simulink model "DYN_02x"  (R2021a)
(part 5 of 53)

[de2*((cos(e6)*(sin(e2 + e3)*sin(e5) - cos(e2 + e3)*cos(e4)*cos(e5)) + cos(e2 + e3)*sin(e4)*sin(e6))*(I6zx*(cos(e2 + e3)*cos(e5) - sin(e2 + e3)*cos(e4)*sin(e5)) + I6xx*(cos(e6)*(cos(e2 + e3)*sin(e5) + sin(e2 + e3)*cos(e4)*cos(e5)) - sin(e2 + e3)*sin(e4)*sin(e6)) - I6yx*(sin(e6)*(cos(e2 + e3)*sin(e5) + sin(e2 + e3)*cos(e4)*cos(e5)) + sin(e2 + e3)*cos(e6)*sin(e4))) - (sin(e6)*(sin(e2 + e3)*sin(e5) - cos(e2 + e3)*cos(e4)*cos(e5)) - cos(e2 + e3)*cos(e6)*sin(e4))*(I6zy*(cos(e2 + e3)*cos(e5) - sin(e2 + e3)*cos(e4)*sin(e5)) + I6xy*(cos(e6)*(cos(e2 + e3)*sin(e5) + sin(e2 + e3)*cos(e4)*cos(e5)) - sin(e2 + e3)*sin(e4)*sin(e6)) - I6yy*(sin(e6)*(cos(e2 + e3)*sin(e5) + sin(e2 + e3)*cos(e4)*cos(e5)) + sin(e2 + e3)*cos(e6)*sin(e4))) + (cos(e2 + e3)*sin(e5) + sin(e2 + e3)*cos(e4)*cos(e5))*(I5xx*(sin(e2 + e3)*sin(e5) - cos(e2 + e3)*cos(e4)*cos(e5)) + I5yx*(sin(e2 + e3)*cos(e5) + cos(e2 + e3)*cos(e4)*sin(e5)) - I5zx*cos(e2 + e3)*sin(e4)) + (cos(e2 + e3)*cos(e5) - sin(e2 + e3)*cos(e4)*sin(e5))*(I5xy*(sin(e2 + e3)*sin(e5) - cos(e2 + e3)*cos(e4)*cos(e5)) + I5yy*(sin(e2 + e3)*cos(e5) + cos(e2 + e3)*cos(e4)*sin(e5)) - I5zy*cos(e2 + e3)*sin(e4)) + (sin(e2 + e3)*sin(e5) - cos(e2 + e3)*cos(e4)*cos(e5))*(I5xx*(cos(e2 + e3)*sin(e5) + sin(e2 + e3)*cos(e4)*cos(e5)) + I5yx*(cos(e2 + e3)*cos(e5) - sin(e2 + e3)*cos(e4)*sin(e5)) + I5zx*sin(e2 + e3)*sin(e4)) + (sin(e2 + e3)*cos(e5) + cos(e2 + e3)*cos(e4)*sin(e5))*(I5xy*(cos(e2 + e3)*sin(e5) + sin(e2 + e3)*cos(e4)*cos(e5)) + I5yy*(cos(e2 + e3)*cos(e5) - sin(e2 + e3)*cos(e4)*sin(e5)) + I5zy*sin(e2 + e3)*sin(e4)) - cos(e2)*(I2yx*cos(e2) + I2xx*sin(e2)) - cos(e2)*(I2xy*cos(e2) - I2yy*sin(e2)) - sin(e2)*(I2xx*cos(e2) - I2yx*sin(e2)) + sin(e2)*(I2yy*cos(e2) + I2xy*sin(e2)) + cos(e2 + e3)*(I4zz*sin(e2 + e3) + I4yz*cos(e2 + e3)*sin(e4) - I4xz*cos(e2 + e3)*cos(e4)) + sin(e2 + e3)*(I4zz*cos(e2 + e3) + I4xz*sin(e2 + e3)*cos(e4) - I4yz*sin(e2 + e3)*sin(e4)) + (cos(e2 + e3)*cos(e5) - sin(e2 + e3)*cos(e4)*sin(e5))*(I6zz*(sin(e2 + e3)*cos(e5) + cos(e2 + e3)*cos(e4)*sin(e5)) + I6xz*(cos(e6)*(sin(e2 + e3)*sin(e5) - cos(e2 + e3)*cos(e4)*cos(e5)) + cos(e2 + e3)*sin(e4)*sin(e6)) - I6yz*(sin(e6)*(sin(e2 + e3)*sin(e5) - cos(e2 + e3)*cos(e4)*cos(e5)) - cos(e2 + e3)*cos(e6)*sin(e4))) - cos(e2 + e3)*(I3yx*cos(e2 + e3) + I3xx*sin(e2 + e3)) - cos(e2 + e3)*(I3xy*cos(e2 + e3) - I3yy*sin(e2 + e3)) - sin(e2 + e3)*(I3xx*cos(e2 + e3) - I3yx*sin(e2 + e3)) + sin(e2 + e3)*(I3yy*cos(e2 + e3) + I3xy*sin(e2 + e3)) + (sin(e2 + e3)*cos(e5) + cos(e2 + e3)*cos(e4)*sin(e5))*(I6zz*(cos(e2 + e3)*cos(e5) - sin(e2 + e3)*cos(e4)*sin(e5)) + I6xz*(cos(e6)*(cos(e2 + e3)*sin(e5) + sin(e2 + e3)*cos(e4)*cos(e5)) - sin(e2 + e3)*sin(e4)*sin(e6)) - I6yz*(sin(e6)*(cos(e2 + e3)*sin(e5) + sin(e2 + e3)*cos(e4)*cos(e5)) + sin(e2 + e3)*cos(e6)*sin(e4))) + (cos(e6)*(cos(e2 + e3)*sin(e5) + sin(e2 + e3)*cos(e4)*cos(e5)) - sin(e2 + e3)*sin(e4)*sin(e6))*(I6zx*(sin(e2 + e3)*cos(e5) + cos(e2 + e3)*cos(e4)*sin(e5)) + I6xx*(cos(e6)*(sin(e2 + e3)*sin(e5) - cos(e2 + e3)*cos(e4)*cos(e5)) + cos(e2 + e3)*sin(e4)*sin(e6)) - I6yx*(sin(e6)*(sin(e2 + e3)*sin(e5) - cos(e2 + e3)*cos(e4)*cos(e5)) - cos(e2 + e3)*cos(e6)*sin(e4))) - (sin(e6)*(cos(e2 + e3)*sin(e5) + sin(e2 + e3)*cos(e4)*cos(e5)) + sin(e2 + e3)*cos(e6)*sin(e4))*(I6zy*(sin(e2 + e3)*cos(e5) + cos(e2 + e3)*cos(e4)*sin(e5)) + I6xy*(cos(e6)*(sin(e2 + e3)*sin(e5) - cos(e2 + e3)*cos(e4)*cos(e5)) + cos(e2 + e3)*sin(e4)*sin(e6)) - I6yy*(sin(e6)*(sin(e2 + e3)*sin(e5) - cos(e2 + e3)*cos(e4)*cos(e5)) - cos(e2 + e3)*cos(e6)*sin(e4))) - 2*m6*((sin(e6)*(sin(e5)*(cos(e2)*cos(e3)*sin(e1) - sin(e1)*sin(e2)*sin(e3)) - cos(e5)*(cos(e1)*sin(e4) - cos(e4)*(cos(e2)*sin(e1)*sin(e3) + cos(e3)*sin(e1)*sin(e2)))) + cos(e6)*(sin(e4)*(cos(e2)*sin(e1)*sin(e3) + cos(e3)*sin(e1)*sin(e2)) + cos(e1)*cos(e4)))*(x6*(sin(e2 + e3)*cos(e5) + cos(e2 + e3)*cos(e4)*sin(e5)) - z6*(cos(e6)*(sin(e2 + e3)*sin(e5) - cos(e2 + e3)*cos(e4)*cos(e5)) + cos(e2 + e3)*sin(e4)*sin(e6)) + cos(e4)*cos(e6)*(a1 + d4*cos(e2 + e3) + a3*sin(e2 + e3) + a2*sin(e2)) - cos(e5)*sin(e4)*sin(e6)*(a1 + d4*cos(e2 + e3) + a3*sin(e2 + e3) + a2*sin(e2))) + (cos(e6)*(sin(e5)*(cos(e2)*cos(e3)*sin(e1) - sin(e1)*sin(e2)*sin(e3)) - cos(e5)*(cos(e1)*sin(e4) - cos(e4)*(cos(e2)*sin(e1)*sin(e3) + cos(e3)*sin(e1)*sin(e2)))) - sin(e6)*(sin(e4)*(cos(e2)*sin(e1)*sin(e3) + cos(e3)*sin(e1)*sin(e2)) + cos(e1)*cos(e4)))*(y6*(sin(e2 + e3)*cos(e5) + cos(e2 + e3)*cos(e4)*sin(e5)) + z6*(sin(e6)*(sin(e2 + e3)*sin(e5) - cos(e2 + e3)*cos(e4)*cos(e5)) - cos(e2 + e3)*cos(e6)*sin(e4)) - cos(e4)*sin(e6)*(a1 + d4*cos(e2 + e3) + a3*sin(e2 + e3) + a2*sin(e2)) - cos(e5)*cos(e6)*sin(e4)*(a1 + d4*cos(e2 + e3) + a3*sin(e2 + e3) + a2*sin(e2))) - (cos(e5)*(cos(e2)*cos(e3)*sin(e1) - sin(e1)*sin(e2)*sin(e3)) + sin(e5)*(cos(e1)*sin(e4) - cos(e4)*(cos(e2)*sin(e1)*sin(e3) + cos(e3)*sin(e1)*sin(e2))))*(x6*(sin(e6)*(sin(e2 + e3)*sin(e5) - cos(e2 + e3)*cos(e4)*cos(e5)) - cos(e2 + e3)*cos(e6)*sin(e4)) + y6*(cos(e6)*(sin(e2 + e3)*sin(e5) - cos(e2 + e3)*cos(e4)*cos(e5)) + cos(e2 + e3)*sin(e4)*sin(e6)) - sin(e4)*sin(e5)*(a1 + d4*cos(e2 + e3) + a3*sin(e2 + e3) + a2*sin(e2))))*((sin(e6)*(sin(e5)*(cos(e2)*sin(e1)*sin(e3) + cos(e3)*sin(e1)*sin(e2)) - cos(e4)*cos(e5)*(cos(e2)*cos(e3)*sin(e1) - sin(e1)*sin(e2)*sin(e3))) - cos(e6)*sin(e4)*(cos(e2)*cos(e3)*sin(e1) - sin(e1)*sin(e2)*sin(e3)))*(x6*(sin(e2 + e3)*cos(e5) + cos(e2 + e3)*cos(e4)*sin(e5)) - z6*(cos(e6)*(sin(e2 + e3)*sin(e5) - cos(e2 + e3)*cos(e4)*cos(e5)) + cos(e2 + e3)*sin(e4)*sin(e6)) + cos(e4)*cos(e6)*(a1 + d4*cos(e2 + e3) + a3*sin(e2 + e3) + a2*sin(e2)) - cos(e5)*sin(e4)*sin(e6)*(a1 + d4*cos(e2 + e3) + a3*sin(e2 + e3) + a2*sin(e2))) + (cos(e6)*(sin(e5)*(cos(e2)*sin(e1)*sin(e3) + cos(e3)*sin(e1)*sin(e2)) - cos(e4)*cos(e5)*(cos(e2)*cos(e3)*sin(e1) - sin(e1)*sin(e2)*sin(e3))) + sin(e4)*sin(e6)*(cos(e2)*cos(e3)*sin(e1) - sin(e1)*sin(e2)*sin(e3)))*(y6*(sin(e2 + e3)*cos(e5) + cos(e2 + e3)*cos(e4)*sin(e5)) + z6*(sin(e6)*(sin(e2 + e3)*sin(e5) - cos(e2 + e3)*cos(e4)*cos(e5)) - cos(e2 + e3)*cos(e6)*sin(e4)) - cos(e4)*sin(e6)*(a1 + d4*cos(e2 + e3) + a3*sin(e2 + e3) + a2*sin(e2)) - cos(e5)*cos(e6)*sin(e4)*(a1 + d4*cos(e2 + e3) + a3*sin(e2 + e3) + a2*sin(e2))) + (cos(e5)*(cos(e2)*cos(e3)*sin(e1) - sin(e1)*sin(e2)*sin(e3)) + sin(e5)*(cos(e1)*sin(e4) - cos(e4)*(cos(e2)*sin(e1)*sin(e3) + cos(e3)*sin(e1)*sin(e2))))*(x6*(sin(e6)*(cos(e2 + e3)*sin(e5) + sin(e2 + e3)*cos(e4)*cos(e5)) + sin(e2 + e3)*cos(e6)*sin(e4)) + y6*(cos(e6)*(cos(e2 + e3)*sin(e5) + sin(e2 + e3)*cos(e4)*cos(e5)) - sin(e2 + e3)*sin(e4)*sin(e6)) - sin(e4)*sin(e5)*(a3*cos(e2 + e3) - d4*sin(e2 + e3) + a2*cos(e2))) - (sin(e6)*(sin(e5)*(cos(e2)*cos(e3)*sin(e1) - sin(e1)*sin(e2)*sin(e3)) - cos(e5)*(cos(e1)*sin(e4) - cos(e4)*(cos(e2)*sin(e1)*sin(e3) + cos(e3)*sin(e1)*sin(e2)))) + cos(e6)*(sin(e4)*(cos(e2)*sin(e1)*sin(e3) + cos(e3)*sin(e1)*sin(e2)) + cos(e1)*cos(e4)))*(x6*(cos(e2 + e3)*cos(e5) - sin(e2 + e3)*cos(e4)*sin(e5)) - z6*(cos(e6)*(cos(e2 + e3)*sin(e5) + sin(e2 + e3)*cos(e4)*cos(e5)) - sin(e2 + e3)*sin(e4)*sin(e6)) + cos(e4)*cos(e6)*(a3*cos(e2 + e3) - d4*sin(e2 + e3) + a2*cos(e2)) - cos(e5)*sin(e4)*sin(e6)*(a3*cos(e2 + e3) - d4*sin(e2 + e3) + a2*cos(e2))) - (cos(e6)*(sin(e5)*(cos(e2)*cos(e3)*sin(e1) - sin(e1)*sin(e2)*sin(e3)) - cos(e5)*(cos(e1)*sin(e4) - cos(e4)*(cos(e2)*sin(e1)*sin(e3) + cos(e3)*sin(e1)*sin(e2)))) - sin(e6)*(sin(e4)*(cos(e2)*sin(e1)*sin(e3) + cos(e3)*sin(e1)*sin(e2)) + cos(e1)*cos(e4)))*(y6*(cos(e2 + e3)*cos(e5) - sin(e2 + e3)*cos(e4)*sin(e5)) + z6*(sin(e6)*(cos(e2 + e3)*sin(e5) + sin(e2 + e3)*cos(e4)*cos(e5)) + sin(e2 + e3)*cos(e6)*sin(e4)) - cos(e4)*sin(e6)*(a3*cos(e2 + e3) - d4*sin(e2 + e3) + a2*cos(e2)) - cos(e5)*cos(e6)*sin(e4)*(a3*cos(e2 + e3) - d4*sin(e2 + e3) + a2*cos(e2))) - (cos(e5)*(cos(e2)*sin(e1)*sin(e3) + cos(e3)*sin(e1)*sin(e2)) + cos(e4)*sin(e5)*(cos(e2)*cos(e3)*sin(e1) - sin(e1)*sin(e2)*sin(e3)))*(x6*(sin(e6)*(sin(e2 + e3)*sin(e5) - cos(e2 + e3)*cos(e4)*cos(e5)) - cos(e2 + e3)*cos(e6)*sin(e4)) + y6*(cos(e6)*(sin(e2 + e3)*sin(e5) - cos(e2 + e3)*cos(e4)*cos(e5)) + cos(e2 + e3)*sin(e4)*sin(e6)) - sin(e4)*sin(e5)*(a1 + d4*cos(e2 + e3) + a3*sin(e2 + e3) + a2*sin(e2)))) + 2*m5*((cos(e5)*(cos(e2)*sin(e3) + cos(e3)*sin(e2)) - cos(e4)*sin(e5)*(sin(e2)*sin(e3) - cos(e2)*cos(e3)))*(z5*(sin(e2 + e3)*sin(e5) - cos(e2 + e3)*cos(e4)*cos(e5)) + sin(e4)*sin(e5)*(a1 + d4*cos(e2 + e3) + a3*sin(e2 + e3) + a2*sin(e2)) + x5*cos(e2 + e3)*sin(e4)) - (sin(e5)*(cos(e2)*sin(e3) + cos(e3)*sin(e2)) + cos(e4)*cos(e5)*(sin(e2)*sin(e3) - cos(e2)*cos(e3)))*(z5*(sin(e2 + e3)*cos(e5) + cos(e2 + e3)*cos(e4)*sin(e5)) + cos(e5)*sin(e4)*(a1 + d4*cos(e2 + e3) + a3*sin(e2 + e3) + a2*sin(e2)) + y5*cos(e2 + e3)*sin(e4)) + sin(e4)*(sin(e2)*sin(e3) - cos(e2)*cos(e3))*(cos(e4)*(a1 + d4*cos(e2 + e3) + a3*sin(e2 + e3) + a2*sin(e2)) + x5*(sin(e2 + e3)*cos(e5) + cos(e2 + e3)*cos(e4)*sin(e5)) - y5*(sin(e2 + e3)*sin(e5) - cos(e2 + e3)*cos(e4)*cos(e5))))*((cos(e5)*(cos(e2)*sin(e3) + cos(e3)*sin(e2)) - cos(e4)*sin(e5)*(sin(e2)*sin(e3) - cos(e2)*cos(e3)))*(z5*(cos(e2 + e3)*sin(e5) + sin(e2 + e3)*cos(e4)*cos(e5)) - x5*sin(e2 + e3)*sin(e4) + sin(e4)*sin(e5)*(a3*cos(e2 + e3) - d4*sin(e2 + e3) + a2*cos(e2))) - (sin(e5)*(cos(e2)*sin(e3) + cos(e3)*sin(e2)) + cos(e4)*cos(e5)*(sin(e2)*sin(e3) - cos(e2)*cos(e3)))*(z5*(cos(e2 + e3)*cos(e5) - sin(e2 + e3)*cos(e4)*sin(e5)) - y5*sin(e2 + e3)*sin(e4) + cos(e5)*sin(e4)*(a3*cos(e2 + e3) - d4*sin(e2 + e3) + a2*cos(e2))) + (sin(e5)*(sin(e2)*sin(e3) - cos(e2)*cos(e3)) - cos(e4)*cos(e5)*(cos(e2)*sin(e3) + cos(e3)*sin(e2)))*(z5*(sin(e2 + e3)*cos(e5) + cos(e2 + e3)*cos(e4)*sin(e5)) + cos(e5)*sin(e4)*(a1 + d4*cos(e2 + e3) + a3*sin(e2 + e3) + a2*sin(e2)) + y5*cos(e2 + e3)*sin(e4)) - (cos(e5)*(sin(e2)*sin(e3) - cos(e2)*cos(e3)) + cos(e4)*sin(e5)*(cos(e2)*sin(e3) + cos(e3)*sin(e2)))*(z5*(sin(e2 + e3)*sin(e5) - cos(e2 + e3)*cos(e4)*cos(e5)) + sin(e4)*sin(e5)*(a1 + d4*cos(e2 + e3) + a3*sin(e2 + e3) + a2*sin(e2)) + x5*cos(e2 + e3)*sin(e4)) + sin(e4)*(cos(e2)*sin(e3) + cos(e3)*sin(e2))*(cos(e4)*(a1 + d4*cos(e2 + e3) + a3*sin(e2 + e3) + a2*sin(e2)) + x5*(sin(e2 + e3)*cos(e5) + cos(e2 + e3)*cos(e4)*sin(e5)) - y5*(sin(e2 + e3)*sin(e5) - cos(e2 + e3)*cos(e4)*cos(e5))) + sin(e4)*(sin(e2)*sin(e3) - cos(e2)*cos(e3))*(x5*(cos(e2 + e3)*cos(e5) - sin(e2 + e3)*cos(e4)*sin(e5)) - y5*(cos(e2 + e3)*sin(e5) + sin(e2 + e3)*cos(e4)*cos(e5)) + cos(e4)*(a3*cos(e2 + e3) - d4*sin(e2 + e3) + a2*cos(e2)))) - 2*m4*((cos(e2)*sin(e3) + cos(e3)*sin(e2))*(y4*cos(e2 + e3)*cos(e4) + x4*cos(e2 + e3)*sin(e4)) + sin(e4)*(sin(e2)*sin(e3) - cos(e2)*cos(e3))*(cos(e4)*(a1 + d4*cos(e2 + e3) + a3*sin(e2 + e3) + a2*sin(e2)) + x4*sin(e2 + e3) + z4*cos(e2 + e3)*cos(e4)) - cos(e4)*(sin(e2)*sin(e3) - cos(e2)*cos(e3))*(sin(e4)*(a1 + d4*cos(e2 + e3) + a3*sin(e2 + e3) + a2*sin(e2)) - y4*sin(e2 + e3) + z4*cos(e2 + e3)*sin(e4)))*((sin(e2)*sin(e3) - cos(e2)*cos(e3))*(y4*cos(e2 + e3)*cos(e4) + x4*cos(e2 + e3)*sin(e4)) + (cos(e2)*sin(e3) + cos(e3)*sin(e2))*(y4*sin(e2 + e3)*cos(e4) + x4*sin(e2 + e3)*sin(e4)) - sin(e4)*(sin(e2)*sin(e3) - cos(e2)*cos(e3))*(x4*cos(e2 + e3) + cos(e4)*(a3*cos(e2 + e3) - d4*sin(e2 + e3) + a2*cos(e2)) - z4*sin(e2 + e3)*cos(e4)) - cos(e4)*(sin(e2)*sin(e3) - cos(e2)*cos(e3))*(y4*cos(e2 + e3) - sin(e4)*(a3*cos(e2 + e3) - d4*sin(e2 + e3) + a2*cos(e2)) + z4*sin(e2 + e3)*sin(e4)) - sin(e4)*(cos(e2)*sin(e3) + cos(e3)*sin(e2))*(cos(e4)*(a1 + d4*cos(e2 + e3) + a3*sin(e2 + e3) + a2*sin(e2)) + x4*sin(e2 + e3) + z4*cos(e2 + e3)*cos(e4)) + cos(e4)*(cos(e2)*sin(e3) + cos(e3)*sin(e2))*(sin(e4)*(a1 + d4*cos(e2 + e3) + a3*sin(e2 + e3) + a2*sin(e2)) - y4*sin(e2 + e3) + z4*cos(e2 + e3)*sin(e4))) - 2*m6*((sin(e6)*(sin(e5)*(cos(e2)*sin(e3) + cos(e3)*sin(e2)) + cos(e4)*cos(e5)*(sin(e2)*sin(e3) - cos(e2)*cos(e3))) + cos(e6)*sin(e4)*(sin(e2)*sin(e3) - cos(e2)*cos(e3)))*(x6*(sin(e2 + e3)*cos(e5) + cos(e2 + e3)*cos(e4)*sin(e5)) - z6*(cos(e6)*(sin(e2 + e3)*sin(e5) - cos(e2 + e3)*cos(e4)*cos(e5)) + cos(e2 + e3)*sin(e4)*sin(e6)) + cos(e4)*cos(e6)*(a1 + d4*cos(e2 + e3) + a3*sin(e2 + e3) + a2*sin(e2)) - cos(e5)*sin(e4)*sin(e6)*(a1 + d4*cos(e2 + e3) + a3*sin(e2 + e3) + a2*sin(e2))) + (cos(e6)*(sin(e5)*(cos(e2)*sin(e3) + cos(e3)*sin(e2)) + cos(e4)*cos(e5)*(sin(e2)*sin(e3) - cos(e2)*cos(e3))) - sin(e4)*sin(e6)*(sin(e2)*sin(e3) - cos(e2)*cos(e3)))*(y6*(sin(e2 + e3)*cos(e5) + cos(e2 + e3)*cos(e4)*sin(e5)) + z6*(sin(e6)*(sin(e2 + e3)*sin(e5) - cos(e2 + e3)*cos(e4)*cos(e5)) - cos(e2 + e3)*cos(e6)*sin(e4)) - cos(e4)*sin(e6)*(a1 + d4*cos(e2 + e3) + a3*sin(e2 + e3) + a2*sin(e2)) - cos(e5)*cos(e6)*sin(e4)*(a1 + d4*cos(e2 + e3) + a3*sin(e2 + e3) + a2*sin(e2))) - (cos(e5)*(cos(e2)*sin(e3) + cos(e3)*sin(e2)) - cos(e4)*sin(e5)*(sin(e2)*sin(e3) - cos(e2)*cos(e3)))*(x6*(sin(e6)*(sin(e2 + e3)*sin(e5) - cos(e2 + e3)*cos(e4)*cos(e5)) - cos(e2 + e3)*cos(e6)*sin(e4)) + y6*(cos(e6)*(sin(e2 + e3)*sin(e5) - cos(e2 + e3)*cos(e4)*cos(e5)) + cos(e2 + e3)*sin(e4)*sin(e6)) - sin(e4)*sin(e5)*(a1 + d4*cos(e2 + e3) + a3*sin(e2 + e3) + a2*sin(e2))))*((sin(e6)*(sin(e5)*(sin(e2)*sin(e3) - cos(e2)*cos(e3)) - cos(e4)*cos(e5)*(cos(e2)*sin(e3) + cos(e3)*sin(e2))) - cos(e6)*sin(e4)*(cos(e2)*sin(e3) + cos(e3)*sin(e2)))*(x6*(sin(e2 + e3)*cos(e5) + cos(e2 + e3)*cos(e4)*sin(e5)) - z6*(cos(e6)*(sin(e2 + e3)*sin(e5) - cos(e2 + e3)*cos(e4)*cos(e5)) + cos(e2 + e3)*sin(e4)*sin(e6)) + cos(e4)*cos(e6)*(a1 + d4*cos(e2 + e3) + a3*sin(e2 + e3) + a2*sin(e2)) - cos(e5)*sin(e4)*sin(e6)*(a1 + d4*cos(e2 + e3) + a3*sin(e2 + e3) + a2*sin(e2))) + (cos(e6)*(sin(e5)*(sin(e2)*sin(e3) - cos(e2)*cos(e3)) - cos(e4)*cos(e5)*(cos(e2)*sin(e3) + cos(e3)*sin(e2))) + sin(e4)*sin(e6)*(cos(e2)*sin(e3) + cos(e3)*sin(e2)))*(y6*(sin(e2 + e3)*cos(e5) + cos(e2 + e3)*cos(e4)*sin(e5)) + z6*(sin(e6)*(sin(e2 + e3)*sin(e5) - cos(e2 + e3)*cos(e4)*cos(e5)) - cos(e2 + e3)*cos(e6)*sin(e4)) - cos(e4)*sin(e6)*(a1 + d4*cos(e2 + e3) + a3*sin(e2 + e3) + a2*sin(e2)) - cos(e5)*cos(e6)*sin(e4)*(a1 + d4*cos(e2 + e3) + a3*sin(e2 + e3) + a2*sin(e2))) + (cos(e5)*(cos(e2)*sin(e3) + cos(e3)*sin(e2)) - cos(e4)*sin(e5)*(sin(e2)*sin(e3) - cos(e2)*cos(e3)))*(x6*(sin(e6)*(cos(e2 + e3)*sin(e5) + sin(e2 + e3)*cos(e4)*cos(e5)) + sin(e2 + e3)*cos(e6)*sin(e4)) + y6*(cos(e6)*(cos(e2 + e3)*sin(e5) + sin(e2 + e3)*cos(e4)*cos(e5)) - sin(e2 + e3)*sin(e4)*sin(e6)) - sin(e4)*sin(e5)*(a3*cos(e2 + e3) - d4*sin(e2 + e3) + a2*cos(e2))) - (sin(e6)*(sin(e5)*(cos(e2)*sin(e3) + cos(e3)*sin(e2)) + cos(e4)*cos(e5)*(sin(e2)*sin(e3) - cos(e2)*cos(e3))) + cos(e6)*sin(e4)*(sin(e2)*sin(e3) - cos(e2)*cos(e3)))*(x6*(cos(e2 + e3)*cos(e5) - sin(e2 + e3)*cos(e4)*sin(e5)) - z6*(cos(e6)*(cos(e2 + e3)*sin(e5) + sin(e2 + e3)*cos(e4)*cos(e5)) - sin(e2 + e3)*sin(e4)*sin(e6)) + cos(e4)*cos(e6)*(a3*cos(e2 + e3) - d4*sin(e2 + e3) + a2*cos(e2)) - cos(e5)*sin(e4)*sin(e6)*(a3*cos(e2 + e3) - d4*sin(e2 + e3) + a2*cos(e2))) - (cos(e6)*(sin(e5)*(cos(e2)*sin(e3) + cos(e3)*sin(e2)) + cos(e4)*cos(e5)*(sin(e2)*sin(e3) - cos(e2)*cos(e3))) - sin(e4)*sin(e6)*(sin(e2)*sin(e3) - cos(e2)*cos(e3)))*(y6*(cos(e2 + e3)*cos(e5) - sin(e2 + e3)*cos(e4)*sin(e5)) + z6*(sin(e6)*(cos(e2 + e3)*sin(e5) + sin(e2 + e3)*cos(e4)*cos(e5)) + sin(e2 + e3)*cos(e6)*sin(e4)) - cos(e4)*sin(e6)*(a3*cos(e2 + e3) - d4*sin(e2 + e3) + a2*cos(e2)) - cos(e5)*cos(e6)*sin(e4)*(a3*cos(e2 + e3) - d4*sin(e2 + e3) + a2*cos(e2))) - (cos(e5)*(sin(e2)*sin(e3) - cos(e2)*cos(e3)) + cos(e4)*sin(e5)*(cos(e2)*sin(e3) + cos(e3)*sin(e2)))*(x6*(sin(e6)*(sin(e2 + e3)*sin(e5) - cos(e2 + e3)*cos(e4)*cos(e5)) - cos(e2 + e3)*cos(e6)*sin(e4)) + y6*(cos(e6)*(sin(e2 + e3)*sin(e5) - cos(e2 + e3)*cos(e4)*cos(e5)) + cos(e2 + e3)*sin(e4)*sin(e6)) - sin(e4)*sin(e5)*(a1 + d4*cos(e2 + e3) + a3*sin(e2 + e3) + a2*sin(e2)))) - 2*m4*((sin(e4)*(cos(e2)*sin(e1)*sin(e3) + cos(e3)*sin(e1)*sin(e2)) + cos(e1)*cos(e4))*(cos(e4)*(a1 + d4*cos(e2 + e3) + a3*sin(e2 + e3) + a2*sin(e2)) + x4*sin(e2 + e3) + z4*cos(e2 + e3)*cos(e4)) + (cos(e2)*cos(e3)*sin(e1) - sin(e1)*sin(e2)*sin(e3))*(y4*cos(e2 + e3)*cos(e4) + x4*cos(e2 + e3)*sin(e4)) + (cos(e1)*sin(e4) - cos(e4)*(cos(e2)*sin(e1)*sin(e3) + cos(e3)*sin(e1)*sin(e2)))*(sin(e4)*(a1 + d4*cos(e2 + e3) + a3*sin(e2 + e3) + a2*sin(e2)) - y4*sin(e2 + e3) + z4*cos(e2 + e3)*sin(e4)))*((cos(e2)*sin(e1)*sin(e3) + cos(e3)*sin(e1)*sin(e2))*(y4*cos(e2 + e3)*cos(e4) + x4*cos(e2 + e3)*sin(e4)) + (cos(e2)*cos(e3)*sin(e1) - sin(e1)*sin(e2)*sin(e3))*(y4*sin(e2 + e3)*cos(e4) + x4*sin(e2 + e3)*sin(e4)) - (sin(e4)*(cos(e2)*sin(e1)*sin(e3) + cos(e3)*sin(e1)*sin(e2)) + cos(e1)*cos(e4))*(x4*cos(e2 + e3) + cos(e4)*(a3*cos(e2 + e3) - d4*sin(e2 + e3) + a2*cos(e2)) - z4*sin(e2 + e3)*cos(e4)) + (cos(e1)*sin(e4) - cos(e4)*(cos(e2)*sin(e1)*sin(e3) + cos(e3)*sin(e1)*sin(e2)))*(y4*cos(e2 + e3) - sin(e4)*(a3*cos(e2 + e3) - d4*sin(e2 + e3) + a2*cos(e2)) + z4*sin(e2 + e3)*sin(e4)) - sin(e4)*(cos(e2)*cos(e3)*sin(e1) - sin(e1)*sin(e2)*sin(e3))*(cos(e4)*(a1 + d4*cos(e2 + e3) + a3*sin(e2 + e3) + a2*sin(e2)) + x4*sin(e2 + e3) + z4*cos(e2 + e3)*cos(e4)) + cos(e4)*(cos(e2)*cos(e3)*sin(e1) - sin(e1)*sin(e2)*sin(e3))*(sin(e4)*(a1 + d4*cos(e2 + e3) + a3*sin(e2 + e3) + a2*sin(e2)) - y4*sin(e2 + e3) + z4*cos(e2 + e3)*sin(e4))) + 2*m5*((cos(e4)*sin(e1) - sin(e4)*(cos(e1)*cos(e2)*sin(e3) + cos(e1)*cos(e3)*sin(e2)))*(cos(e4)*(a1 + d4*cos(e2 + e3) + a3*sin(e2 + e3) + a2*sin(e2)) + x5*(sin(e2 + e3)*cos(e5) + cos(e2 + e3)*cos(e4)*sin(e5)) - y5*(sin(e2 + e3)*sin(e5) - cos(e2 + e3)*cos(e4)*cos(e5))) + (sin(e5)*(cos(e1)*cos(e2)*cos(e3) - cos(e1)*sin(e2)*sin(e3)) + cos(e5)*(sin(e1)*sin(e4) + cos(e4)*(cos(e1)*cos(e2)*sin(e3) + cos(e1)*cos(e3)*sin(e2))))*(z5*(sin(e2 + e3)*cos(e5) + cos(e2 + e3)*cos(e4)*sin(e5)) + cos(e5)*sin(e4)*(a1 + d4*cos(e2 + e3) + a3*sin(e2 + e3) + a2*sin(e2)) + y5*cos(e2 + e3)*sin(e4)) - (cos(e5)*(cos(e1)*cos(e2)*cos(e3) - cos(e1)*sin(e2)*sin(e3)) - sin(e5)*(sin(e1)*sin(e4) + cos(e4)*(cos(e1)*cos(e2)*sin(e3) + cos(e1)*cos(e3)*sin(e2))))*(z5*(sin(e2 + e3)*sin(e5) - cos(e2 + e3)*cos(e4)*cos(e5)) + sin(e4)*sin(e5)*(a1 + d4*cos(e2 + e3) + a3*sin(e2 + e3) + a2*sin(e2)) + x5*cos(e2 + e3)*sin(e4)))*((cos(e5)*(cos(e1)*cos(e2)*sin(e3) + cos(e1)*cos(e3)*sin(e2)) + cos(e4)*sin(e5)*(cos(e1)*cos(e2)*cos(e3) - cos(e1)*sin(e2)*sin(e3)))*(z5*(sin(e2 + e3)*sin(e5) - cos(e2 + e3)*cos(e4)*cos(e5)) + sin(e4)*sin(e5)*(a1 + d4*cos(e2 + e3) + a3*sin(e2 + e3) + a2*sin(e2)) + x5*cos(e2 + e3)*sin(e4)) + (cos(e4)*sin(e1) - sin(e4)*(cos(e1)*cos(e2)*sin(e3) + cos(e1)*cos(e3)*sin(e2)))*(x5*(cos(e2 + e3)*cos(e5) - sin(e2 + e3)*cos(e4)*sin(e5)) - y5*(cos(e2 + e3)*sin(e5) + sin(e2 + e3)*cos(e4)*cos(e5)) + cos(e4)*(a3*cos(e2 + e3) - d4*sin(e2 + e3) + a2*cos(e2))) + (sin(e5)*(cos(e1)*cos(e2)*cos(e3) - cos(e1)*sin(e2)*sin(e3)) + cos(e5)*(sin(e1)*sin(e4) + cos(e4)*(cos(e1)*cos(e2)*sin(e3) + cos(e1)*cos(e3)*sin(e2))))*(z5*(cos(e2 + e3)*cos(e5) - sin(e2 + e3)*cos(e4)*sin(e5)) - y5*sin(e2 + e3)*sin(e4) + cos(e5)*sin(e4)*(a3*cos(e2 + e3) - d4*sin(e2 + e3) + a2*cos(e2))) - (cos(e5)*(cos(e1)*cos(e2)*cos(e3) - cos(e1)*sin(e2)*sin(e3)) - sin(e5)*(sin(e1)*sin(e4) + cos(e4)*(cos(e1)*cos(e2)*sin(e3) + cos(e1)*cos(e3)*sin(e2))))*(z5*(cos(e2 + e3)*sin(e5) + sin(e2 + e3)*cos(e4)*cos(e5)) - x5*sin(e2 + e3)*sin(e4) + sin(e4)*sin(e5)*(a3*cos(e2 + e3) - d4*sin(e2 + e3) + a2*cos(e2))) - (sin(e5)*(cos(e1)*cos(e2)*sin(e3) + cos(e1)*cos(e3)*sin(e2)) - cos(e4)*cos(e5)*(cos(e1)*cos(e2)*cos(e3) - cos(e1)*sin(e2)*sin(e3)))*(z5*(sin(e2 + e3)*cos(e5) + cos(e2 + e3)*cos(e4)*sin(e5)) + cos(e5)*sin(e4)*(a1 + d4*cos(e2 + e3) + a3*sin(e2 + e3) + a2*sin(e2)) + y5*cos(e2 + e3)*sin(e4)) - sin(e4)*(cos(e1)*cos(e2)*cos(e3) - cos(e1)*sin(e2)*sin(e3))*(cos(e4)*(a1 + d4*cos(e2 + e3) + a3*sin(e2 + e3) + a2*sin(e2)) + x5*(sin(e2 + e3)*cos(e5) + cos(e2 + e3)*cos(e4)*sin(e5)) - y5*(sin(e2 + e3)*sin(e5) - cos(e2 + e3)*cos(e4)*cos(e5)))) - cos(e2 + e3)*cos(e4)*(I4zx*cos(e2 + e3) + I4xx*sin(e2 + e3)*cos(e4) - I4yx*sin(e2 + e3)*sin(e4)) + sin(e2 + e3)*cos(e4)*(I4zx*sin(e2 + e3) + I4yx*cos(e2 + e3)*sin(e4) - I4xx*cos(e2 + e3)*cos(e4)) + 2*m4*((cos(e4)*sin(e1) - sin(e4)*(cos(e1)*cos(e2)*sin(e3) + cos(e1)*cos(e3)*sin(e2)))*(cos(e4)*(a1 + d4*cos(e2 + e3) + a3*sin(e2 + e3) + a2*sin(e2)) + x4*sin(e2 + e3) + z4*cos(e2 + e3)*cos(e4)) - (y4*cos(e2 + e3)*cos(e4) + x4*cos(e2 + e3)*sin(e4))*(cos(e1)*cos(e2)*cos(e3) - cos(e1)*sin(e2)*sin(e3)) + (sin(e1)*sin(e4) + cos(e4)*(cos(e1)*cos(e2)*sin(e3) + cos(e1)*cos(e3)*sin(e2)))*(sin(e4)*(a1 + d4*cos(e2 + e3) + a3*sin(e2 + e3) + a2*sin(e2)) - y4*sin(e2 + e3) + z4*cos(e2 + e3)*sin(e4)))*((y4*cos(e2 + e3)*cos(e4) + x4*cos(e2 + e3)*sin(e4))*(cos(e1)*cos(e2)*sin(e3) + cos(e1)*cos(e3)*sin(e2)) + (y4*sin(e2 + e3)*cos(e4) + x4*sin(e2 + e3)*sin(e4))*(cos(e1)*cos(e2)*cos(e3) - cos(e1)*sin(e2)*sin(e3)) + (cos(e4)*sin(e1) - sin(e4)*(cos(e1)*cos(e2)*sin(e3) + cos(e1)*cos(e3)*sin(e2)))*(x4*cos(e2 + e3) + cos(e4)*(a3*cos(e2 + e3) - d4*sin(e2 + e3) + a2*cos(e2)) - z4*sin(e2 + e3)*cos(e4)) - (sin(e1)*sin(e4) + cos(e4)*(cos(e1)*cos(e2)*sin(e3) + cos(e1)*cos(e3)*sin(e2)))*(y4*cos(e2 + e3) - sin(e4)*(a3*cos(e2 + e3) - d4*sin(e2 + e3) + a2*cos(e2)) + z4*sin(e2 + e3)*sin(e4)) - sin(e4)*(cos(e1)*cos(e2)*cos(e3) - cos(e1)*sin(e2)*sin(e3))*(cos(e4)*(a1 + d4*cos(e2 + e3) + a3*sin(e2 + e3) + a2*sin(e2)) + x4*sin(e2 + e3) + z4*cos(e2 + e3)*cos(e4)) + cos(e4)*(cos(e1)*cos(e2)*cos(e3) - cos(e1)*sin(e2)*sin(e3))*(sin(e4)*(a1 + d4*cos(e2 + e3) + a3*sin(e2 + e3) + a2*sin(e2)) - y4*sin(e2 + e3) + z4*cos(e2 + e3)*sin(e4))) + cos(e2 + e3)*sin(e4)*(I4zy*cos(e2 + e3) + I4xy*sin(e2 + e3)*cos(e4) - I4yy*sin(e2 + e3)*sin(e4)) - sin(e2 + e3)*sin(e4)*(I4zy*sin(e2 + e3) + I4yy*cos(e2 + e3)*sin(e4) - I4xy*cos(e2 + e3)*cos(e4)) - 2*m6*((sin(e6)*(sin(e5)*(cos(e1)*cos(e2)*cos(e3) - cos(e1)*sin(e2)*sin(e3)) + cos(e5)*(sin(e1)*sin(e4) + cos(e4)*(cos(e1)*cos(e2)*sin(e3) + cos(e1)*cos(e3)*sin(e2)))) - cos(e6)*(cos(e4)*sin(e1) - sin(e4)*(cos(e1)*cos(e2)*sin(e3) + cos(e1)*cos(e3)*sin(e2))))*(x6*(sin(e2 + e3)*cos(e5) + cos(e2 + e3)*cos(e4)*sin(e5)) - z6*(cos(e6)*(sin(e2 + e3)*sin(e5) - cos(e2 + e3)*cos(e4)*cos(e5)) + cos(e2 + e3)*sin(e4)*sin(e6)) + cos(e4)*cos(e6)*(a1 + d4*cos(e2 + e3) + a3*sin(e2 + e3) + a2*sin(e2)) - cos(e5)*sin(e4)*sin(e6)*(a1 + d4*cos(e2 + e3) + a3*sin(e2 + e3) + a2*sin(e2))) + (cos(e6)*(sin(e5)*(cos(e1)*cos(e2)*cos(e3) - cos(e1)*sin(e2)*sin(e3)) + cos(e5)*(sin(e1)*sin(e4) + cos(e4)*(cos(e1)*cos(e2)*sin(e3) + cos(e1)*cos(e3)*sin(e2)))) + sin(e6)*(cos(e4)*sin(e1) - sin(e4)*(cos(e1)*cos(e2)*sin(e3) + cos(e1)*cos(e3)*sin(e2))))*(y6*(sin(e2 + e3)*cos(e5) + cos(e2 + e3)*cos(e4)*sin(e5)) + z6*(sin(e6)*(sin(e2 + e3)*sin(e5) - cos(e2 + e3)*cos(e4)*cos(e5)) - cos(e2 + e3)*cos(e6)*sin(e4)) - cos(e4)*sin(e6)*(a1 + d4*cos(e2 + e3) + a3*sin(e2 + e3) + a2*sin(e2)) - cos(e5)*cos(e6)*sin(e4)*(a1 + d4*cos(e2 + e3) + a3*sin(e2 + e3) + a2*sin(e2))) - (cos(e5)*(cos(e1)*cos(e2)*cos(e3) - cos(e1)*sin(e2)*sin(e3)) - sin(e5)*(sin(e1)*sin(e4) + cos(e4)*(cos(e1)*cos(e2)*sin(e3) + cos(e1)*cos(e3)*sin(e2))))*(x6*(sin(e6)*(sin(e2 + e3)*sin(e5) - cos(e2 + e3)*cos(e4)*cos(e5)) - cos(e2 + e3)*cos(e6)*sin(e4)) + y6*(cos(e6)*(sin(e2 + e3)*sin(e5) - cos(e2 + e3)*cos(e4)*cos(e5)) + cos(e2 + e3)*sin(e4)*sin(e6)) - sin(e4)*sin(e5)*(a1 + d4*cos(e2 + e3) + a3*sin(e2 + e3) + a2*sin(e2))))*((cos(e5)*(cos(e1)*cos(e2)*cos(e3) - cos(e1)*sin(e2)*sin(e3)) - sin(e5)*(sin(e1)*sin(e4) + cos(e4)*(cos(e1)*cos(e2)*sin(e3) + cos(e1)*cos(e3)*sin(e2))))*(x6*(sin(e6)*(cos(e2 + e3)*sin(e5) + sin(e2 + e3)*cos(e4)*cos(e5)) + sin(e2 + e3)*cos(e6)*sin(e4)) + y6*(cos(e6)*(cos(e2 + e3)*sin(e5) + sin(e2 + e3)*cos(e4)*cos(e5)) - sin(e2 + e3)*sin(e4)*sin(e6)) - sin(e4)*sin(e5)*(a3*cos(e2 + e3) - d4*sin(e2 + e3) + a2*cos(e2))) - (sin(e6)*(sin(e5)*(cos(e1)*cos(e2)*cos(e3) - cos(e1)*sin(e2)*sin(e3)) + cos(e5)*(sin(e1)*sin(e4) + cos(e4)*(cos(e1)*cos(e2)*sin(e3) + cos(e1)*cos(e3)*sin(e2)))) - cos(e6)*(cos(e4)*sin(e1) - sin(e4)*(cos(e1)*cos(e2)*sin(e3) + cos(e1)*cos(e3)*sin(e2))))*(x6*(cos(e2 + e3)*cos(e5) - sin(e2 + e3)*cos(e4)*sin(e5)) - z6*(cos(e6)*(cos(e2 + e3)*sin(e5) + sin(e2 + e3)*cos(e4)*cos(e5)) - sin(e2 + e3)*sin(e4)*sin(e6)) + cos(e4)*cos(e6)*(a3*cos(e2 + e3) - d4*sin(e2 + e3) + a2*cos(e2)) - cos(e5)*sin(e4)*sin(e6)*(a3*cos(e2 + e3) - d4*sin(e2 + e3) + a2*cos(e2))) - (cos(e6)*(sin(e5)*(cos(e1)*cos(e2)*cos(e3) - cos(e1)*sin(e2)*sin(e3)) + cos(e5)*(sin(e1)*sin(e4) + cos(e4)*(cos(e1)*cos(e2)*sin(e3) + cos(e1)*cos(e3)*sin(e2)))) + sin(e6)*(cos(e4)*sin(e1) - sin(e4)*(cos(e1)*cos(e2)*sin(e3) + cos(e1)*cos(e3)*sin(e2))))*(y6*(cos(e2 + e3)*cos(e5) - sin(e2 + e3)*cos(e4)*sin(e5)) + z6*(sin(e6)*(cos(e2 + e3)*sin(e5) + sin(e2 + e3)*cos(e4)*cos(e5)) + sin(e2 + e3)*cos(e6)*sin(e4)) - cos(e4)*sin(e6)*(a3*cos(e2 + e3) - d4*sin(e2 + e3) + a2*cos(e2)) - cos(e5)*cos(e6)*sin(e4)*(a3*cos(e2 + e3) - d4*sin(e2 + e3) + a2*cos(e2))) - (cos(e5)*(cos(e1)*cos(e2)*sin(e3) + cos(e1)*cos(e3)*sin(e2)) + cos(e4)*sin(e5)*(cos(e1)*cos(e2)*cos(e3) - cos(e1)*sin(e2)*sin(e3)))*(x6*(sin(e6)*(sin(e2 + e3)*sin(e5) - cos(e2 + e3)*cos(e4)*cos(e5)) - cos(e2 + e3)*cos(e6)*sin(e4)) + y6*(cos(e6)*(sin(e2 + e3)*sin(e5) - cos(e2 + e3)*cos(e4)*cos(e5)) + cos(e2 + e3)*sin(e4)*sin(e6)) - sin(e4)*sin(e5)*(a1 + d4*cos(e2 + e3) + a3*sin(e2 + e3) + a2*sin(e2))) + (sin(e6)*(sin(e5)*(cos(e1)*cos(e2)*sin(e3) + cos(e1)*cos(e3)*sin(e2)) - cos(e4)*cos(e5)*(cos(e1)*cos(e2)*cos(e3) - cos(e1)*sin(e2)*sin(e3))) - cos(e6)*sin(e4)*(cos(e1)*cos(e2)*cos(e3) - cos(e1)*sin(e2)*sin(e3)))*(x6*(sin(e2 + e3)*cos(e5) + cos(e2 + e3)*cos(e4)*sin(e5)) - z6*(cos(e6)*(sin(e2 + e3)*sin(e5) - cos(e2 + e3)*cos(e4)*cos(e5)) + cos(e2 + e3)*sin(e4)*sin(e6)) + cos(e4)*cos(e6)*(a1 + d4*cos(e2 + e3) + a3*sin(e2 + e3) + a2*sin(e2)) - cos(e5)*sin(e4)*sin(e6)*(a1 + d4*cos(e2 + e3) + a3*sin(e2 + e3) + a2*sin(e2))) + (cos(e6)*(sin(e5)*(cos(e1)*cos(e2)*sin(e3) + cos(e1)*cos(e3)*sin(e2)) - cos(e4)*cos(e5)*(cos(e1)*cos(e2)*cos(e3) - cos(e1)*sin(e2)*sin(e3))) + sin(e4)*sin(e6)*(cos(e1)*cos(e2)*cos(e3) - cos(e1)*sin(e2)*sin(e3)))*(y6*(sin(e2 + e3)*cos(e5) + cos(e2 + e3)*cos(e4)*sin(e5)) + z6*(sin(e6)*(sin(e2 + e3)*sin(e5) - cos(e2 + e3)*cos(e4)*cos(e5)) - cos(e2 + e3)*cos(e6)*sin(e4)) - cos(e4)*sin(e6)*(a1 + d4*cos(e2 + e3) + a3*sin(e2 + e3) + a2*sin(e2)) - cos(e5)*cos(e6)*sin(e4)*(a1 + d4*cos(e2 + e3) + a3*sin(e2 + e3) + a2*sin(e2)))) + 2*m5*((cos(e5)*(cos(e2)*cos(e3)*sin(e1) - sin(e1)*sin(e2)*sin(e3)) + sin(e5)*(cos(e1)*sin(e4) - cos(e4)*(cos(e2)*sin(e1)*sin(e3) + cos(e3)*sin(e1)*sin(e2))))*(z5*(sin(e2 + e3)*sin(e5) - cos(e2 + e3)*cos(e4)*cos(e5)) + sin(e4)*sin(e5)*(a1 + d4*cos(e2 + e3) + a3*sin(e2 + e3) + a2*sin(e2)) + x5*cos(e2 + e3)*sin(e4)) + (sin(e4)*(cos(e2)*sin(e1)*sin(e3) + cos(e3)*sin(e1)*sin(e2)) + cos(e1)*cos(e4))*(cos(e4)*(a1 + d4*cos(e2 + e3) + a3*sin(e2 + e3) + a2*sin(e2)) + x5*(sin(e2 + e3)*cos(e5) + cos(e2 + e3)*cos(e4)*sin(e5)) - y5*(sin(e2 + e3)*sin(e5) - cos(e2 + e3)*cos(e4)*cos(e5))) - (sin(e5)*(cos(e2)*cos(e3)*sin(e1) - sin(e1)*sin(e2)*sin(e3)) - cos(e5)*(cos(e1)*sin(e4) - cos(e4)*(cos(e2)*sin(e1)*sin(e3) + cos(e3)*sin(e1)*sin(e2))))*(z5*(sin(e2 + e3)*cos(e5) + cos(e2 + e3)*cos(e4)*sin(e5)) + cos(e5)*sin(e4)*(a1 + d4*cos(e2 + e3) + a3*sin(e2 + e3) + a2*sin(e2)) + y5*cos(e2 + e3)*sin(e4)))*((sin(e4)*(cos(e2)*sin(e1)*sin(e3) + cos(e3)*sin(e1)*sin(e2)) + cos(e1)*cos(e4))*(x5*(cos(e2 + e3)*cos(e5) - sin(e2 + e3)*cos(e4)*sin(e5)) - y5*(cos(e2 + e3)*sin(e5) + sin(e2 + e3)*cos(e4)*cos(e5)) + cos(e4)*(a3*cos(e2 + e3) - d4*sin(e2 + e3) + a2*cos(e2))) + (sin(e5)*(cos(e2)*sin(e1)*sin(e3) + cos(e3)*sin(e1)*sin(e2)) - cos(e4)*cos(e5)*(cos(e2)*cos(e3)*sin(e1) - sin(e1)*sin(e2)*sin(e3)))*(z5*(sin(e2 + e3)*cos(e5) + cos(e2 + e3)*cos(e4)*sin(e5)) + cos(e5)*sin(e4)*(a1 + d4*cos(e2 + e3) + a3*sin(e2 + e3) + a2*sin(e2)) + y5*cos(e2 + e3)*sin(e4)) - (cos(e5)*(cos(e2)*sin(e1)*sin(e3) + cos(e3)*sin(e1)*sin(e2)) + cos(e4)*sin(e5)*(cos(e2)*cos(e3)*sin(e1) - sin(e1)*sin(e2)*sin(e3)))*(z5*(sin(e2 + e3)*sin(e5) - cos(e2 + e3)*cos(e4)*cos(e5)) + sin(e4)*sin(e5)*(a1 + d4*cos(e2 + e3) + a3*sin(e2 + e3) + a2*sin(e2)) + x5*cos(e2 + e3)*sin(e4)) - (sin(e5)*(cos(e2)*cos(e3)*sin(e1) - sin(e1)*sin(e2)*sin(e3)) - cos(e5)*(cos(e1)*sin(e4) - cos(e4)*(cos(e2)*sin(e1)*sin(e3) + cos(e3)*sin(e1)*sin(e2))))*(z5*(cos(e2 + e3)*cos(e5) - sin(e2 + e3)*cos(e4)*sin(e5)) - y5*sin(e2 + e3)*sin(e4) + cos(e5)*sin(e4)*(a3*cos(e2 + e3) - d4*sin(e2 + e3) + a2*cos(e2))) + (cos(e5)*(cos(e2)*cos(e3)*sin(e1) - sin(e1)*sin(e2)*sin(e3)) + sin(e5)*(cos(e1)*sin(e4) - cos(e4)*(cos(e2)*sin(e1)*sin(e3) + cos(e3)*sin(e1)*sin(e2))))*(z5*(cos(e2 + e3)*sin(e5) + sin(e2 + e3)*cos(e4)*cos(e5)) - x5*sin(e2 + e3)*sin(e4) + sin(e4)*sin(e5)*(a3*cos(e2 + e3) - d4*sin(e2 + e3) + a2*cos(e2))) + sin(e4)*(cos(e2)*cos(e3)*sin(e1) - sin(e1)*sin(e2)*sin(e3))*(cos(e4)*(a1 + d4*cos(e2 + e3) + a3*sin(e2 + e3) + a2*sin(e2)) + x5*(sin(e2 + e3)*cos(e5) + cos(e2 + e3)*cos(e4)*sin(e5)) - y5*(sin(e2 + e3)*sin(e5) - cos(e2 + e3)*cos(e4)*cos(e5)))) - cos(e2 + e3)*sin(e4)*(I5xz*(cos(e2 + e3)*sin(e5) + sin(e2 + e3)*cos(e4)*cos(e5)) + I5yz*(cos(e2 + e3)*cos(e5) - sin(e2 + e3)*cos(e4)*sin(e5)) + I5zz*sin(e2 + e3)*sin(e4)) + sin(e2 + e3)*sin(e4)*(I5xz*(sin(e2 + e3)*sin(e5) - cos(e2 + e3)*cos(e4)*cos(e5)) + I5yz*(sin(e2 + e3)*cos(e5) + cos(e2 + e3)*cos(e4)*sin(e5)) - I5zz*cos(e2 + e3)*sin(e4)) + 2*m3*sin(e1)*(x3*cos(e2 + e3) - y3*sin(e2 + e3) + a2*cos(e2))*(sin(e1)*(a1 + y3*cos(e2 + e3) + x3*sin(e2 + e3) + a2*sin(e2)) + z3*cos(e2 + e3)^2*cos(e1) + z3*sin(e2 + e3)^2*cos(e1)) - 2*m3*cos(e1)*(z3*cos(e2 + e3)^2*sin(e1) - cos(e1)*(a1 + y3*cos(e2 + e3) + x3*sin(e2 + e3) + a2*sin(e2)) + z3*sin(e2 + e3)^2*sin(e1))*(x3*cos(e2 + e3) - y3*sin(e2 + e3) + a2*cos(e2)) + 2*m2*sin(e1)*(x2*cos(e2) - y2*sin(e2))*(sin(e1)*(a1 + y2*cos(e2) + x2*sin(e2)) + z2*cos(e1)*cos(e2)^2 + z2*cos(e1)*sin(e2)^2) - 2*m2*cos(e1)*(x2*cos(e2) - y2*sin(e2))*(z2*cos(e2)^2*sin(e1) - cos(e1)*(a1 + y2*cos(e2) + x2*sin(e2)) + z2*sin(e1)*sin(e2)^2)) - de5*((sin(e2 + e3)*cos(e5) + cos(e2 + e3)*cos(e4)*sin(e5))*(I6zz*(sin(e2 + e3)*sin(e5) - cos(e2 + e3)*cos(e4)*cos(e5)) - I6xz*cos(e6)*(sin(e2 + e3)*cos(e5) + cos(e2 + e3)*cos(e4)*sin(e5)) + I6yz*sin(e6)*(sin(e2 + e3)*cos(e5) + cos(e2 + e3)*cos(e4)*sin(e5))) - (I5xx*(sin(e2 + e3)*cos(e5) + cos(e2 + e3)*cos(e4)*sin(e5)) - I5yx*(sin(e2 + e3)*sin(e5) - cos(e2 + e3)*cos(e4)*cos(e5)))*(sin(e2 + e3)*sin(e5) - cos(e2 + e3)*cos(e4)*cos(e5)) - (I5xy*(sin(e2 + e3)*cos(e5) + cos(e2 + e3)*cos(e4)*sin(e5)) - I5yy*(sin(e2 + e3)*sin(e5) - cos(e2 + e3)*cos(e4)*cos(e5)))*(sin(e2 + e3)*cos(e5) + cos(e2 + e3)*cos(e4)*sin(e5)) - (sin(e2 + e3)*cos(e5) + cos(e2 + e3)*cos(e4)*sin(e5))*(I5xx*(sin(e2 + e3)*sin(e5) - cos(e2 + e3)*cos(e4)*cos(e5)) + I5yx*(sin(e2 + e3)*cos(e5) + cos(e2 + e3)*cos(e4)*sin(e5)) - I5zx*cos(e2 + e3)*sin(e4)) + (sin(e2 + e3)*sin(e5) - cos(e2 + e3)*cos(e4)*cos(e5))*(I5xy*(sin(e2 + e3)*sin(e5) - cos(e2 + e3)*cos(e4)*cos(e5)) + I5yy*(sin(e2 + e3)*cos(e5) + cos(e2 + e3)*cos(e4)*sin(e5)) - I5zy*cos(e2 + e3)*sin(e4)) + (cos(e6)*(sin(e2 + e3)*sin(e5) - cos(e2 + e3)*cos(e4)*cos(e5)) + cos(e2 + e3)*sin(e4)*sin(e6))*(I6zx*(sin(e2 + e3)*sin(e5) - cos(e2 + e3)*cos(e4)*cos(e5)) - I6xx*cos(e6)*(sin(e2 + e3)*cos(e5) + cos(e2 + e3)*cos(e4)*sin(e5)) + I6yx*sin(e6)*(sin(e2 + e3)*cos(e5) + cos(e2 + e3)*cos(e4)*sin(e5))) - (sin(e6)*(sin(e2 + e3)*sin(e5) - cos(e2 + e3)*cos(e4)*cos(e5)) - cos(e2 + e3)*cos(e6)*sin(e4))*(I6zy*(sin(e2 + e3)*sin(e5) - cos(e2 + e3)*cos(e4)*cos(e5)) - I6xy*cos(e6)*(sin(e2 + e3)*cos(e5) + cos(e2 + e3)*cos(e4)*sin(e5)) + I6yy*sin(e6)*(sin(e2 + e3)*cos(e5) + cos(e2 + e3)*cos(e4)*sin(e5))) + (sin(e2 + e3)*sin(e5) - cos(e2 + e3)*cos(e4)*cos(e5))*(I6zz*(sin(e2 + e3)*cos(e5) + cos(e2 + e3)*cos(e4)*sin(e5)) + I6xz*(cos(e6)*(sin(e2 + e3)*sin(e5) - cos(e2 + e3)*cos(e4)*cos(e5)) + cos(e2 + e3)*sin(e4)*sin(e6)) - I6yz*(sin(e6)*(sin(e2 + e3)*sin(e5) - cos(e2 + e3)*cos(e4)*cos(e5)) - cos(e2 + e3)*cos(e6)*sin(e4))) + 2*m5*((cos(e5)*(cos(e2)*cos(e3)*sin(e1) - sin(e1)*sin(e2)*sin(e3)) + sin(e5)*(cos(e1)*sin(e4) - cos(e4)*(cos(e2)*sin(e1)*sin(e3) + cos(e3)*sin(e1)*sin(e2))))*(z5*(sin(e2 + e3)*sin(e5) - cos(e2 + e3)*cos(e4)*cos(e5)) + sin(e4)*sin(e5)*(a1 + d4*cos(e2 + e3) + a3*sin(e2 + e3) + a2*sin(e2)) + x5*cos(e2 + e3)*sin(e4)) + (sin(e4)*(cos(e2)*sin(e1)*sin(e3) + cos(e3)*sin(e1)*sin(e2)) + cos(e1)*cos(e4))*(cos(e4)*(a1 + d4*cos(e2 + e3) + a3*sin(e2 + e3) + a2*sin(e2)) + x5*(sin(e2 + e3)*cos(e5) + cos(e2 + e3)*cos(e4)*sin(e5)) - y5*(sin(e2 + e3)*sin(e5) - cos(e2 + e3)*cos(e4)*cos(e5))) - (sin(e5)*(cos(e2)*cos(e3)*sin(e1) - sin(e1)*sin(e2)*sin(e3)) - cos(e5)*(cos(e1)*sin(e4) - cos(e4)*(cos(e2)*sin(e1)*sin(e3) + cos(e3)*sin(e1)*sin(e2))))*(z5*(sin(e2 + e3)*cos(e5) + cos(e2 + e3)*cos(e4)*sin(e5)) + cos(e5)*sin(e4)*(a1 + d4*cos(e2 + e3) + a3*sin(e2 + e3) + a2*sin(e2)) + y5*cos(e2 + e3)*sin(e4)))*((sin(e5)*(cos(e2)*cos(e3)*sin(e1) - sin(e1)*sin(e2)*sin(e3)) - cos(e5)*(cos(e1)*sin(e4) - cos(e4)*(cos(e2)*sin(e1)*sin(e3) + cos(e3)*sin(e1)*sin(e2))))*(z5*(sin(e2 + e3)*sin(e5) - cos(e2 + e3)*cos(e4)*cos(e5)) + sin(e4)*sin(e5)*(a1 + d4*cos(e2 + e3) + a3*sin(e2 + e3) + a2*sin(e2)) + x5*cos(e2 + e3)*sin(e4)) + (x5*(sin(e2 + e3)*sin(e5) - cos(e2 + e3)*cos(e4)*cos(e5)) + y5*(sin(e2 + e3)*cos(e5) + cos(e2 + e3)*cos(e4)*sin(e5)))*(sin(e4)*(cos(e2)*sin(e1)*sin(e3) + cos(e3)*sin(e1)*sin(e2)) + cos(e1)*cos(e4)) - (cos(e5)*(cos(e2)*cos(e3)*sin(e1) - sin(e1)*sin(e2)*sin(e3)) + sin(e5)*(cos(e1)*sin(e4) - cos(e4)*(cos(e2)*sin(e1)*sin(e3) + cos(e3)*sin(e1)*sin(e2))))*(z5*(sin(e2 + e3)*cos(e5) + cos(e2 + e3)*cos(e4)*sin(e5)) + cos(e5)*sin(e4)*(a1 + d4*cos(e2 + e3) + a3*sin(e2 + e3) + a2*sin(e2))) - (z5*(sin(e2 + e3)*sin(e5) - cos(e2 + e3)*cos(e4)*cos(e5)) + sin(e4)*sin(e5)*(a1 + d4*cos(e2 + e3) + a3*sin(e2 + e3) + a2*sin(e2)))*(sin(e5)*(cos(e2)*cos(e3)*sin(e1) - sin(e1)*sin(e2)*sin(e3)) - cos(e5)*(cos(e1)*sin(e4) - cos(e4)*(cos(e2)*sin(e1)*sin(e3) + cos(e3)*sin(e1)*sin(e2)))) + (cos(e5)*(cos(e2)*cos(e3)*sin(e1) - sin(e1)*sin(e2)*sin(e3)) + sin(e5)*(cos(e1)*sin(e4) - cos(e4)*(cos(e2)*sin(e1)*sin(e3) + cos(e3)*sin(e1)*sin(e2))))*(z5*(sin(e2 + e3)*cos(e5) + cos(e2 + e3)*cos(e4)*sin(e5)) + cos(e5)*sin(e4)*(a1 + d4*cos(e2 + e3) + a3*sin(e2 + e3) + a2*sin(e2)) + y5*cos(e2 + e3)*sin(e4))) - 2*m6*((sin(e6)*(sin(e5)*(cos(e2)*cos(e3)*sin(e1) - sin(e1)*sin(e2)*sin(e3)) - cos(e5)*(cos(e1)*sin(e4) - cos(e4)*(cos(e2)*sin(e1)*sin(e3) + cos(e3)*sin(e1)*sin(e2)))) + cos(e6)*(sin(e4)*(cos(e2)*sin(e1)*sin(e3) + cos(e3)*sin(e1)*sin(e2)) + cos(e1)*cos(e4)))*(x6*(sin(e2 + e3)*cos(e5) + cos(e2 + e3)*cos(e4)*sin(e5)) - z6*(cos(e6)*(sin(e2 + e3)*sin(e5) - cos(e2 + e3)*cos(e4)*cos(e5)) + cos(e2 + e3)*sin(e4)*sin(e6)) + cos(e4)*cos(e6)*(a1 + d4*cos(e2 + e3) + a3*sin(e2 + e3) + a2*sin(e2)) - cos(e5)*sin(e4)*sin(e6)*(a1 + d4*cos(e2 + e3) + a3*sin(e2 + e3) + a2*sin(e2))) + (cos(e6)*(sin(e5)*(cos(e2)*cos(e3)*sin(e1) - sin(e1)*sin(e2)*sin(e3)) - cos(e5)*(cos(e1)*sin(e4) - cos(e4)*(cos(e2)*sin(e1)*sin(e3) + cos(e3)*sin(e1)*sin(e2)))) - sin(e6)*(sin(e4)*(cos(e2)*sin(e1)*sin(e3) + cos(e3)*sin(e1)*sin(e2)) + cos(e1)*cos(e4)))*(y6*(sin(e2 + e3)*cos(e5) + cos(e2 + e3)*cos(e4)*sin(e5)) + z6*(sin(e6)*(sin(e2 + e3)*sin(e5) - cos(e2 + e3)*cos(e4)*cos(e5)) - cos(e2 + e3)*cos(e6)*sin(e4)) - cos(e4)*sin(e6)*(a1 + d4*cos(e2 + e3) + a3*sin(e2 + e3) + a2*sin(e2)) - cos(e5)*cos(e6)*sin(e4)*(a1 + d4*cos(e2 + e3) + a3*sin(e2 + e3) + a2*sin(e2))) - (cos(e5)*(cos(e2)*cos(e3)*sin(e1) - sin(e1)*sin(e2)*sin(e3)) + sin(e5)*(cos(e1)*sin(e4) - cos(e4)*(cos(e2)*sin(e1)*sin(e3) + cos(e3)*sin(e1)*sin(e2))))*(x6*(sin(e6)*(sin(e2 + e3)*sin(e5) - cos(e2 + e3)*cos(e4)*cos(e5)) - cos(e2 + e3)*cos(e6)*sin(e4)) + y6*(cos(e6)*(sin(e2 + e3)*sin(e5) - cos(e2 + e3)*cos(e4)*cos(e5)) + cos(e2 + e3)*sin(e4)*sin(e6)) - sin(e4)*sin(e5)*(a1 + d4*cos(e2 + e3) + a3*sin(e2 + e3) + a2*sin(e2))))*((cos(e6)*(sin(e5)*(cos(e2)*cos(e3)*sin(e1) - sin(e1)*sin(e2)*sin(e3)) - cos(e5)*(cos(e1)*sin(e4) - cos(e4)*(cos(e2)*sin(e1)*sin(e3) + cos(e3)*sin(e1)*sin(e2)))) - sin(e6)*(sin(e4)*(cos(e2)*sin(e1)*sin(e3) + cos(e3)*sin(e1)*sin(e2)) + cos(e1)*cos(e4)))*(z6*sin(e6)*(sin(e2 + e3)*cos(e5) + cos(e2 + e3)*cos(e4)*sin(e5)) - y6*(sin(e2 + e3)*sin(e5) - cos(e2 + e3)*cos(e4)*cos(e5)) + cos(e6)*sin(e4)*sin(e5)*(a1 + d4*cos(e2 + e3) + a3*sin(e2 + e3) + a2*sin(e2))) - (sin(e6)*(sin(e5)*(cos(e2)*cos(e3)*sin(e1) - sin(e1)*sin(e2)*sin(e3)) - cos(e5)*(cos(e1)*sin(e4) - cos(e4)*(cos(e2)*sin(e1)*sin(e3) + cos(e3)*sin(e1)*sin(e2)))) + cos(e6)*(sin(e4)*(cos(e2)*sin(e1)*sin(e3) + cos(e3)*sin(e1)*sin(e2)) + cos(e1)*cos(e4)))*(x6*(sin(e2 + e3)*sin(e5) - cos(e2 + e3)*cos(e4)*cos(e5)) + z6*cos(e6)*(sin(e2 + e3)*cos(e5) + cos(e2 + e3)*cos(e4)*sin(e5)) - sin(e4)*sin(e5)*sin(e6)*(a1 + d4*cos(e2 + e3) + a3*sin(e2 + e3) + a2*sin(e2))) + (sin(e5)*(cos(e2)*cos(e3)*sin(e1) - sin(e1)*sin(e2)*sin(e3)) - cos(e5)*(cos(e1)*sin(e4) - cos(e4)*(cos(e2)*sin(e1)*sin(e3) + cos(e3)*sin(e1)*sin(e2))))*(x6*(sin(e6)*(sin(e2 + e3)*sin(e5) - cos(e2 + e3)*cos(e4)*cos(e5)) - cos(e2 + e3)*cos(e6)*sin(e4)) + y6*(cos(e6)*(sin(e2 + e3)*sin(e5) - cos(e2 + e3)*cos(e4)*cos(e5)) + cos(e2 + e3)*sin(e4)*sin(e6)) - sin(e4)*sin(e5)*(a1 + d4*cos(e2 + e3) + a3*sin(e2 + e3) + a2*sin(e2))) - (cos(e5)*(cos(e2)*cos(e3)*sin(e1) - sin(e1)*sin(e2)*sin(e3)) + sin(e5)*(cos(e1)*sin(e4) - cos(e4)*(cos(e2)*sin(e1)*sin(e3) + cos(e3)*sin(e1)*sin(e2))))*(y6*cos(e6)*(sin(e2 + e3)*cos(e5) + cos(e2 + e3)*cos(e4)*sin(e5)) - cos(e5)*sin(e4)*(a1 + d4*cos(e2 + e3) + a3*sin(e2 + e3) + a2*sin(e2)) + x6*sin(e6)*(sin(e2 + e3)*cos(e5) + cos(e2 + e3)*cos(e4)*sin(e5))) + sin(e6)*(cos(e5)*(cos(e2)*cos(e3)*sin(e1) - sin(e1)*sin(e2)*sin(e3)) + sin(e5)*(cos(e1)*sin(e4) - cos(e4)*(cos(e2)*sin(e1)*sin(e3) + cos(e3)*sin(e1)*sin(e2))))*(x6*(sin(e2 + e3)*cos(e5) + cos(e2 + e3)*cos(e4)*sin(e5)) - z6*(cos(e6)*(sin(e2 + e3)*sin(e5) - cos(e2 + e3)*cos(e4)*cos(e5)) + cos(e2 + e3)*sin(e4)*sin(e6)) + cos(e4)*cos(e6)*(a1 + d4*cos(e2 + e3) + a3*sin(e2 + e3) + a2*sin(e2)) - cos(e5)*sin(e4)*sin(e6)*(a1 + d4*cos(e2 + e3) + a3*sin(e2 + e3) + a2*sin(e2))) + cos(e6)*(cos(e5)*(cos(e2)*cos(e3)*sin(e1) - sin(e1)*sin(e2)*sin(e3)) + sin(e5)*(cos(e1)*sin(e4) - cos(e4)*(cos(e2)*sin(e1)*sin(e3) + cos(e3)*sin(e1)*sin(e2))))*(y6*(sin(e2 + e3)*cos(e5) + cos(e2 + e3)*cos(e4)*sin(e5)) + z6*(sin(e6)*(sin(e2 + e3)*sin(e5) - cos(e2 + e3)*cos(e4)*cos(e5)) - cos(e2 + e3)*cos(e6)*sin(e4)) - cos(e4)*sin(e6)*(a1 + d4*cos(e2 + e3) + a3*sin(e2 + e3) + a2*sin(e2)) - cos(e5)*cos(e6)*sin(e4)*(a1 + d4*cos(e2 + e3) + a3*sin(e2 + e3) + a2*sin(e2)))) - 2*m6*((sin(e6)*(sin(e5)*(cos(e1)*cos(e2)*cos(e3) - cos(e1)*sin(e2)*sin(e3)) + cos(e5)*(sin(e1)*sin(e4) + cos(e4)*(cos(e1)*cos(e2)*sin(e3) + cos(e1)*cos(e3)*sin(e2)))) - cos(e6)*(cos(e4)*sin(e1) - sin(e4)*(cos(e1)*cos(e2)*sin(e3) + cos(e1)*cos(e3)*sin(e2))))*(x6*(sin(e2 + e3)*cos(e5) + cos(e2 + e3)*cos(e4)*sin(e5)) - z6*(cos(e6)*(sin(e2 + e3)*sin(e5) - cos(e2 + e3)*cos(e4)*cos(e5)) + cos(e2 + e3)*sin(e4)*sin(e6)) + cos(e4)*cos(e6)*(a1 + d4*cos(e2 + e3) + a3*sin(e2 + e3) + a2*sin(e2)) - cos(e5)*sin(e4)*sin(e6)*(a1 + d4*cos(e2 + e3) + a3*sin(e2 + e3) + a2*sin(e2))) + (cos(e6)*(sin(e5)*(cos(e1)*cos(e2)*cos(e3) - cos(e1)*sin(e2)*sin(e3)) + cos(e5)*(sin(e1)*sin(e4) + cos(e4)*(cos(e1)*cos(e2)*sin(e3) + cos(e1)*cos(e3)*sin(e2)))) + sin(e6)*(cos(e4)*sin(e1) - sin(e4)*(cos(e1)*cos(e2)*sin(e3) + cos(e1)*cos(e3)*sin(e2))))*(y6*(sin(e2 + e3)*cos(e5) + cos(e2 + e3)*cos(e4)*sin(e5)) + z6*(sin(e6)*(sin(e2 + e3)*sin(e5) - cos(e2 + e3)*cos(e4)*cos(e5)) - cos(e2 + e3)*cos(e6)*sin(e4)) - cos(e4)*sin(e6)*(a1 + d4*cos(e2 + e3) + a3*sin(e2 + e3) + a2*sin(e2)) - cos(e5)*cos(e6)*sin(e4)*(a1 + d4*cos(e2 + e3) + a3*sin(e2 + e3) + a2*sin(e2))) - (cos(e5)*(cos(e1)*cos(e2)*cos(e3) - cos(e1)*sin(e2)*sin(e3)) - sin(e5)*(sin(e1)*sin(e4) + cos(e4)*(cos(e1)*cos(e2)*sin(e3) + cos(e1)*cos(e3)*sin(e2))))*(x6*(sin(e6)*(sin(e2 + e3)*sin(e5) - cos(e2 + e3)*cos(e4)*cos(e5)) - cos(e2 + e3)*cos(e6)*sin(e4)) + y6*(cos(e6)*(sin(e2 + e3)*sin(e5) - cos(e2 + e3)*cos(e4)*cos(e5)) + cos(e2 + e3)*sin(e4)*sin(e6)) - sin(e4)*sin(e5)*(a1 + d4*cos(e2 + e3) + a3*sin(e2 + e3) + a2*sin(e2))))*((cos(e6)*(sin(e5)*(cos(e1)*cos(e2)*cos(e3) - cos(e1)*sin(e2)*sin(e3)) + cos(e5)*(sin(e1)*sin(e4) + cos(e4)*(cos(e1)*cos(e2)*sin(e3) + cos(e1)*cos(e3)*sin(e2)))) + sin(e6)*(cos(e4)*sin(e1) - sin(e4)*(cos(e1)*cos(e2)*sin(e3) + cos(e1)*cos(e3)*sin(e2))))*(z6*sin(e6)*(sin(e2 + e3)*cos(e5) + cos(e2 + e3)*cos(e4)*sin(e5)) - y6*(sin(e2 + e3)*sin(e5) - cos(e2 + e3)*cos(e4)*cos(e5)) + cos(e6)*sin(e4)*sin(e5)*(a1 + d4*cos(e2 + e3) + a3*sin(e2 + e3) + a2*sin(e2))) - (sin(e6)*(sin(e5)*(cos(e1)*cos(e2)*cos(e3) - cos(e1)*sin(e2)*sin(e3)) + cos(e5)*(sin(e1)*sin(e4) + cos(e4)*(cos(e1)*cos(e2)*sin(e3) + cos(e1)*cos(e3)*sin(e2)))) - cos(e6)*(cos(e4)*sin(e1) - sin(e4)*(cos(e1)*cos(e2)*sin(e3) + cos(e1)*cos(e3)*sin(e2))))*(x6*(sin(e2 + e3)*sin(e5) - cos(e2 + e3)*cos(e4)*cos(e5)) + z6*cos(e6)*(sin(e2 + e3)*cos(e5) + cos(e2 + e3)*cos(e4)*sin(e5)) - sin(e4)*sin(e5)*sin(e6)*(a1 + d4*cos(e2 + e3) + a3*sin(e2 + e3) + a2*sin(e2))) + (sin(e5)*(cos(e1)*cos(e2)*cos(e3) - cos(e1)*sin(e2)*sin(e3)) + cos(e5)*(sin(e1)*sin(e4) + cos(e4)*(cos(e1)*cos(e2)*sin(e3) + cos(e1)*cos(e3)*sin(e2))))*(x6*(sin(e6)*(sin(e2 + e3)*sin(e5) - cos(e2 + e3)*cos(e4)*cos(e5)) - cos(e2 + e3)*cos(e6)*sin(e4)) + y6*(cos(e6)*(sin(e2 + e3)*sin(e5) - cos(e2 + e3)*cos(e4)*cos(e5)) + cos(e2 + e3)*sin(e4)*sin(e6)) - sin(e4)*sin(e5)*(a1 + d4*cos(e2 + e3) + a3*sin(e2 + e3) + a2*sin(e2))) - (cos(e5)*(cos(e1)*cos(e2)*cos(e3) - cos(e1)*sin(e2)*sin(e3)) - sin(e5)*(sin(e1)*sin(e4) + cos(e4)*(cos(e1)*cos(e2)*sin(e3) + cos(e1)*cos(e3)*sin(e2))))*(y6*cos(e6)*(sin(e2 + e3)*cos(e5) + cos(e2 + e3)*cos(e4)*sin(e5)) - cos(e5)*sin(e4)*(a1 + d4*cos(e2 + e3) + a3*sin(e2 + e3) + a2*sin(e2)) + x6*sin(e6)*(sin(e2 + e3)*cos(e5) + cos(e2 + e3)*cos(e4)*sin(e5))) + cos(e6)*(cos(e5)*(cos(e1)*cos(e2)*cos(e3) - cos(e1)*sin(e2)*sin(e3)) - sin(e5)*(sin(e1)*sin(e4) + cos(e4)*(cos(e1)*cos(e2)*sin(e3) + cos(e1)*cos(e3)*sin(e2))))*(y6*(sin(e2 + e3)*cos(e5) + cos(e2 + e3)*cos(e4)*sin(e5)) + z6*(sin(e6)*(sin(e2 + e3)*sin(e5) - cos(e2 + e3)*cos(e4)*cos(e5)) - cos(e2 + e3)*cos(e6)*sin(e4)) - cos(e4)*sin(e6)*(a1 + d4*cos(e2 + e3) + a3*sin(e2 + e3) + a2*sin(e2)) - cos(e5)*cos(e6)*sin(e4)*(a1 + d4*cos(e2 + e3) + a3*sin(e2 + e3) + a2*sin(e2))) + sin(e6)*(cos(e5)*(cos(e1)*cos(e2)*cos(e3) - cos(e1)*sin(e2)*sin(e3)) - sin(e5)*(sin(e1)*sin(e4) + cos(e4)*(cos(e1)*cos(e2)*sin(e3) + cos(e1)*cos(e3)*sin(e2))))*(x6*(sin(e2 + e3)*cos(e5) + cos(e2 + e3)*cos(e4)*sin(e5)) - z6*(cos(e6)*(sin(e2 + e3)*sin(e5) - cos(e2 + e3)*cos(e4)*cos(e5)) + cos(e2 + e3)*sin(e4)*sin(e6)) + cos(e4)*cos(e6)*(a1 + d4*cos(e2 + e3) + a3*sin(e2 + e3) + a2*sin(e2)) - cos(e5)*sin(e4)*sin(e6)*(a1 + d4*cos(e2 + e3) + a3*sin(e2 + e3) + a2*sin(e2)))) + 2*m5*((cos(e5)*(cos(e2)*sin(e3) + cos(e3)*sin(e2)) - cos(e4)*sin(e5)*(sin(e2)*sin(e3) - cos(e2)*cos(e3)))*(z5*(sin(e2 + e3)*sin(e5) - cos(e2 + e3)*cos(e4)*cos(e5)) + sin(e4)*sin(e5)*(a1 + d4*cos(e2 + e3) + a3*sin(e2 + e3) + a2*sin(e2)) + x5*cos(e2 + e3)*sin(e4)) - (sin(e5)*(cos(e2)*sin(e3) + cos(e3)*sin(e2)) + cos(e4)*cos(e5)*(sin(e2)*sin(e3) - cos(e2)*cos(e3)))*(z5*(sin(e2 + e3)*cos(e5) + cos(e2 + e3)*cos(e4)*sin(e5)) + cos(e5)*sin(e4)*(a1 + d4*cos(e2 + e3) + a3*sin(e2 + e3) + a2*sin(e2)) + y5*cos(e2 + e3)*sin(e4)) + sin(e4)*(sin(e2)*sin(e3) - cos(e2)*cos(e3))*(cos(e4)*(a1 + d4*cos(e2 + e3) + a3*sin(e2 + e3) + a2*sin(e2)) + x5*(sin(e2 + e3)*cos(e5) + cos(e2 + e3)*cos(e4)*sin(e5)) - y5*(sin(e2 + e3)*sin(e5) - cos(e2 + e3)*cos(e4)*cos(e5))))*((cos(e5)*(cos(e2)*sin(e3) + cos(e3)*sin(e2)) - cos(e4)*sin(e5)*(sin(e2)*sin(e3) - cos(e2)*cos(e3)))*(z5*(sin(e2 + e3)*cos(e5) + cos(e2 + e3)*cos(e4)*sin(e5)) + cos(e5)*sin(e4)*(a1 + d4*cos(e2 + e3) + a3*sin(e2 + e3) + a2*sin(e2)) + y5*cos(e2 + e3)*sin(e4)) - (z5*(sin(e2 + e3)*sin(e5) - cos(e2 + e3)*cos(e4)*cos(e5)) + sin(e4)*sin(e5)*(a1 + d4*cos(e2 + e3) + a3*sin(e2 + e3) + a2*sin(e2)))*(sin(e5)*(cos(e2)*sin(e3) + cos(e3)*sin(e2)) + cos(e4)*cos(e5)*(sin(e2)*sin(e3) - cos(e2)*cos(e3))) - (cos(e5)*(cos(e2)*sin(e3) + cos(e3)*sin(e2)) - cos(e4)*sin(e5)*(sin(e2)*sin(e3) - cos(e2)*cos(e3)))*(z5*(sin(e2 + e3)*cos(e5) + cos(e2 + e3)*cos(e4)*sin(e5)) + cos(e5)*sin(e4)*(a1 + d4*cos(e2 + e3) + a3*sin(e2 + e3) + a2*sin(e2))) + (sin(e5)*(cos(e2)*sin(e3) + cos(e3)*sin(e2)) + cos(e4)*cos(e5)*(sin(e2)*sin(e3) - cos(e2)*cos(e3)))*(z5*(sin(e2 + e3)*sin(e5) - cos(e2 + e3)*cos(e4)*cos(e5)) + sin(e4)*sin(e5)*(a1 + d4*cos(e2 + e3) + a3*sin(e2 + e3) + a2*sin(e2)) + x5*cos(e2 + e3)*sin(e4)) + sin(e4)*(sin(e2)*sin(e3) - cos(e2)*cos(e3))*(x5*(sin(e2 + e3)*sin(e5) - cos(e2 + e3)*cos(e4)*cos(e5)) + y5*(sin(e2 + e3)*cos(e5) + cos(e2 + e3)*cos(e4)*sin(e5)))) - cos(e6)*(sin(e2 + e3)*cos(e5) + cos(e2 + e3)*cos(e4)*sin(e5))*(I6zx*(sin(e2 + e3)*cos(e5) + cos(e2 + e3)*cos(e4)*sin(e5)) + I6xx*(cos(e6)*(sin(e2 + e3)*sin(e5) - cos(e2 + e3)*cos(e4)*cos(e5)) + cos(e2 + e3)*sin(e4)*sin(e6)) - I6yx*(sin(e6)*(sin(e2 + e3)*sin(e5) - cos(e2 + e3)*cos(e4)*cos(e5)) - cos(e2 + e3)*cos(e6)*sin(e4))) + sin(e6)*(sin(e2 + e3)*cos(e5) + cos(e2 + e3)*cos(e4)*sin(e5))*(I6zy*(sin(e2 + e3)*cos(e5) + cos(e2 + e3)*cos(e4)*sin(e5)) + I6xy*(cos(e6)*(sin(e2 + e3)*sin(e5) - cos(e2 + e3)*cos(e4)*cos(e5)) + cos(e2 + e3)*sin(e4)*sin(e6)) - I6yy*(sin(e6)*(sin(e2 + e3)*sin(e5) - cos(e2 + e3)*cos(e4)*cos(e5)) - cos(e2 + e3)*cos(e6)*sin(e4))) - 2*m6*((sin(e6)*(sin(e5)*(cos(e2)*sin(e3) + cos(e3)*sin(e2)) + cos(e4)*cos(e5)*(sin(e2)*sin(e3) - cos(e2)*cos(e3))) + cos(e6)*sin(e4)*(sin(e2)*sin(e3) - cos(e2)*cos(e3)))*(x6*(sin(e2 + e3)*cos(e5) + cos(e2 + e3)*cos(e4)*sin(e5)) - z6*(cos(e6)*(sin(e2 + e3)*sin(e5) - cos(e2 + e3)*cos(e4)*cos(e5)) + cos(e2 + e3)*sin(e4)*sin(e6)) + cos(e4)*cos(e6)*(a1 + d4*cos(e2 + e3) + a3*sin(e2 + e3) + a2*sin(e2)) - cos(e5)*sin(e4)*sin(e6)*(a1 + d4*cos(e2 + e3) + a3*sin(e2 + e3) + a2*sin(e2))) + (cos(e6)*(sin(e5)*(cos(e2)*sin(e3) + cos(e3)*sin(e2)) + cos(e4)*cos(e5)*(sin(e2)*sin(e3) - cos(e2)*cos(e3))) - sin(e4)*sin(e6)*(sin(e2)*sin(e3) - cos(e2)*cos(e3)))*(y6*(sin(e2 + e3)*cos(e5) + cos(e2 + e3)*cos(e4)*sin(e5)) + z6*(sin(e6)*(sin(e2 + e3)*sin(e5) - cos(e2 + e3)*cos(e4)*cos(e5)) - cos(e2 + e3)*cos(e6)*sin(e4)) - cos(e4)*sin(e6)*(a1 + d4*cos(e2 + e3) + a3*sin(e2 + e3) + a2*sin(e2)) - cos(e5)*cos(e6)*sin(e4)*(a1 + d4*cos(e2 + e3) + a3*sin(e2 + e3) + a2*sin(e2))) - (cos(e5)*(cos(e2)*sin(e3) + cos(e3)*sin(e2)) - cos(e4)*sin(e5)*(sin(e2)*sin(e3) - cos(e2)*cos(e3)))*(x6*(sin(e6)*(sin(e2 + e3)*sin(e5) - cos(e2 + e3)*cos(e4)*cos(e5)) - cos(e2 + e3)*cos(e6)*sin(e4)) + y6*(cos(e6)*(sin(e2 + e3)*sin(e5) - cos(e2 + e3)*cos(e4)*cos(e5)) + cos(e2 + e3)*sin(e4)*sin(e6)) - sin(e4)*sin(e5)*(a1 + d4*cos(e2 + e3) + a3*sin(e2 + e3) + a2*sin(e2))))*((sin(e5)*(cos(e2)*sin(e3) + cos(e3)*sin(e2)) + cos(e4)*cos(e5)*(sin(e2)*sin(e3) - cos(e2)*cos(e3)))*(x6*(sin(e6)*(sin(e2 + e3)*sin(e5) - cos(e2 + e3)*cos(e4)*cos(e5)) - cos(e2 + e3)*cos(e6)*sin(e4)) + y6*(cos(e6)*(sin(e2 + e3)*sin(e5) - cos(e2 + e3)*cos(e4)*cos(e5)) + cos(e2 + e3)*sin(e4)*sin(e6)) - sin(e4)*sin(e5)*(a1 + d4*cos(e2 + e3) + a3*sin(e2 + e3) + a2*sin(e2))) - (cos(e5)*(cos(e2)*sin(e3) + cos(e3)*sin(e2)) - cos(e4)*sin(e5)*(sin(e2)*sin(e3) - cos(e2)*cos(e3)))*(y6*cos(e6)*(sin(e2 + e3)*cos(e5) + cos(e2 + e3)*cos(e4)*sin(e5)) - cos(e5)*sin(e4)*(a1 + d4*cos(e2 + e3) + a3*sin(e2 + e3) + a2*sin(e2)) + x6*sin(e6)*(sin(e2 + e3)*cos(e5) + cos(e2 + e3)*cos(e4)*sin(e5))) - (sin(e6)*(sin(e5)*(cos(e2)*sin(e3) + cos(e3)*sin(e2)) + cos(e4)*cos(e5)*(sin(e2)*sin(e3) - cos(e2)*cos(e3))) + cos(e6)*sin(e4)*(sin(e2)*sin(e3) - cos(e2)*cos(e3)))*(x6*(sin(e2 + e3)*sin(e5) - cos(e2 + e3)*cos(e4)*cos(e5)) + z6*cos(e6)*(sin(e2 + e3)*cos(e5) + cos(e2 + e3)*cos(e4)*sin(e5)) - sin(e4)*sin(e5)*sin(e6)*(a1 + d4*cos(e2 + e3) + a3*sin(e2 + e3) + a2*sin(e2))) + (cos(e6)*(sin(e5)*(cos(e2)*sin(e3) + cos(e3)*sin(e2)) + cos(e4)*cos(e5)*(sin(e2)*sin(e3) - cos(e2)*cos(e3))) - sin(e4)*sin(e6)*(sin(e2)*sin(e3) - cos(e2)*cos(e3)))*(z6*sin(e6)*(sin(e2 + e3)*cos(e5) + cos(e2 + e3)*cos(e4)*sin(e5)) - y6*(sin(e2 + e3)*sin(e5) - cos(e2 + e3)*cos(e4)*cos(e5)) + cos(e6)*sin(e4)*sin(e5)*(a1 + d4*cos(e2 + e3) + a3*sin(e2 + e3) + a2*sin(e2))) + cos(e6)*(cos(e5)*(cos(e2)*sin(e3) + cos(e3)*sin(e2)) - cos(e4)*sin(e5)*(sin(e2)*sin(e3) - cos(e2)*cos(e3)))*(y6*(sin(e2 + e3)*cos(e5) + cos(e2 + e3)*cos(e4)*sin(e5)) + z6*(sin(e6)*(sin(e2 + e3)*sin(e5) - cos(e2 + e3)*cos(e4)*cos(e5)) - cos(e2 + e3)*cos(e6)*sin(e4)) - cos(e4)*sin(e6)*(a1 + d4*cos(e2 + e3) + a3*sin(e2 + e3) + a2*sin(e2)) - cos(e5)*cos(e6)*sin(e4)*(a1 + d4*cos(e2 + e3) + a3*sin(e2 + e3) + a2*sin(e2))) + sin(e6)*(cos(e5)*(cos(e2)*sin(e3) + cos(e3)*sin(e2)) - cos(e4)*sin(e5)*(sin(e2)*sin(e3) - cos(e2)*cos(e3)))*(x6*(sin(e2 + e3)*cos(e5) + cos(e2 + e3)*cos(e4)*sin(e5)) - z6*(cos(e6)*(sin(e2 + e3)*sin(e5) - cos(e2 + e3)*cos(e4)*cos(e5)) + cos(e2 + e3)*sin(e4)*sin(e6)) + cos(e4)*cos(e6)*(a1 + d4*cos(e2 + e3) + a3*sin(e2 + e3) + a2*sin(e2)) - cos(e5)*sin(e4)*sin(e6)*(a1 + d4*cos(e2 + e3) + a3*sin(e2 + e3) + a2*sin(e2)))) + 2*m5*((cos(e4)*sin(e1) - sin(e4)*(cos(e1)*cos(e2)*sin(e3) + cos(e1)*cos(e3)*sin(e2)))*(cos(e4)*(a1 + d4*cos(e2 + e3) + a3*sin(e2 + e3) + a2*sin(e2)) + x5*(sin(e2 + e3)*cos(e5) + cos(e2 + e3)*cos(e4)*sin(e5)) - y5*(sin(e2 + e3)*sin(e5) - cos(e2 + e3)*cos(e4)*cos(e5))) + (sin(e5)*(cos(e1)*cos(e2)*cos(e3) - cos(e1)*sin(e2)*sin(e3)) + cos(e5)*(sin(e1)*sin(e4) + cos(e4)*(cos(e1)*cos(e2)*sin(e3) + cos(e1)*cos(e3)*sin(e2))))*(z5*(sin(e2 + e3)*cos(e5) + cos(e2 + e3)*cos(e4)*sin(e5)) + cos(e5)*sin(e4)*(a1 + d4*cos(e2 + e3) + a3*sin(e2 + e3) + a2*sin(e2)) + y5*cos(e2 + e3)*sin(e4)) - (cos(e5)*(cos(e1)*cos(e2)*cos(e3) - cos(e1)*sin(e2)*sin(e3)) - sin(e5)*(sin(e1)*sin(e4) + cos(e4)*(cos(e1)*cos(e2)*sin(e3) + cos(e1)*cos(e3)*sin(e2))))*(z5*(sin(e2 + e3)*sin(e5) - cos(e2 + e3)*cos(e4)*cos(e5)) + sin(e4)*sin(e5)*(a1 + d4*cos(e2 + e3) + a3*sin(e2 + e3) + a2*sin(e2)) + x5*cos(e2 + e3)*sin(e4)))*((x5*(sin(e2 + e3)*sin(e5) - cos(e2 + e3)*cos(e4)*cos(e5)) + y5*(sin(e2 + e3)*cos(e5) + cos(e2 + e3)*cos(e4)*sin(e5)))*(cos(e4)*sin(e1) - sin(e4)*(cos(e1)*cos(e2)*sin(e3) + cos(e1)*cos(e3)*sin(e2))) + (cos(e5)*(cos(e1)*cos(e2)*cos(e3) - cos(e1)*sin(e2)*sin(e3)) - sin(e5)*(sin(e1)*sin(e4) + cos(e4)*(cos(e1)*cos(e2)*sin(e3) + cos(e1)*cos(e3)*sin(e2))))*(z5*(sin(e2 + e3)*cos(e5) + cos(e2 + e3)*cos(e4)*sin(e5)) + cos(e5)*sin(e4)*(a1 + d4*cos(e2 + e3) + a3*sin(e2 + e3) + a2*sin(e2))) + (z5*(sin(e2 + e3)*sin(e5) - cos(e2 + e3)*cos(e4)*cos(e5)) + sin(e4)*sin(e5)*(a1 + d4*cos(e2 + e3) + a3*sin(e2 + e3) + a2*sin(e2)))*(sin(e5)*(cos(e1)*cos(e2)*cos(e3) - cos(e1)*sin(e2)*sin(e3)) + cos(e5)*(sin(e1)*sin(e4) + cos(e4)*(cos(e1)*cos(e2)*sin(e3) + cos(e1)*cos(e3)*sin(e2)))) - (cos(e5)*(cos(e1)*cos(e2)*cos(e3) - cos(e1)*sin(e2)*sin(e3)) - sin(e5)*(sin(e1)*sin(e4) + cos(e4)*(cos(e1)*cos(e2)*sin(e3) + cos(e1)*cos(e3)*sin(e2))))*(z5*(sin(e2 + e3)*cos(e5) + cos(e2 + e3)*cos(e4)*sin(e5)) + cos(e5)*sin(e4)*(a1 + d4*cos(e2 + e3) + a3*sin(e2 + e3) + a2*sin(e2)) + y5*cos(e2 + e3)*sin(e4)) - (sin(e5)*(cos(e1)*cos(e2)*cos(e3) - cos(e1)*sin(e2)*sin(e3)) + cos(e5)*(sin(e1)*sin(e4) + cos(e4)*(cos(e1)*cos(e2)*sin(e3) + cos(e1)*cos(e3)*sin(e2))))*(z5*(sin(e2 + e3)*sin(e5) - cos(e2 + e3)*cos(e4)*cos(e5)) + sin(e4)*sin(e5)*(a1 + d4*cos(e2 + e3) + a3*sin(e2 + e3) + a2*sin(e2)) + x5*cos(e2 + e3)*sin(e4))) + cos(e2 + e3)*sin(e4)*(I5xz*(sin(e2 + e3)*cos(e5) + cos(e2 + e3)*cos(e4)*sin(e5)) - I5yz*(sin(e2 + e3)*sin(e5) - cos(e2 + e3)*cos(e4)*cos(e5)))) - de6*((I6xz*(sin(e6)*(sin(e2 + e3)*sin(e5) - cos(e2 + e3)*cos(e4)*cos(e5)) - cos(e2 + e3)*cos(e6)*sin(e4)) + I6yz*(cos(e6)*(sin(e2 + e3)*sin(e5) - cos(e2 + e3)*cos(e4)*cos(e5)) + cos(e2 + e3)*sin(e4)*sin(e6)))*(sin(e2 + e3)*cos(e5) + cos(e2 + e3)*cos(e4)*sin(e5)) + (I6xx*(sin(e6)*(sin(e2 + e3)*sin(e5) - cos(e2 + e3)*cos(e4)*cos(e5)) - cos(e2 + e3)*cos(e6)*sin(e4)) + I6yx*(cos(e6)*(sin(e2 + e3)*sin(e5) - cos(e2 + e3)*cos(e4)*cos(e5)) + cos(e2 + e3)*sin(e4)*sin(e6)))*(cos(e6)*(sin(e2 + e3)*sin(e5) - cos(e2 + e3)*cos(e4)*cos(e5)) + cos(e2 + e3)*sin(e4)*sin(e6)) - (I6xy*(sin(e6)*(sin(e2 + e3)*sin(e5) - cos(e2 + e3)*cos(e4)*cos(e5)) - cos(e2 + e3)*cos(e6)*sin(e4)) + I6yy*(cos(e6)*(sin(e2 + e3)*sin(e5) - cos(e2 + e3)*cos(e4)*cos(e5)) + cos(e2 + e3)*sin(e4)*sin(e6)))*(sin(e6)*(sin(e2 + e3)*sin(e5) - cos(e2 + e3)*cos(e4)*cos(e5)) - cos(e2 + e3)*cos(e6)*sin(e4)) + (sin(e6)*(sin(e2 + e3)*sin(e5) - cos(e2 + e3)*cos(e4)*cos(e5)) - cos(e2 + e3)*cos(e6)*sin(e4))*(I6zx*(sin(e2 + e3)*cos(e5) + cos(e2 + e3)*cos(e4)*sin(e5)) + I6xx*(cos(e6)*(sin(e2 + e3)*sin(e5) - cos(e2 + e3)*cos(e4)*cos(e5)) + cos(e2 + e3)*sin(e4)*sin(e6)) - I6yx*(sin(e6)*(sin(e2 + e3)*sin(e5) - cos(e2 + e3)*cos(e4)*cos(e5)) - cos(e2 + e3)*cos(e6)*sin(e4))) + (cos(e6)*(sin(e2 + e3)*sin(e5) - cos(e2 + e3)*cos(e4)*cos(e5)) + cos(e2 + e3)*sin(e4)*sin(e6))*(I6zy*(sin(e2 + e3)*cos(e5) + cos(e2 + e3)*cos(e4)*sin(e5)) + I6xy*(cos(e6)*(sin(e2 + e3)*sin(e5) - cos(e2 + e3)*cos(e4)*cos(e5)) + cos(e2 + e3)*sin(e4)*sin(e6)) - I6yy*(sin(e6)*(sin(e2 + e3)*sin(e5) - cos(e2 + e3)*cos(e4)*cos(e5)) - cos(e2 + e3)*cos(e6)*sin(e4))) + 2*m6*((sin(e6)*(sin(e5)*(cos(e1)*cos(e2)*cos(e3) - cos(e1)*sin(e2)*sin(e3)) + cos(e5)*(sin(e1)*sin(e4) + cos(e4)*(cos(e1)*cos(e2)*sin(e3) + cos(e1)*cos(e3)*sin(e2)))) - cos(e6)*(cos(e4)*sin(e1) - sin(e4)*(cos(e1)*cos(e2)*sin(e3) + cos(e1)*cos(e3)*sin(e2))))*(x6*(sin(e2 + e3)*cos(e5) + cos(e2 + e3)*cos(e4)*sin(e5)) - z6*(cos(e6)*(sin(e2 + e3)*sin(e5) - cos(e2 + e3)*cos(e4)*cos(e5)) + cos(e2 + e3)*sin(e4)*sin(e6)) + cos(e4)*cos(e6)*(a1 + d4*cos(e2 + e3) + a3*sin(e2 + e3) + a2*sin(e2)) - cos(e5)*sin(e4)*sin(e6)*(a1 + d4*cos(e2 + e3) + a3*sin(e2 + e3) + a2*sin(e2))) + (cos(e6)*(sin(e5)*(cos(e1)*cos(e2)*cos(e3) - cos(e1)*sin(e2)*sin(e3)) + cos(e5)*(sin(e1)*sin(e4) + cos(e4)*(cos(e1)*cos(e2)*sin(e3) + cos(e1)*cos(e3)*sin(e2)))) + sin(e6)*(cos(e4)*sin(e1) - sin(e4)*(cos(e1)*cos(e2)*sin(e3) + cos(e1)*cos(e3)*sin(e2))))*(y6*(sin(e2 + e3)*cos(e5) + cos(e2 + e3)*cos(e4)*sin(e5)) + z6*(sin(e6)*(sin(e2 + e3)*sin(e5) - cos(e2 + e3)*cos(e4)*cos(e5)) - cos(e2 + e3)*cos(e6)*sin(e4)) - cos(e4)*sin(e6)*(a1 + d4*cos(e2 + e3) + a3*sin(e2 + e3) + a2*sin(e2)) - cos(e5)*cos(e6)*sin(e4)*(a1 + d4*cos(e2 + e3) + a3*sin(e2 + e3) + a2*sin(e2))) - (cos(e5)*(cos(e1)*cos(e2)*cos(e3) - cos(e1)*sin(e2)*sin(e3)) - sin(e5)*(sin(e1)*sin(e4) + cos(e4)*(cos(e1)*cos(e2)*sin(e3) + cos(e1)*cos(e3)*sin(e2))))*(x6*(sin(e6)*(sin(e2 + e3)*sin(e5) - cos(e2 + e3)*cos(e4)*cos(e5)) - cos(e2 + e3)*cos(e6)*sin(e4)) + y6*(cos(e6)*(sin(e2 + e3)*sin(e5) - cos(e2 + e3)*cos(e4)*cos(e5)) + cos(e2 + e3)*sin(e4)*sin(e6)) - sin(e4)*sin(e5)*(a1 + d4*cos(e2 + e3) + a3*sin(e2 + e3) + a2*sin(e2))))*((sin(e6)*(sin(e5)*(cos(e1)*cos(e2)*cos(e3) - cos(e1)*sin(e2)*sin(e3)) + cos(e5)*(sin(e1)*sin(e4) + cos(e4)*(cos(e1)*cos(e2)*sin(e3) + cos(e1)*cos(e3)*sin(e2)))) - cos(e6)*(cos(e4)*sin(e1) - sin(e4)*(cos(e1)*cos(e2)*sin(e3) + cos(e1)*cos(e3)*sin(e2))))*(y6*(sin(e2 + e3)*cos(e5) + cos(e2 + e3)*cos(e4)*sin(e5)) + z6*(sin(e6)*(sin(e2 + e3)*sin(e5) - cos(e2 + e3)*cos(e4)*cos(e5)) - cos(e2 + e3)*cos(e6)*sin(e4)) - cos(e4)*sin(e6)*(a1 + d4*cos(e2 + e3) + a3*sin(e2 + e3) + a2*sin(e2)) - cos(e5)*cos(e6)*sin(e4)*(a1 + d4*cos(e2 + e3) + a3*sin(e2 + e3) + a2*sin(e2))) - (cos(e6)*(sin(e5)*(cos(e1)*cos(e2)*cos(e3) - cos(e1)*sin(e2)*sin(e3)) + cos(e5)*(sin(e1)*sin(e4) + cos(e4)*(cos(e1)*cos(e2)*sin(e3) + cos(e1)*cos(e3)*sin(e2)))) + sin(e6)*(cos(e4)*sin(e1) - sin(e4)*(cos(e1)*cos(e2)*sin(e3) + cos(e1)*cos(e3)*sin(e2))))*(x6*(sin(e2 + e3)*cos(e5) + cos(e2 + e3)*cos(e4)*sin(e5)) - z6*(cos(e6)*(sin(e2 + e3)*sin(e5) - cos(e2 + e3)*cos(e4)*cos(e5)) + cos(e2 + e3)*sin(e4)*sin(e6)) + cos(e4)*cos(e6)*(a1 + d4*cos(e2 + e3) + a3*sin(e2 + e3) + a2*sin(e2)) - cos(e5)*sin(e4)*sin(e6)*(a1 + d4*cos(e2 + e3) + a3*sin(e2 + e3) + a2*sin(e2))) + (cos(e5)*(cos(e1)*cos(e2)*cos(e3) - cos(e1)*sin(e2)*sin(e3)) - sin(e5)*(sin(e1)*sin(e4) + cos(e4)*(cos(e1)*cos(e2)*sin(e3) + cos(e1)*cos(e3)*sin(e2))))*(x6*(cos(e6)*(sin(e2 + e3)*sin(e5) - cos(e2 + e3)*cos(e4)*cos(e5)) + cos(e2 + e3)*sin(e4)*sin(e6)) - y6*(sin(e6)*(sin(e2 + e3)*sin(e5) - cos(e2 + e3)*cos(e4)*cos(e5)) - cos(e2 + e3)*cos(e6)*sin(e4))) - (cos(e6)*(sin(e5)*(cos(e1)*cos(e2)*cos(e3) - cos(e1)*sin(e2)*sin(e3)) + cos(e5)*(sin(e1)*sin(e4) + cos(e4)*(cos(e1)*cos(e2)*sin(e3) + cos(e1)*cos(e3)*sin(e2)))) + sin(e6)*(cos(e4)*sin(e1) - sin(e4)*(cos(e1)*cos(e2)*sin(e3) + cos(e1)*cos(e3)*sin(e2))))*(z6*(cos(e6)*(sin(e2 + e3)*sin(e5) - cos(e2 + e3)*cos(e4)*cos(e5)) + cos(e2 + e3)*sin(e4)*sin(e6)) - cos(e4)*cos(e6)*(a1 + d4*cos(e2 + e3) + a3*sin(e2 + e3) + a2*sin(e2)) + cos(e5)*sin(e4)*sin(e6)*(a1 + d4*cos(e2 + e3) + a3*sin(e2 + e3) + a2*sin(e2))) + (sin(e6)*(sin(e5)*(cos(e1)*cos(e2)*cos(e3) - cos(e1)*sin(e2)*sin(e3)) + cos(e5)*(sin(e1)*sin(e4) + cos(e4)*(cos(e1)*cos(e2)*sin(e3) + cos(e1)*cos(e3)*sin(e2)))) - cos(e6)*(cos(e4)*sin(e1) - sin(e4)*(cos(e1)*cos(e2)*sin(e3) + cos(e1)*cos(e3)*sin(e2))))*(cos(e4)*sin(e6)*(a1 + d4*cos(e2 + e3) + a3*sin(e2 + e3) + a2*sin(e2)) - z6*(sin(e6)*(sin(e2 + e3)*sin(e5) - cos(e2 + e3)*cos(e4)*cos(e5)) - cos(e2 + e3)*cos(e6)*sin(e4)) + cos(e5)*cos(e6)*sin(e4)*(a1 + d4*cos(e2 + e3) + a3*sin(e2 + e3) + a2*sin(e2)))) + 2*m6*((sin(e6)*(sin(e5)*(cos(e2)*sin(e3) + cos(e3)*sin(e2)) + cos(e4)*cos(e5)*(sin(e2)*sin(e3) - cos(e2)*cos(e3))) + cos(e6)*sin(e4)*(sin(e2)*sin(e3) - cos(e2)*cos(e3)))*(x6*(sin(e2 + e3)*cos(e5) + cos(e2 + e3)*cos(e4)*sin(e5)) - z6*(cos(e6)*(sin(e2 + e3)*sin(e5) - cos(e2 + e3)*cos(e4)*cos(e5)) + cos(e2 + e3)*sin(e4)*sin(e6)) + cos(e4)*cos(e6)*(a1 + d4*cos(e2 + e3) + a3*sin(e2 + e3) + a2*sin(e2)) - cos(e5)*sin(e4)*sin(e6)*(a1 + d4*cos(e2 + e3) + a3*sin(e2 + e3) + a2*sin(e2))) + (cos(e6)*(sin(e5)*(cos(e2)*sin(e3) + cos(e3)*sin(e2)) + cos(e4)*cos(e5)*(sin(e2)*sin(e3) - cos(e2)*cos(e3))) - sin(e4)*sin(e6)*(sin(e2)*sin(e3) - cos(e2)*cos(e3)))*(y6*(sin(e2 + e3)*cos(e5) + cos(e2 + e3)*cos(e4)*sin(e5)) + z6*(sin(e6)*(sin(e2 + e3)*sin(e5) - cos(e2 + e3)*cos(e4)*cos(e5)) - cos(e2 + e3)*cos(e6)*sin(e4)) - cos(e4)*sin(e6)*(a1 + d4*cos(e2 + e3) + a3*sin(e2 + e3) + a2*sin(e2)) - cos(e5)*cos(e6)*sin(e4)*(a1 + d4*cos(e2 + e3) + a3*sin(e2 + e3) + a2*sin(e2))) - (cos(e5)*(cos(e2)*sin(e3) + cos(e3)*sin(e2)) - cos(e4)*sin(e5)*(sin(e2)*sin(e3) - cos(e2)*cos(e3)))*(x6*(sin(e6)*(sin(e2 + e3)*sin(e5) - cos(e2 + e3)*cos(e4)*cos(e5)) - cos(e2 + e3)*cos(e6)*sin(e4)) + y6*(cos(e6)*(sin(e2 + e3)*sin(e5) - cos(e2 + e3)*cos(e4)*cos(e5)) + cos(e2 + e3)*sin(e4)*sin(e6)) - sin(e4)*sin(e5)*(a1 + d4*cos(e2 + e3) + a3*sin(e2 + e3) + a2*sin(e2))))*((sin(e6)*(sin(e5)*(cos(e2)*sin(e3) + cos(e3)*sin(e2)) + cos(e4)*cos(e5)*(sin(e2)*sin(e3) - cos(e2)*cos(e3))) + cos(e6)*sin(e4)*(sin(e2)*sin(e3) - cos(e2)*cos(e3)))*(y6*(sin(e2 + e3)*cos(e5) + cos(e2 + e3)*cos(e4)*sin(e5)) + z6*(sin(e6)*(sin(e2 + e3)*sin(e5) - cos(e2 + e3)*cos(e4)*cos(e5)) - cos(e2 + e3)*cos(e6)*sin(e4)) - cos(e4)*sin(e6)*(a1 + d4*cos(e2 + e3) + a3*sin(e2 + e3) + a2*sin(e2)) - cos(e5)*cos(e6)*sin(e4)*(a1 + d4*cos(e2 + e3) + a3*sin(e2 + e3) + a2*sin(e2))) - (cos(e6)*(sin(e5)*(cos(e2)*sin(e3) + cos(e3)*sin(e2)) + cos(e4)*cos(e5)*(sin(e2)*sin(e3) - cos(e2)*cos(e3))) - sin(e4)*sin(e6)*(sin(e2)*sin(e3) - cos(e2)*cos(e3)))*(x6*(sin(e2 + e3)*cos(e5) + cos(e2 + e3)*cos(e4)*sin(e5)) - z6*(cos(e6)*(sin(e2 + e3)*sin(e5) - cos(e2 + e3)*cos(e4)*cos(e5)) + cos(e2 + e3)*sin(e4)*sin(e6)) + cos(e4)*cos(e6)*(a1 + d4*cos(e2 + e3) + a3*sin(e2 + e3) + a2*sin(e2)) - cos(e5)*sin(e4)*sin(e6)*(a1 + d4*cos(e2 + e3) + a3*sin(e2 + e3) + a2*sin(e2))) + (cos(e5)*(cos(e2)*sin(e3) + cos(e3)*sin(e2)) - cos(e4)*sin(e5)*(sin(e2)*sin(e3) - cos(e2)*cos(e3)))*(x6*(cos(e6)*(sin(e2 + e3)*sin(e5) - cos(e2 + e3)*cos(e4)*cos(e5)) + cos(e2 + e3)*sin(e4)*sin(e6)) - y6*(sin(e6)*(sin(e2 + e3)*sin(e5) - cos(e2 + e3)*cos(e4)*cos(e5)) - cos(e2 + e3)*cos(e6)*sin(e4))) + (sin(e6)*(sin(e5)*(cos(e2)*sin(e3) + cos(e3)*sin(e2)) + cos(e4)*cos(e5)*(sin(e2)*sin(e3) - cos(e2)*cos(e3))) + cos(e6)*sin(e4)*(sin(e2)*sin(e3) - cos(e2)*cos(e3)))*(cos(e4)*sin(e6)*(a1 + d4*cos(e2 + e3) + a3*sin(e2 + e3) + a2*sin(e2)) - z6*(sin(e6)*(sin(e2 + e3)*sin(e5) - cos(e2 + e3)*cos(e4)*cos(e5)) - cos(e2 + e3)*cos(e6)*sin(e4)) + cos(e5)*cos(e6)*sin(e4)*(a1 + d4*cos(e2 + e3) + a3*sin(e2 + e3) + a2*sin(e2))) - (cos(e6)*(sin(e5)*(cos(e2)*sin(e3) + cos(e3)*sin(e2)) + cos(e4)*cos(e5)*(sin(e2)*sin(e3) - cos(e2)*cos(e3))) - sin(e4)*sin(e6)*(sin(e2)*sin(e3) - cos(e2)*cos(e3)))*(z6*(cos(e6)*(sin(e2 + e3)*sin(e5) - cos(e2 + e3)*cos(e4)*cos(e5)) + cos(e2 + e3)*sin(e4)*sin(e6)) - cos(e4)*cos(e6)*(a1 + d4*cos(e2 + e3) + a3*sin(e2 + e3) + a2*sin(e2)) + cos(e5)*sin(e4)*sin(e6)*(a1 + d4*cos(e2 + e3) + a3*sin(e2 + e3) + a2*sin(e2)))) + 2*m6*((sin(e6)*(sin(e5)*(cos(e2)*cos(e3)*sin(e1) - sin(e1)*sin(e2)*sin(e3)) - cos(e5)*(cos(e1)*sin(e4) - cos(e4)*(cos(e2)*sin(e1)*sin(e3) + cos(e3)*sin(e1)*sin(e2)))) + cos(e6)*(sin(e4)*(cos(e2)*sin(e1)*sin(e3) + cos(e3)*sin(e1)*sin(e2)) + cos(e1)*cos(e4)))*(x6*(sin(e2 + e3)*cos(e5) + cos(e2 + e3)*cos(e4)*sin(e5)) - z6*(cos(e6)*(sin(e2 + e3)*sin(e5) - cos(e2 + e3)*cos(e4)*cos(e5)) + cos(e2 + e3)*sin(e4)*sin(e6)) + cos(e4)*cos(e6)*(a1 + d4*cos(e2 + e3) + a3*sin(e2 + e3) + a2*sin(e2)) - cos(e5)*sin(e4)*sin(e6)*(a1 + d4*cos(e2 + e3) + a3*sin(e2 + e3) + a2*sin(e2))) + (cos(e6)*(sin(e5)*(cos(e2)*cos(e3)*sin(e1) - sin(e1)*sin(e2)*sin(e3)) - cos(e5)*(cos(e1)*sin(e4) - cos(e4)*(cos(e2)*sin(e1)*sin(e3) + cos(e3)*sin(e1)*sin(e2)))) - sin(e6)*(sin(e4)*(cos(e2)*sin(e1)*sin(e3) + cos(e3)*sin(e1)*sin(e2)) + cos(e1)*cos(e4)))*(y6*(sin(e2 + e3)*cos(e5) + cos(e2 + e3)*cos(e4)*sin(e5)) + z6*(sin(e6)*(sin(e2 + e3)*sin(e5) - cos(e2 + e3)*cos(e4)*cos(e5)) - cos(e2 + e3)*cos(e6)*sin(e4)) - cos(e4)*sin(e6)*(a1 + d4*cos(e2 + e3) + a3*sin(e2 + e3) + a2*sin(e2)) - cos(e5)*cos(e6)*sin(e4)*(a1 + d4*cos(e2 + e3) + a3*sin(e2 + e3) + a2*sin(e2))) - (cos(e5)*(cos(e2)*cos(e3)*sin(e1) - sin(e1)*sin(e2)*sin(e3)) + sin(e5)*(cos(e1)*sin(e4) - cos(e4)*(cos(e2)*sin(e1)*sin(e3) + cos(e3)*sin(e1)*sin(e2))))*(x6*(sin(e6)*(sin(e2 + e3)*sin(e5) - cos(e2 + e3)*cos(e4)*cos(e5)) - cos(e2 + e3)*cos(e6)*sin(e4)) + y6*(cos(e6)*(sin(e2 + e3)*sin(e5) - cos(e2 + e3)*cos(e4)*cos(e5)) + cos(e2 + e3)*sin(e4)*sin(e6)) - sin(e4)*sin(e5)*(a1 + d4*cos(e2 + e3) + a3*sin(e2 + e3) + a2*sin(e2))))*((sin(e6)*(sin(e5)*(cos(e2)*cos(e3)*sin(e1) - sin(e1)*sin(e2)*sin(e3)) - cos(e5)*(cos(e1)*sin(e4) - cos(e4)*(cos(e2)*sin(e1)*sin(e3) + cos(e3)*sin(e1)*sin(e2)))) + cos(e6)*(sin(e4)*(cos(e2)*sin(e1)*sin(e3) + cos(e3)*sin(e1)*sin(e2)) + cos(e1)*cos(e4)))*(cos(e4)*sin(e6)*(a1 + d4*cos(e2 + e3) + a3*sin(e2 + e3) + a2*sin(e2)) - z6*(sin(e6)*(sin(e2 + e3)*sin(e5) - cos(e2 + e3)*cos(e4)*cos(e5)) - cos(e2 + e3)*cos(e6)*sin(e4)) + cos(e5)*cos(e6)*sin(e4)*(a1 + d4*cos(e2 + e3) + a3*sin(e2 + e3) + a2*sin(e2))) - (cos(e6)*(sin(e5)*(cos(e2)*cos(e3)*sin(e1) - sin(e1)*sin(e2)*sin(e3)) - cos(e5)*(cos(e1)*sin(e4) - cos(e4)*(cos(e2)*sin(e1)*sin(e3) + cos(e3)*sin(e1)*sin(e2)))) - sin(e6)*(sin(e4)*(cos(e2)*sin(e1)*sin(e3) + cos(e3)*sin(e1)*sin(e2)) + cos(e1)*cos(e4)))*(z6*(cos(e6)*(sin(e2 + e3)*sin(e5) - cos(e2 + e3)*cos(e4)*cos(e5)) + cos(e2 + e3)*sin(e4)*sin(e6)) - cos(e4)*cos(e6)*(a1 + d4*cos(e2 + e3) + a3*sin(e2 + e3) + a2*sin(e2)) + cos(e5)*sin(e4)*sin(e6)*(a1 + d4*cos(e2 + e3) + a3*sin(e2 + e3) + a2*sin(e2))) + (cos(e5)*(cos(e2)*cos(e3)*sin(e1) - sin(e1)*sin(e2)*sin(e3)) + sin(e5)*(cos(e1)*sin(e4) - cos(e4)*(cos(e2)*sin(e1)*sin(e3) + cos(e3)*sin(e1)*sin(e2))))*(x6*(cos(e6)*(sin(e2 + e3)*sin(e5) - cos(e2 + e3)*cos(e4)*cos(e5)) + cos(e2 + e3)*sin(e4)*sin(e6)) - y6*(sin(e6)*(sin(e2 + e3)*sin(e5) - cos(e2 + e3)*cos(e4)*cos(e5)) - cos(e2 + e3)*cos(e6)*sin(e4))) - (cos(e6)*(sin(e5)*(cos(e2)*cos(e3)*sin(e1) - sin(e1)*sin(e2)*sin(e3)) - cos(e5)*(cos(e1)*sin(e4) - cos(e4)*(cos(e2)*sin(e1)*sin(e3) + cos(e3)*sin(e1)*sin(e2)))) - sin(e6)*(sin(e4)*(cos(e2)*sin(e1)*sin(e3) + cos(e3)*sin(e1)*sin(e2)) + cos(e1)*cos(e4)))*(x6*(sin(e2 + e3)*cos(e5) + cos(e2 + e3)*cos(e4)*sin(e5)) - z6*(cos(e6)*(sin(e2 + e3)*sin(e5) - cos(e2 + e3)*cos(e4)*cos(e5)) + cos(e2 + e3)*sin(e4)*sin(e6)) + cos(e4)*cos(e6)*(a1 + d4*cos(e2 + e3) + a3*sin(e2 + e3) + a2*sin(e2)) - cos(e5)*sin(e4)*sin(e6)*(a1 + d4*cos(e2 + e3) + a3*sin(e2 + e3) + a2*sin(e2))) + (sin(e6)*(sin(e5)*(cos(e2)*cos(e3)*sin(e1) - sin(e1)*sin(e2)*sin(e3)) - cos(e5)*(cos(e1)*sin(e4) - cos(e4)*(cos(e2)*sin(e1)*sin(e3) + cos(e3)*sin(e1)*sin(e2)))) + cos(e6)*(sin(e4)*(cos(e2)*sin(e1)*sin(e3) + cos(e3)*sin(e1)*sin(e2)) + cos(e1)*cos(e4)))*(y6*(sin(e2 + e3)*cos(e5) + cos(e2 + e3)*cos(e4)*sin(e5)) + z6*(sin(e6)*(sin(e2 + e3)*sin(e5) - cos(e2 + e3)*cos(e4)*cos(e5)) - cos(e2 + e3)*cos(e6)*sin(e4)) - cos(e4)*sin(e6)*(a1 + d4*cos(e2 + e3) + a3*sin(e2 + e3) + a2*sin(e2)) - cos(e5)*cos(e6)*sin(e4)*(a1 + d4*cos(e2 + e3) + a3*sin(e2 + e3) + a2*sin(e2))))) + de3*((cos(e6)*(sin(e2 + e3)*sin(e5) - cos(e2 + e3)*cos(e4)*cos(e5)) + cos(e2 + e3)*sin(e4)*sin(e6))*(I6zx*(cos(e2 + e3)*cos(e5) - sin(e2 + e3)*cos(e4)*sin(e5)) + I6xx*(cos(e6)*(cos(e2 + e3)*sin(e5) + sin(e2 + e3)*cos(e4)*cos(e5)) - sin(e2 + e3)*sin(e4)*sin(e6)) - I6yx*(sin(e6)*(cos(e2 + e3)*sin(e5) + sin(e2 + e3)*cos(e4)*cos(e5)) + sin(e2 + e3)*cos(e6)*sin(e4))) - (sin(e6)*(sin(e2 + e3)*sin(e5) - cos(e2 + e3)*cos(e4)*cos(e5)) - cos(e2 + e3)*cos(e6)*sin(e4))*(I6zy*(cos(e2 + e3)*cos(e5) - sin(e2 + e3)*cos(e4)*sin(e5)) + I6xy*(cos(e6)*(cos(e2 + e3)*sin(e5) + sin(e2 + e3)*cos(e4)*cos(e5)) - sin(e2 + e3)*sin(e4)*sin(e6)) - I6yy*(sin(e6)*(cos(e2 + e3)*sin(e5) + sin(e2 + e3)*cos(e4)*cos(e5)) + sin(e2 + e3)*cos(e6)*sin(e4))) + (cos(e2 + e3)*sin(e5) + sin(e2 + e3)*cos(e4)*cos(e5))*(I5xx*(sin(e2 + e3)*sin(e5) - cos(e2 + e3)*cos(e4)*cos(e5)) + I5yx*(sin(e2 + e3)*cos(e5) + cos(e2 + e3)*cos(e4)*sin(e5)) - I5zx*cos(e2 + e3)*sin(e4)) + (cos(e2 + e3)*cos(e5) - sin(e2 + e3)*cos(e4)*sin(e5))*(I5xy*(sin(e2 + e3)*sin(e5) - cos(e2 + e3)*cos(e4)*cos(e5)) + I5yy*(sin(e2 + e3)*cos(e5) + cos(e2 + e3)*cos(e4)*sin(e5)) - I5zy*cos(e2 + e3)*sin(e4)) + (sin(e2 + e3)*sin(e5) - cos(e2 + e3)*cos(e4)*cos(e5))*(I5xx*(cos(e2 + e3)*sin(e5) + sin(e2 + e3)*cos(e4)*cos(e5)) + I5yx*(cos(e2 + e3)*cos(e5) - sin(e2 + e3)*cos(e4)*sin(e5)) + I5zx*sin(e2 + e3)*sin(e4)) + (sin(e2 + e3)*cos(e5) + cos(e2 + e3)*cos(e4)*sin(e5))*(I5xy*(cos(e2 + e3)*sin(e5) + sin(e2 + e3)*cos(e4)*cos(e5)) + I5yy*(cos(e2 + e3)*cos(e5) - sin(e2 + e3)*cos(e4)*sin(e5)) + I5zy*sin(e2 + e3)*sin(e4)) + cos(e2 + e3)*(I4zz*sin(e2 + e3) + I4yz*cos(e2 + e3)*sin(e4) - I4xz*cos(e2 + e3)*cos(e4)) + sin(e2 + e3)*(I4zz*cos(e2 + e3) + I4xz*sin(e2 + e3)*cos(e4) - I4yz*sin(e2 + e3)*sin(e4)) + (cos(e2 + e3)*cos(e5) - sin(e2 + e3)*cos(e4)*sin(e5))*(I6zz*(sin(e2 + e3)*cos(e5) + cos(e2 + e3)*cos(e4)*sin(e5)) + I6xz*(cos(e6)*(sin(e2 + e3)*sin(e5) - cos(e2 + e3)*cos(e4)*cos(e5)) + cos(e2 + e3)*sin(e4)*sin(e6)) - I6yz*(sin(e6)*(sin(e2 + e3)*sin(e5) - cos(e2 + e3)*cos(e4)*cos(e5)) - cos(e2 + e3)*cos(e6)*sin(e4))) - cos(e2 + e3)*(I3yx*cos(e2 + e3) + I3xx*sin(e2 + e3)) - cos(e2 + e3)*(I3xy*cos(e2 + e3) - I3yy*sin(e2 + e3)) - sin(e2 + e3)*(I3xx*cos(e2 + e3) - I3yx*sin(e2 + e3)) + sin(e2 + e3)*(I3yy*cos(e2 + e3) + I3xy*sin(e2 + e3)) + (sin(e2 + e3)*cos(e5) + cos(e2 + e3)*cos(e4)*sin(e5))*(I6zz*(cos(e2 + e3)*cos(e5) - sin(e2 + e3)*cos(e4)*sin(e5)) + I6xz*(cos(e6)*(cos(e2 + e3)*sin(e5) + sin(e2 + e3)*cos(e4)*cos(e5)) - sin(e2 + e3)*sin(e4)*sin(e6)) - I6yz*(sin(e6)*(cos(e2 + e3)*sin(e5) + sin(e2 + e3)*cos(e4)*cos(e5)) + sin(e2 + e3)*cos(e6)*sin(e4))) + (cos(e6)*(cos(e2 + e3)*sin(e5) + sin(e2 + e3)*cos(e4)*cos(e5)) - sin(e2 + e3)*sin(e4)*sin(e6))*(I6zx*(sin(e2 + e3)*cos(e5) + cos(e2 + e3)*cos(e4)*sin(e5)) + I6xx*(cos(e6)*(sin(e2 + e3)*sin(e5) - cos(e2 + e3)*cos(e4)*cos(e5)) + cos(e2 + e3)*sin(e4)*sin(e6)) - I6yx*(sin(e6)*(sin(e2 + e3)*sin(e5) - cos(e2 + e3)*cos(e4)*cos(e5)) - cos(e2 + e3)*cos(e6)*sin(e4))) - (sin(e6)*(cos(e2 + e3)*sin(e5) + sin(e2 + e3)*cos(e4)*cos(e5)) + sin(e2 + e3)*cos(e6)*sin(e4))*(I6zy*(sin(e2 + e3)*cos(e5) + cos(e2 + e3)*cos(e4)*sin(e5)) + I6xy*(cos(e6)*(sin(e2 + e3)*sin(e5) - cos(e2 + e3)*cos(e4)*cos(e5)) + cos(e2 + e3)*sin(e4)*sin(e6)) - I6yy*(sin(e6)*(sin(e2 + e3)*sin(e5) - cos(e2 + e3)*cos(e4)*cos(e5)) - cos(e2 + e3)*cos(e6)*sin(e4))) + 2*m6*((sin(e6)*(sin(e5)*(cos(e1)*cos(e2)*cos(e3) - cos(e1)*sin(e2)*sin(e3)) + cos(e5)*(sin(e1)*sin(e4) + cos(e4)*(cos(e1)*cos(e2)*sin(e3) + cos(e1)*cos(e3)*sin(e2)))) - cos(e6)*(cos(e4)*sin(e1) - sin(e4)*(cos(e1)*cos(e2)*sin(e3) + cos(e1)*cos(e3)*sin(e2))))*(x6*(sin(e2 + e3)*cos(e5) + cos(e2 + e3)*cos(e4)*sin(e5)) - z6*(cos(e6)*(sin(e2 + e3)*sin(e5) - cos(e2 + e3)*cos(e4)*cos(e5)) + cos(e2 + e3)*sin(e4)*sin(e6)) + cos(e4)*cos(e6)*(a1 + d4*cos(e2 + e3) + a3*sin(e2 + e3) + a2*sin(e2)) - cos(e5)*sin(e4)*sin(e6)*(a1 + d4*cos(e2 + e3) + a3*sin(e2 + e3) + a2*sin(e2))) + (cos(e6)*(sin(e5)*(cos(e1)*cos(e2)*cos(e3) - cos(e1)*sin(e2)*sin(e3)) + cos(e5)*(sin(e1)*sin(e4) + cos(e4)*(cos(e1)*cos(e2)*sin(e3) + cos(e1)*cos(e3)*sin(e2)))) + sin(e6)*(cos(e4)*sin(e1) - sin(e4)*(cos(e1)*cos(e2)*sin(e3) + cos(e1)*cos(e3)*sin(e2))))*(y6*(sin(e2 + e3)*cos(e5) + cos(e2 + e3)*cos(e4)*sin(e5)) + z6*(sin(e6)*(sin(e2 + e3)*sin(e5) - cos(e2 + e3)*cos(e4)*cos(e5)) - cos(e2 + e3)*cos(e6)*sin(e4)) - cos(e4)*sin(e6)*(a1 + d4*cos(e2 + e3) + a3*sin(e2 + e3) + a2*sin(e2)) - cos(e5)*cos(e6)*sin(e4)*(a1 + d4*cos(e2 + e3) + a3*sin(e2 + e3) + a2*sin(e2))) - (cos(e5)*(cos(e1)*cos(e2)*cos(e3) - cos(e1)*sin(e2)*sin(e3)) - sin(e5)*(sin(e1)*sin(e4) + cos(e4)*(cos(e1)*cos(e2)*sin(e3) + cos(e1)*cos(e3)*sin(e2))))*(x6*(sin(e6)*(sin(e2 + e3)*sin(e5) - cos(e2 + e3)*cos(e4)*cos(e5)) - cos(e2 + e3)*cos(e6)*sin(e4)) + y6*(cos(e6)*(sin(e2 + e3)*sin(e5) - cos(e2 + e3)*cos(e4)*cos(e5)) + cos(e2 + e3)*sin(e4)*sin(e6)) - sin(e4)*sin(e5)*(a1 + d4*cos(e2 + e3) + a3*sin(e2 + e3) + a2*sin(e2))))*((sin(e6)*(sin(e5)*(cos(e1)*cos(e2)*cos(e3) - cos(e1)*sin(e2)*sin(e3)) + cos(e5)*(sin(e1)*sin(e4) + cos(e4)*(cos(e1)*cos(e2)*sin(e3) + cos(e1)*cos(e3)*sin(e2)))) - cos(e6)*(cos(e4)*sin(e1) - sin(e4)*(cos(e1)*cos(e2)*sin(e3) + cos(e1)*cos(e3)*sin(e2))))*(x6*(cos(e2 + e3)*cos(e5) - sin(e2 + e3)*cos(e4)*sin(e5)) - z6*(cos(e6)*(cos(e2 + e3)*sin(e5) + sin(e2 + e3)*cos(e4)*cos(e5)) - sin(e2 + e3)*sin(e4)*sin(e6)) + cos(e4)*cos(e6)*(a3*cos(e2 + e3) - d4*sin(e2 + e3)) - cos(e5)*sin(e4)*sin(e6)*(a3*cos(e2 + e3) - d4*sin(e2 + e3))) + (cos(e6)*(sin(e5)*(cos(e1)*cos(e2)*cos(e3) - cos(e1)*sin(e2)*sin(e3)) + cos(e5)*(sin(e1)*sin(e4) + cos(e4)*(cos(e1)*cos(e2)*sin(e3) + cos(e1)*cos(e3)*sin(e2)))) + sin(e6)*(cos(e4)*sin(e1) - sin(e4)*(cos(e1)*cos(e2)*sin(e3) + cos(e1)*cos(e3)*sin(e2))))*(y6*(cos(e2 + e3)*cos(e5) - sin(e2 + e3)*cos(e4)*sin(e5)) + z6*(sin(e6)*(cos(e2 + e3)*sin(e5) + sin(e2 + e3)*cos(e4)*cos(e5)) + sin(e2 + e3)*cos(e6)*sin(e4)) - cos(e4)*sin(e6)*(a3*cos(e2 + e3) - d4*sin(e2 + e3)) - cos(e5)*cos(e6)*sin(e4)*(a3*cos(e2 + e3) - d4*sin(e2 + e3))) - (cos(e5)*(cos(e1)*cos(e2)*cos(e3) - cos(e1)*sin(e2)*sin(e3)) - sin(e5)*(sin(e1)*sin(e4) + cos(e4)*(cos(e1)*cos(e2)*sin(e3) + cos(e1)*cos(e3)*sin(e2))))*(x6*(sin(e6)*(cos(e2 + e3)*sin(e5) + sin(e2 + e3)*cos(e4)*cos(e5)) + sin(e2 + e3)*cos(e6)*sin(e4)) + y6*(cos(e6)*(cos(e2 + e3)*sin(e5) + sin(e2 + e3)*cos(e4)*cos(e5)) - sin(e2 + e3)*sin(e4)*sin(e6)) - sin(e4)*sin(e5)*(a3*cos(e2 + e3) - d4*sin(e2 + e3))) + (cos(e5)*(cos(e1)*cos(e2)*sin(e3) + cos(e1)*cos(e3)*sin(e2)) + cos(e4)*sin(e5)*(cos(e1)*cos(e2)*cos(e3) - cos(e1)*sin(e2)*sin(e3)))*(x6*(sin(e6)*(sin(e2 + e3)*sin(e5) - cos(e2 + e3)*cos(e4)*cos(e5)) - cos(e2 + e3)*cos(e6)*sin(e4)) + y6*(cos(e6)*(sin(e2 + e3)*sin(e5) - cos(e2 + e3)*cos(e4)*cos(e5)) + cos(e2 + e3)*sin(e4)*sin(e6)) - sin(e4)*sin(e5)*(a1 + d4*cos(e2 + e3) + a3*sin(e2 + e3) + a2*sin(e2))) - (sin(e6)*(sin(e5)*(cos(e1)*cos(e2)*sin(e3) + cos(e1)*cos(e3)*sin(e2)) - cos(e4)*cos(e5)*(cos(e1)*cos(e2)*cos(e3) - cos(e1)*sin(e2)*sin(e3))) - cos(e6)*sin(e4)*(cos(e1)*cos(e2)*cos(e3) - cos(e1)*sin(e2)*sin(e3)))*(x6*(sin(e2 + e3)*cos(e5) + cos(e2 + e3)*cos(e4)*sin(e5)) - z6*(cos(e6)*(sin(e2 + e3)*sin(e5) - cos(e2 + e3)*cos(e4)*cos(e5)) + cos(e2 + e3)*sin(e4)*sin(e6)) + cos(e4)*cos(e6)*(a1 + d4*cos(e2 + e3) + a3*sin(e2 + e3) + a2*sin(e2)) - cos(e5)*sin(e4)*sin(e6)*(a1 + d4*cos(e2 + e3) + a3*sin(e2 + e3) + a2*sin(e2))) - (cos(e6)*(sin(e5)*(cos(e1)*cos(e2)*sin(e3) + cos(e1)*cos(e3)*sin(e2)) - cos(e4)*cos(e5)*(cos(e1)*cos(e2)*cos(e3) - cos(e1)*sin(e2)*sin(e3))) + sin(e4)*sin(e6)*(cos(e1)*cos(e2)*cos(e3) - cos(e1)*sin(e2)*sin(e3)))*(y6*(sin(e2 + e3)*cos(e5) + cos(e2 + e3)*cos(e4)*sin(e5)) + z6*(sin(e6)*(sin(e2 + e3)*sin(e5) - cos(e2 + e3)*cos(e4)*cos(e5)) - cos(e2 + e3)*cos(e6)*sin(e4)) - cos(e4)*sin(e6)*(a1 + d4*cos(e2 + e3) + a3*sin(e2 + e3) + a2*sin(e2)) - cos(e5)*cos(e6)*sin(e4)*(a1 + d4*cos(e2 + e3) + a3*sin(e2 + e3) + a2*sin(e2)))) - 2*m4*((cos(e2)*sin(e3) + cos(e3)*sin(e2))*(y4*cos(e2 + e3)*cos(e4) + x4*cos(e2 + e3)*sin(e4)) + sin(e4)*(sin(e2)*sin(e3) - cos(e2)*cos(e3))*(cos(e4)*(a1 + d4*cos(e2 + e3) + a3*sin(e2 + e3) + a2*sin(e2)) + x4*sin(e2 + e3) + z4*cos(e2 + e3)*cos(e4)) - cos(e4)*(sin(e2)*sin(e3) - cos(e2)*cos(e3))*(sin(e4)*(a1 + d4*cos(e2 + e3) + a3*sin(e2 + e3) + a2*sin(e2)) - y4*sin(e2 + e3) + z4*cos(e2 + e3)*sin(e4)))*((sin(e2)*sin(e3) - cos(e2)*cos(e3))*(y4*cos(e2 + e3)*cos(e4) + x4*cos(e2 + e3)*sin(e4)) + (cos(e2)*sin(e3) + cos(e3)*sin(e2))*(y4*sin(e2 + e3)*cos(e4) + x4*sin(e2 + e3)*sin(e4)) - sin(e4)*(cos(e2)*sin(e3) + cos(e3)*sin(e2))*(cos(e4)*(a1 + d4*cos(e2 + e3) + a3*sin(e2 + e3) + a2*sin(e2)) + x4*sin(e2 + e3) + z4*cos(e2 + e3)*cos(e4)) - sin(e4)*(sin(e2)*sin(e3) - cos(e2)*cos(e3))*(cos(e4)*(a3*cos(e2 + e3) - d4*sin(e2 + e3)) + x4*cos(e2 + e3) - z4*sin(e2 + e3)*cos(e4)) + cos(e4)*(cos(e2)*sin(e3) + cos(e3)*sin(e2))*(sin(e4)*(a1 + d4*cos(e2 + e3) + a3*sin(e2 + e3) + a2*sin(e2)) - y4*sin(e2 + e3) + z4*cos(e2 + e3)*sin(e4)) - cos(e4)*(sin(e2)*sin(e3) - cos(e2)*cos(e3))*(y4*cos(e2 + e3) - sin(e4)*(a3*cos(e2 + e3) - d4*sin(e2 + e3)) + z4*sin(e2 + e3)*sin(e4))) + 2*m5*((cos(e5)*(cos(e2)*cos(e3)*sin(e1) - sin(e1)*sin(e2)*sin(e3)) + sin(e5)*(cos(e1)*sin(e4) - cos(e4)*(cos(e2)*sin(e1)*sin(e3) + cos(e3)*sin(e1)*sin(e2))))*(z5*(sin(e2 + e3)*sin(e5) - cos(e2 + e3)*cos(e4)*cos(e5)) + sin(e4)*sin(e5)*(a1 + d4*cos(e2 + e3) + a3*sin(e2 + e3) + a2*sin(e2)) + x5*cos(e2 + e3)*sin(e4)) + (sin(e4)*(cos(e2)*sin(e1)*sin(e3) + cos(e3)*sin(e1)*sin(e2)) + cos(e1)*cos(e4))*(cos(e4)*(a1 + d4*cos(e2 + e3) + a3*sin(e2 + e3) + a2*sin(e2)) + x5*(sin(e2 + e3)*cos(e5) + cos(e2 + e3)*cos(e4)*sin(e5)) - y5*(sin(e2 + e3)*sin(e5) - cos(e2 + e3)*cos(e4)*cos(e5))) - (sin(e5)*(cos(e2)*cos(e3)*sin(e1) - sin(e1)*sin(e2)*sin(e3)) - cos(e5)*(cos(e1)*sin(e4) - cos(e4)*(cos(e2)*sin(e1)*sin(e3) + cos(e3)*sin(e1)*sin(e2))))*(z5*(sin(e2 + e3)*cos(e5) + cos(e2 + e3)*cos(e4)*sin(e5)) + cos(e5)*sin(e4)*(a1 + d4*cos(e2 + e3) + a3*sin(e2 + e3) + a2*sin(e2)) + y5*cos(e2 + e3)*sin(e4)))*((cos(e5)*(cos(e2)*cos(e3)*sin(e1) - sin(e1)*sin(e2)*sin(e3)) + sin(e5)*(cos(e1)*sin(e4) - cos(e4)*(cos(e2)*sin(e1)*sin(e3) + cos(e3)*sin(e1)*sin(e2))))*(z5*(cos(e2 + e3)*sin(e5) + sin(e2 + e3)*cos(e4)*cos(e5)) + sin(e4)*sin(e5)*(a3*cos(e2 + e3) - d4*sin(e2 + e3)) - x5*sin(e2 + e3)*sin(e4)) - (sin(e5)*(cos(e2)*cos(e3)*sin(e1) - sin(e1)*sin(e2)*sin(e3)) - cos(e5)*(cos(e1)*sin(e4) - cos(e4)*(cos(e2)*sin(e1)*sin(e3) + cos(e3)*sin(e1)*sin(e2))))*(z5*(cos(e2 + e3)*cos(e5) - sin(e2 + e3)*cos(e4)*sin(e5)) + cos(e5)*sin(e4)*(a3*cos(e2 + e3) - d4*sin(e2 + e3)) - y5*sin(e2 + e3)*sin(e4)) + (sin(e5)*(cos(e2)*sin(e1)*sin(e3) + cos(e3)*sin(e1)*sin(e2)) - cos(e4)*cos(e5)*(cos(e2)*cos(e3)*sin(e1) - sin(e1)*sin(e2)*sin(e3)))*(z5*(sin(e2 + e3)*cos(e5) + cos(e2 + e3)*cos(e4)*sin(e5)) + cos(e5)*sin(e4)*(a1 + d4*cos(e2 + e3) + a3*sin(e2 + e3) + a2*sin(e2)) + y5*cos(e2 + e3)*sin(e4)) - (cos(e5)*(cos(e2)*sin(e1)*sin(e3) + cos(e3)*sin(e1)*sin(e2)) + cos(e4)*sin(e5)*(cos(e2)*cos(e3)*sin(e1) - sin(e1)*sin(e2)*sin(e3)))*(z5*(sin(e2 + e3)*sin(e5) - cos(e2 + e3)*cos(e4)*cos(e5)) + sin(e4)*sin(e5)*(a1 + d4*cos(e2 + e3) + a3*sin(e2 + e3) + a2*sin(e2)) + x5*cos(e2 + e3)*sin(e4)) + (sin(e4)*(cos(e2)*sin(e1)*sin(e3) + cos(e3)*sin(e1)*sin(e2)) + cos(e1)*cos(e4))*(cos(e4)*(a3*cos(e2 + e3) - d4*sin(e2 + e3)) + x5*(cos(e2 + e3)*cos(e5) - sin(e2 + e3)*cos(e4)*sin(e5)) - y5*(cos(e2 + e3)*sin(e5) + sin(e2 + e3)*cos(e4)*cos(e5))) + sin(e4)*(cos(e2)*cos(e3)*sin(e1) - sin(e1)*sin(e2)*sin(e3))*(cos(e4)*(a1 + d4*cos(e2 + e3) + a3*sin(e2 + e3) + a2*sin(e2)) + x5*(sin(e2 + e3)*cos(e5) + cos(e2 + e3)*cos(e4)*sin(e5)) - y5*(sin(e2 + e3)*sin(e5) - cos(e2 + e3)*cos(e4)*cos(e5)))) - 2*m4*((sin(e4)*(cos(e2)*sin(e1)*sin(e3) + cos(e3)*sin(e1)*sin(e2)) + cos(e1)*cos(e4))*(cos(e4)*(a1 + d4*cos(e2 + e3) + a3*sin(e2 + e3) + a2*sin(e2)) + x4*sin(e2 + e3) + z4*cos(e2 + e3)*cos(e4)) + (cos(e2)*cos(e3)*sin(e1) - sin(e1)*sin(e2)*sin(e3))*(y4*cos(e2 + e3)*cos(e4) + x4*cos(e2 + e3)*sin(e4)) + (cos(e1)*sin(e4) - cos(e4)*(cos(e2)*sin(e1)*sin(e3) + cos(e3)*sin(e1)*sin(e2)))*(sin(e4)*(a1 + d4*cos(e2 + e3) + a3*sin(e2 + e3) + a2*sin(e2)) - y4*sin(e2 + e3) + z4*cos(e2 + e3)*sin(e4)))*((cos(e2)*sin(e1)*sin(e3) + cos(e3)*sin(e1)*sin(e2))*(y4*cos(e2 + e3)*cos(e4) + x4*cos(e2 + e3)*sin(e4)) - (sin(e4)*(cos(e2)*sin(e1)*sin(e3) + cos(e3)*sin(e1)*sin(e2)) + cos(e1)*cos(e4))*(cos(e4)*(a3*cos(e2 + e3) - d4*sin(e2 + e3)) + x4*cos(e2 + e3) - z4*sin(e2 + e3)*cos(e4)) + (cos(e1)*sin(e4) - cos(e4)*(cos(e2)*sin(e1)*sin(e3) + cos(e3)*sin(e1)*sin(e2)))*(y4*cos(e2 + e3) - sin(e4)*(a3*cos(e2 + e3) - d4*sin(e2 + e3)) + z4*sin(e2 + e3)*sin(e4)) + (cos(e2)*cos(e3)*sin(e1) - sin(e1)*sin(e2)*sin(e3))*(y4*sin(e2 + e3)*cos(e4) + x4*sin(e2 + e3)*sin(e4)) - sin(e4)*(cos(e2)*cos(e3)*sin(e1) - sin(e1)*sin(e2)*sin(e3))*(cos(e4)*(a1 + d4*cos(e2 + e3) + a3*sin(e2 + e3) + a2*sin(e2)) + x4*sin(e2 + e3) + z4*cos(e2 + e3)*cos(e4)) + cos(e4)*(cos(e2)*cos(e3)*sin(e1) - sin(e1)*sin(e2)*sin(e3))*(sin(e4)*(a1 + d4*cos(e2 + e3) + a3*sin(e2 + e3) + a2*sin(e2)) - y4*sin(e2 + e3) + z4*cos(e2 + e3)*sin(e4))) - 2*m6*((sin(e6)*(sin(e5)*(cos(e2)*cos(e3)*sin(e1) - sin(e1)*sin(e2)*sin(e3)) - cos(e5)*(cos(e1)*sin(e4) - cos(e4)*(cos(e2)*sin(e1)*sin(e3) + cos(e3)*sin(e1)*sin(e2)))) + cos(e6)*(sin(e4)*(cos(e2)*sin(e1)*sin(e3) + cos(e3)*sin(e1)*sin(e2)) + cos(e1)*cos(e4)))*(x6*(sin(e2 + e3)*cos(e5) + cos(e2 + e3)*cos(e4)*sin(e5)) - z6*(cos(e6)*(sin(e2 + e3)*sin(e5) - cos(e2 + e3)*cos(e4)*cos(e5)) + cos(e2 + e3)*sin(e4)*sin(e6)) + cos(e4)*cos(e6)*(a1 + d4*cos(e2 + e3) + a3*sin(e2 + e3) + a2*sin(e2)) - cos(e5)*sin(e4)*sin(e6)*(a1 + d4*cos(e2 + e3) + a3*sin(e2 + e3) + a2*sin(e2))) + (cos(e6)*(sin(e5)*(cos(e2)*cos(e3)*sin(e1) - sin(e1)*sin(e2)*sin(e3)) - cos(e5)*(cos(e1)*sin(e4) - cos(e4)*(cos(e2)*sin(e1)*sin(e3) + cos(e3)*sin(e1)*sin(e2)))) - sin(e6)*(sin(e4)*(cos(e2)*sin(e1)*sin(e3) + cos(e3)*sin(e1)*sin(e2)) + cos(e1)*cos(e4)))*(y6*(sin(e2 + e3)*cos(e5) + cos(e2 + e3)*cos(e4)*sin(e5)) + z6*(sin(e6)*(sin(e2 + e3)*sin(e5) - cos(e2 + e3)*cos(e4)*cos(e5)) - cos(e2 + e3)*cos(e6)*sin(e4)) - cos(e4)*sin(e6)*(a1 + d4*cos(e2 + e3) + a3*sin(e2 + e3) + a2*sin(e2)) - cos(e5)*cos(e6)*sin(e4)*(a1 + d4*cos(e2 + e3) + a3*sin(e2 + e3) + a2*sin(e2))) - (cos(e5)*(cos(e2)*cos(e3)*sin(e1) - sin(e1)*sin(e2)*sin(e3)) + sin(e5)*(cos(e1)*sin(e4) - cos(e4)*(cos(e2)*sin(e1)*sin(e3) + cos(e3)*sin(e1)*sin(e2))))*(x6*(sin(e6)*(sin(e2 + e3)*sin(e5) - cos(e2 + e3)*cos(e4)*cos(e5)) - cos(e2 + e3)*cos(e6)*sin(e4)) + y6*(cos(e6)*(sin(e2 + e3)*sin(e5) - cos(e2 + e3)*cos(e4)*cos(e5)) + cos(e2 + e3)*sin(e4)*sin(e6)) - sin(e4)*sin(e5)*(a1 + d4*cos(e2 + e3) + a3*sin(e2 + e3) + a2*sin(e2))))*((sin(e6)*(sin(e5)*(cos(e2)*sin(e1)*sin(e3) + cos(e3)*sin(e1)*sin(e2)) - cos(e4)*cos(e5)*(cos(e2)*cos(e3)*sin(e1) - sin(e1)*sin(e2)*sin(e3))) - cos(e6)*sin(e4)*(cos(e2)*cos(e3)*sin(e1) - sin(e1)*sin(e2)*sin(e3)))*(x6*(sin(e2 + e3)*cos(e5) + cos(e2 + e3)*cos(e4)*sin(e5)) - z6*(cos(e6)*(sin(e2 + e3)*sin(e5) - cos(e2 + e3)*cos(e4)*cos(e5)) + cos(e2 + e3)*sin(e4)*sin(e6)) + cos(e4)*cos(e6)*(a1 + d4*cos(e2 + e3) + a3*sin(e2 + e3) + a2*sin(e2)) - cos(e5)*sin(e4)*sin(e6)*(a1 + d4*cos(e2 + e3) + a3*sin(e2 + e3) + a2*sin(e2))) + (cos(e6)*(sin(e5)*(cos(e2)*sin(e1)*sin(e3) + cos(e3)*sin(e1)*sin(e2)) - cos(e4)*cos(e5)*(cos(e2)*cos(e3)*sin(e1) - sin(e1)*sin(e2)*sin(e3))) + sin(e4)*sin(e6)*(cos(e2)*cos(e3)*sin(e1) - sin(e1)*sin(e2)*sin(e3)))*(y6*(sin(e2 + e3)*cos(e5) + cos(e2 + e3)*cos(e4)*sin(e5)) + z6*(sin(e6)*(sin(e2 + e3)*sin(e5) - cos(e2 + e3)*cos(e4)*cos(e5)) - cos(e2 + e3)*cos(e6)*sin(e4)) - cos(e4)*sin(e6)*(a1 + d4*cos(e2 + e3) + a3*sin(e2 + e3) + a2*sin(e2)) - cos(e5)*cos(e6)*sin(e4)*(a1 + d4*cos(e2 + e3) + a3*sin(e2 + e3) + a2*sin(e2))) - (sin(e6)*(sin(e5)*(cos(e2)*cos(e3)*sin(e1) - sin(e1)*sin(e2)*sin(e3)) - cos(e5)*(cos(e1)*sin(e4) - cos(e4)*(cos(e2)*sin(e1)*sin(e3) + cos(e3)*sin(e1)*sin(e2)))) + cos(e6)*(sin(e4)*(cos(e2)*sin(e1)*sin(e3) + cos(e3)*sin(e1)*sin(e2)) + cos(e1)*cos(e4)))*(x6*(cos(e2 + e3)*cos(e5) - sin(e2 + e3)*cos(e4)*sin(e5)) - z6*(cos(e6)*(cos(e2 + e3)*sin(e5) + sin(e2 + e3)*cos(e4)*cos(e5)) - sin(e2 + e3)*sin(e4)*sin(e6)) + cos(e4)*cos(e6)*(a3*cos(e2 + e3) - d4*sin(e2 + e3)) - cos(e5)*sin(e4)*sin(e6)*(a3*cos(e2 + e3) - d4*sin(e2 + e3))) - (cos(e6)*(sin(e5)*(cos(e2)*cos(e3)*sin(e1) - sin(e1)*sin(e2)*sin(e3)) - cos(e5)*(cos(e1)*sin(e4) - cos(e4)*(cos(e2)*sin(e1)*sin(e3) + cos(e3)*sin(e1)*sin(e2)))) - sin(e6)*(sin(e4)*(cos(e2)*sin(e1)*sin(e3) + cos(e3)*sin(e1)*sin(e2)) + cos(e1)*cos(e4)))*(y6*(cos(e2 + e3)*cos(e5) - sin(e2 + e3)*cos(e4)*sin(e5)) + z6*(sin(e6)*(cos(e2 + e3)*sin(e5) + sin(e2 + e3)*cos(e4)*cos(e5)) + sin(e2 + e3)*cos(e6)*sin(e4)) - cos(e4)*sin(e6)*(a3*cos(e2 + e3) - d4*sin(e2 + e3)) - cos(e5)*cos(e6)*sin(e4)*(a3*cos(e2 + e3) - d4*sin(e2 + e3))) + (cos(e5)*(cos(e2)*cos(e3)*sin(e1) - sin(e1)*sin(e2)*sin(e3)) + sin(e5)*(cos(e1)*sin(e4) - cos(e4)*(cos(e2)*sin(e1)*sin(e3) + cos(e3)*sin(e1)*sin(e2))))*(x6*(sin(e6)*(cos(e2 + e3)*sin(e5) + sin(e2 + e3)*cos(e4)*cos(e5)) + sin(e2 + e3)*cos(e6)*sin(e4)) + y6*(cos(e6)*(cos(e2 + e3)*sin(e5) + sin(e2 + e3)*cos(e4)*cos(e5)) - sin(e2 + e3)*sin(e4)*sin(e6)) - sin(e4)*sin(e5)*(a3*cos(e2 + e3) - d4*sin(e2 + e3))) - (cos(e5)*(cos(e2)*sin(e1)*sin(e3) + cos(e3)*sin(e1)*sin(e2)) + cos(e4)*sin(e5)*(cos(e2)*cos(e3)*sin(e1) - sin(e1)*sin(e2)*sin(e3)))*(x6*(sin(e6)*(sin(e2 + e3)*sin(e5) - cos(e2 + e3)*cos(e4)*cos(e5)) - cos(e2 + e3)*cos(e6)*sin(e4)) + y6*(cos(e6)*(sin(e2 + e3)*sin(e5) - cos(e2 + e3)*cos(e4)*cos(e5)) + cos(e2 + e3)*sin(e4)*sin(e6)) - sin(e4)*sin(e5)*(a1 + d4*cos(e2 + e3) + a3*sin(e2 + e3) + a2*sin(e2)))) + 2*m4*((cos(e4)*sin(e1) - sin(e4)*(cos(e1)*cos(e2)*sin(e3) + cos(e1)*cos(e3)*sin(e2)))*(cos(e4)*(a1 + d4*cos(e2 + e3) + a3*sin(e2 + e3) + a2*sin(e2)) + x4*sin(e2 + e3) + z4*cos(e2 + e3)*cos(e4)) - (y4*cos(e2 + e3)*cos(e4) + x4*cos(e2 + e3)*sin(e4))*(cos(e1)*cos(e2)*cos(e3) - cos(e1)*sin(e2)*sin(e3)) + (sin(e1)*sin(e4) + cos(e4)*(cos(e1)*cos(e2)*sin(e3) + cos(e1)*cos(e3)*sin(e2)))*(sin(e4)*(a1 + d4*cos(e2 + e3) + a3*sin(e2 + e3) + a2*sin(e2)) - y4*sin(e2 + e3) + z4*cos(e2 + e3)*sin(e4)))*((y4*cos(e2 + e3)*cos(e4) + x4*cos(e2 + e3)*sin(e4))*(cos(e1)*cos(e2)*sin(e3) + cos(e1)*cos(e3)*sin(e2)) + (cos(e4)*sin(e1) - sin(e4)*(cos(e1)*cos(e2)*sin(e3) + cos(e1)*cos(e3)*sin(e2)))*(cos(e4)*(a3*cos(e2 + e3) - d4*sin(e2 + e3)) + x4*cos(e2 + e3) - z4*sin(e2 + e3)*cos(e4)) + (y4*sin(e2 + e3)*cos(e4) + x4*sin(e2 + e3)*sin(e4))*(cos(e1)*cos(e2)*cos(e3) - cos(e1)*sin(e2)*sin(e3)) - (sin(e1)*sin(e4) + cos(e4)*(cos(e1)*cos(e2)*sin(e3) + cos(e1)*cos(e3)*sin(e2)))*(y4*cos(e2 + e3) - sin(e4)*(a3*cos(e2 + e3) - d4*sin(e2 + e3)) + z4*sin(e2 + e3)*sin(e4)) - sin(e4)*(cos(e1)*cos(e2)*cos(e3) - cos(e1)*sin(e2)*sin(e3))*(cos(e4)*(a1 + d4*cos(e2 + e3) + a3*sin(e2 + e3) + a2*sin(e2)) + x4*sin(e2 + e3) + z4*cos(e2 + e3)*cos(e4)) + cos(e4)*(cos(e1)*cos(e2)*cos(e3) - cos(e1)*sin(e2)*sin(e3))*(sin(e4)*(a1 + d4*cos(e2 + e3) + a3*sin(e2 + e3) + a2*sin(e2)) - y4*sin(e2 + e3) + z4*cos(e2 + e3)*sin(e4))) - cos(e2 + e3)*cos(e4)*(I4zx*cos(e2 + e3) + I4xx*sin(e2 + e3)*cos(e4) - I4yx*sin(e2 + e3)*sin(e4)) + sin(e2 + e3)*cos(e4)*(I4zx*sin(e2 + e3) + I4yx*cos(e2 + e3)*sin(e4) - I4xx*cos(e2 + e3)*cos(e4)) + cos(e2 + e3)*sin(e4)*(I4zy*cos(e2 + e3) + I4xy*sin(e2 + e3)*cos(e4) - I4yy*sin(e2 + e3)*sin(e4)) - sin(e2 + e3)*sin(e4)*(I4zy*sin(e2 + e3) + I4yy*cos(e2 + e3)*sin(e4) - I4xy*cos(e2 + e3)*cos(e4)) + 2*m5*((cos(e5)*(cos(e2)*sin(e3) + cos(e3)*sin(e2)) - cos(e4)*sin(e5)*(sin(e2)*sin(e3) - cos(e2)*cos(e3)))*(z5*(sin(e2 + e3)*sin(e5) - cos(e2 + e3)*cos(e4)*cos(e5)) + sin(e4)*sin(e5)*(a1 + d4*cos(e2 + e3) + a3*sin(e2 + e3) + a2*sin(e2)) + x5*cos(e2 + e3)*sin(e4)) - (sin(e5)*(cos(e2)*sin(e3) + cos(e3)*sin(e2)) + cos(e4)*cos(e5)*(sin(e2)*sin(e3) - cos(e2)*cos(e3)))*(z5*(sin(e2 + e3)*cos(e5) + cos(e2 + e3)*cos(e4)*sin(e5)) + cos(e5)*sin(e4)*(a1 + d4*cos(e2 + e3) + a3*sin(e2 + e3) + a2*sin(e2)) + y5*cos(e2 + e3)*sin(e4)) + sin(e4)*(sin(e2)*sin(e3) - cos(e2)*cos(e3))*(cos(e4)*(a1 + d4*cos(e2 + e3) + a3*sin(e2 + e3) + a2*sin(e2)) + x5*(sin(e2 + e3)*cos(e5) + cos(e2 + e3)*cos(e4)*sin(e5)) - y5*(sin(e2 + e3)*sin(e5) - cos(e2 + e3)*cos(e4)*cos(e5))))*((sin(e5)*(sin(e2)*sin(e3) - cos(e2)*cos(e3)) - cos(e4)*cos(e5)*(cos(e2)*sin(e3) + cos(e3)*sin(e2)))*(z5*(sin(e2 + e3)*cos(e5) + cos(e2 + e3)*cos(e4)*sin(e5)) + cos(e5)*sin(e4)*(a1 + d4*cos(e2 + e3) + a3*sin(e2 + e3) + a2*sin(e2)) + y5*cos(e2 + e3)*sin(e4)) - (cos(e5)*(sin(e2)*sin(e3) - cos(e2)*cos(e3)) + cos(e4)*sin(e5)*(cos(e2)*sin(e3) + cos(e3)*sin(e2)))*(z5*(sin(e2 + e3)*sin(e5) - cos(e2 + e3)*cos(e4)*cos(e5)) + sin(e4)*sin(e5)*(a1 + d4*cos(e2 + e3) + a3*sin(e2 + e3) + a2*sin(e2)) + x5*cos(e2 + e3)*sin(e4)) - (sin(e5)*(cos(e2)*sin(e3) + cos(e3)*sin(e2)) + cos(e4)*cos(e5)*(sin(e2)*sin(e3) - cos(e2)*cos(e3)))*(z5*(cos(e2 + e3)*cos(e5) - sin(e2 + e3)*cos(e4)*sin(e5)) + cos(e5)*sin(e4)*(a3*cos(e2 + e3) - d4*sin(e2 + e3)) - y5*sin(e2 + e3)*sin(e4)) + (cos(e5)*(cos(e2)*sin(e3) + cos(e3)*sin(e2)) - cos(e4)*sin(e5)*(sin(e2)*sin(e3) - cos(e2)*cos(e3)))*(z5*(cos(e2 + e3)*sin(e5) + sin(e2 + e3)*cos(e4)*cos(e5)) + sin(e4)*sin(e5)*(a3*cos(e2 + e3) - d4*sin(e2 + e3)) - x5*sin(e2 + e3)*sin(e4)) + sin(e4)*(cos(e2)*sin(e3) + cos(e3)*sin(e2))*(cos(e4)*(a1 + d4*cos(e2 + e3) + a3*sin(e2 + e3) + a2*sin(e2)) + x5*(sin(e2 + e3)*cos(e5) + cos(e2 + e3)*cos(e4)*sin(e5)) - y5*(sin(e2 + e3)*sin(e5) - cos(e2 + e3)*cos(e4)*cos(e5))) + sin(e4)*(sin(e2)*sin(e3) - cos(e2)*cos(e3))*(cos(e4)*(a3*cos(e2 + e3) - d4*sin(e2 + e3)) + x5*(cos(e2 + e3)*cos(e5) - sin(e2 + e3)*cos(e4)*sin(e5)) - y5*(cos(e2 + e3)*sin(e5) + sin(e2 + e3)*cos(e4)*cos(e5)))) - 2*m6*((sin(e6)*(sin(e5)*(cos(e2)*sin(e3) + cos(e3)*sin(e2)) + cos(e4)*cos(e5)*(sin(e2)*sin(e3) - cos(e2)*cos(e3))) + cos(e6)*sin(e4)*(sin(e2)*sin(e3) - cos(e2)*cos(e3)))*(x6*(sin(e2 + e3)*cos(e5) + cos(e2 + e3)*cos(e4)*sin(e5)) - z6*(cos(e6)*(sin(e2 + e3)*sin(e5) - cos(e2 + e3)*cos(e4)*cos(e5)) + cos(e2 + e3)*sin(e4)*sin(e6)) + cos(e4)*cos(e6)*(a1 + d4*cos(e2 + e3) + a3*sin(e2 + e3) + a2*sin(e2)) - cos(e5)*sin(e4)*sin(e6)*(a1 + d4*cos(e2 + e3) + a3*sin(e2 + e3) + a2*sin(e2))) + (cos(e6)*(sin(e5)*(cos(e2)*sin(e3) + cos(e3)*sin(e2)) + cos(e4)*cos(e5)*(sin(e2)*sin(e3) - cos(e2)*cos(e3))) - sin(e4)*sin(e6)*(sin(e2)*sin(e3) - cos(e2)*cos(e3)))*(y6*(sin(e2 + e3)*cos(e5) + cos(e2 + e3)*cos(e4)*sin(e5)) + z6*(sin(e6)*(sin(e2 + e3)*sin(e5) - cos(e2 + e3)*cos(e4)*cos(e5)) - cos(e2 + e3)*cos(e6)*sin(e4)) - cos(e4)*sin(e6)*(a1 + d4*cos(e2 + e3) + a3*sin(e2 + e3) + a2*sin(e2)) - cos(e5)*cos(e6)*sin(e4)*(a1 + d4*cos(e2 + e3) + a3*sin(e2 + e3) + a2*sin(e2))) - (cos(e5)*(cos(e2)*sin(e3) + cos(e3)*sin(e2)) - cos(e4)*sin(e5)*(sin(e2)*sin(e3) - cos(e2)*cos(e3)))*(x6*(sin(e6)*(sin(e2 + e3)*sin(e5) - cos(e2 + e3)*cos(e4)*cos(e5)) - cos(e2 + e3)*cos(e6)*sin(e4)) + y6*(cos(e6)*(sin(e2 + e3)*sin(e5) - cos(e2 + e3)*cos(e4)*cos(e5)) + cos(e2 + e3)*sin(e4)*sin(e6)) - sin(e4)*sin(e5)*(a1 + d4*cos(e2 + e3) + a3*sin(e2 + e3) + a2*sin(e2))))*((sin(e6)*(sin(e5)*(sin(e2)*sin(e3) - cos(e2)*cos(e3)) - cos(e4)*cos(e5)*(cos(e2)*sin(e3) + cos(e3)*sin(e2))) - cos(e6)*sin(e4)*(cos(e2)*sin(e3) + cos(e3)*sin(e2)))*(x6*(sin(e2 + e3)*cos(e5) + cos(e2 + e3)*cos(e4)*sin(e5)) - z6*(cos(e6)*(sin(e2 + e3)*sin(e5) - cos(e2 + e3)*cos(e4)*cos(e5)) + cos(e2 + e3)*sin(e4)*sin(e6)) + cos(e4)*cos(e6)*(a1 + d4*cos(e2 + e3) + a3*sin(e2 + e3) + a2*sin(e2)) - cos(e5)*sin(e4)*sin(e6)*(a1 + d4*cos(e2 + e3) + a3*sin(e2 + e3) + a2*sin(e2))) + (cos(e6)*(sin(e5)*(sin(e2)*sin(e3) - cos(e2)*cos(e3)) - cos(e4)*cos(e5)*(cos(e2)*sin(e3) + cos(e3)*sin(e2))) + sin(e4)*sin(e6)*(cos(e2)*sin(e3) + cos(e3)*sin(e2)))*(y6*(sin(e2 + e3)*cos(e5) + cos(e2 + e3)*cos(e4)*sin(e5)) + z6*(sin(e6)*(sin(e2 + e3)*sin(e5) - cos(e2 + e3)*cos(e4)*cos(e5)) - cos(e2 + e3)*cos(e6)*sin(e4)) - cos(e4)*sin(e6)*(a1 + d4*cos(e2 + e3) + a3*sin(e2 + e3) + a2*sin(e2)) - cos(e5)*cos(e6)*sin(e4)*(a1 + d4*cos(e2 + e3) + a3*sin(e2 + e3) + a2*sin(e2))) - (sin(e6)*(sin(e5)*(cos(e2)*sin(e3) + cos(e3)*sin(e2)) + cos(e4)*cos(e5)*(sin(e2)*sin(e3) - cos(e2)*cos(e3))) + cos(e6)*sin(e4)*(sin(e2)*sin(e3) - cos(e2)*cos(e3)))*(x6*(cos(e2 + e3)*cos(e5) - sin(e2 + e3)*cos(e4)*sin(e5)) - z6*(cos(e6)*(cos(e2 + e3)*sin(e5) + sin(e2 + e3)*cos(e4)*cos(e5)) - sin(e2 + e3)*sin(e4)*sin(e6)) + cos(e4)*cos(e6)*(a3*cos(e2 + e3) - d4*sin(e2 + e3)) - cos(e5)*sin(e4)*sin(e6)*(a3*cos(e2 + e3) - d4*sin(e2 + e3))) - (cos(e6)*(sin(e5)*(cos(e2)*sin(e3) + cos(e3)*sin(e2)) + cos(e4)*cos(e5)*(sin(e2)*sin(e3) - cos(e2)*cos(e3))) - sin(e4)*sin(e6)*(sin(e2)*sin(e3) - cos(e2)*cos(e3)))*(y6*(cos(e2 + e3)*cos(e5) - sin(e2 + e3)*cos(e4)*sin(e5)) + z6*(sin(e6)*(cos(e2 + e3)*sin(e5) + sin(e2 + e3)*cos(e4)*cos(e5)) + sin(e2 + e3)*cos(e6)*sin(e4)) - cos(e4)*sin(e6)*(a3*cos(e2 + e3) - d4*sin(e2 + e3)) - cos(e5)*cos(e6)*sin(e4)*(a3*cos(e2 + e3) - d4*sin(e2 + e3))) - (cos(e5)*(sin(e2)*sin(e3) - cos(e2)*cos(e3)) + cos(e4)*sin(e5)*(cos(e2)*sin(e3) + cos(e3)*sin(e2)))*(x6*(sin(e6)*(sin(e2 + e3)*sin(e5) - cos(e2 + e3)*cos(e4)*cos(e5)) - cos(e2 + e3)*cos(e6)*sin(e4)) + y6*(cos(e6)*(sin(e2 + e3)*sin(e5) - cos(e2 + e3)*cos(e4)*cos(e5)) + cos(e2 + e3)*sin(e4)*sin(e6)) - sin(e4)*sin(e5)*(a1 + d4*cos(e2 + e3) + a3*sin(e2 + e3) + a2*sin(e2))) + (cos(e5)*(cos(e2)*sin(e3) + cos(e3)*sin(e2)) - cos(e4)*sin(e5)*(sin(e2)*sin(e3) - cos(e2)*cos(e3)))*(x6*(sin(e6)*(cos(e2 + e3)*sin(e5) + sin(e2 + e3)*cos(e4)*cos(e5)) + sin(e2 + e3)*cos(e6)*sin(e4)) + y6*(cos(e6)*(cos(e2 + e3)*sin(e5) + sin(e2 + e3)*cos(e4)*cos(e5)) - sin(e2 + e3)*sin(e4)*sin(e6)) - sin(e4)*sin(e5)*(a3*cos(e2 + e3) - d4*sin(e2 + e3)))) + 2*m5*((cos(e4)*sin(e1) - sin(e4)*(cos(e1)*cos(e2)*sin(e3) + cos(e1)*cos(e3)*sin(e2)))*(cos(e4)*(a1 + d4*cos(e2 + e3) + a3*sin(e2 + e3) + a2*sin(e2)) + x5*(sin(e2 + e3)*cos(e5) + cos(e2 + e3)*cos(e4)*sin(e5)) - y5*(sin(e2 + e3)*sin(e5) - cos(e2 + e3)*cos(e4)*cos(e5))) + (sin(e5)*(cos(e1)*cos(e2)*cos(e3) - cos(e1)*sin(e2)*sin(e3)) + cos(e5)*(sin(e1)*sin(e4) + cos(e4)*(cos(e1)*cos(e2)*sin(e3) + cos(e1)*cos(e3)*sin(e2))))*(z5*(sin(e2 + e3)*cos(e5) + cos(e2 + e3)*cos(e4)*sin(e5)) + cos(e5)*sin(e4)*(a1 + d4*cos(e2 + e3) + a3*sin(e2 + e3) + a2*sin(e2)) + y5*cos(e2 + e3)*sin(e4)) - (cos(e5)*(cos(e1)*cos(e2)*cos(e3) - cos(e1)*sin(e2)*sin(e3)) - sin(e5)*(sin(e1)*sin(e4) + cos(e4)*(cos(e1)*cos(e2)*sin(e3) + cos(e1)*cos(e3)*sin(e2))))*(z5*(sin(e2 + e3)*sin(e5) - cos(e2 + e3)*cos(e4)*cos(e5)) + sin(e4)*sin(e5)*(a1 + d4*cos(e2 + e3) + a3*sin(e2 + e3) + a2*sin(e2)) + x5*cos(e2 + e3)*sin(e4)))*((cos(e5)*(cos(e1)*cos(e2)*sin(e3) + cos(e1)*cos(e3)*sin(e2)) + cos(e4)*sin(e5)*(cos(e1)*cos(e2)*cos(e3) - cos(e1)*sin(e2)*sin(e3)))*(z5*(sin(e2 + e3)*sin(e5) - cos(e2 + e3)*cos(e4)*cos(e5)) + sin(e4)*sin(e5)*(a1 + d4*cos(e2 + e3) + a3*sin(e2 + e3) + a2*sin(e2)) + x5*cos(e2 + e3)*sin(e4)) + (cos(e4)*sin(e1) - sin(e4)*(cos(e1)*cos(e2)*sin(e3) + cos(e1)*cos(e3)*sin(e2)))*(cos(e4)*(a3*cos(e2 + e3) - d4*sin(e2 + e3)) + x5*(cos(e2 + e3)*cos(e5) - sin(e2 + e3)*cos(e4)*sin(e5)) - y5*(cos(e2 + e3)*sin(e5) + sin(e2 + e3)*cos(e4)*cos(e5))) + (sin(e5)*(cos(e1)*cos(e2)*cos(e3) - cos(e1)*sin(e2)*sin(e3)) + cos(e5)*(sin(e1)*sin(e4) + cos(e4)*(cos(e1)*cos(e2)*sin(e3) + cos(e1)*cos(e3)*sin(e2))))*(z5*(cos(e2 + e3)*cos(e5) - sin(e2 + e3)*cos(e4)*sin(e5)) + cos(e5)*sin(e4)*(a3*cos(e2 + e3) - d4*sin(e2 + e3)) - y5*sin(e2 + e3)*sin(e4)) - (cos(e5)*(cos(e1)*cos(e2)*cos(e3) - cos(e1)*sin(e2)*sin(e3)) - sin(e5)*(sin(e1)*sin(e4) + cos(e4)*(cos(e1)*cos(e2)*sin(e3) + cos(e1)*cos(e3)*sin(e2))))*(z5*(cos(e2 + e3)*sin(e5) + sin(e2 + e3)*cos(e4)*cos(e5)) + sin(e4)*sin(e5)*(a3*cos(e2 + e3) - d4*sin(e2 + e3)) - x5*sin(e2 + e3)*sin(e4)) - (sin(e5)*(cos(e1)*cos(e2)*sin(e3) + cos(e1)*cos(e3)*sin(e2)) - cos(e4)*cos(e5)*(cos(e1)*cos(e2)*cos(e3) - cos(e1)*sin(e2)*sin(e3)))*(z5*(sin(e2 + e3)*cos(e5) + cos(e2 + e3)*cos(e4)*sin(e5)) + cos(e5)*sin(e4)*(a1 + d4*cos(e2 + e3) + a3*sin(e2 + e3) + a2*sin(e2)) + y5*cos(e2 + e3)*sin(e4)) - sin(e4)*(cos(e1)*cos(e2)*cos(e3) - cos(e1)*sin(e2)*sin(e3))*(cos(e4)*(a1 + d4*cos(e2 + e3) + a3*sin(e2 + e3) + a2*sin(e2)) + x5*(sin(e2 + e3)*cos(e5) + cos(e2 + e3)*cos(e4)*sin(e5)) - y5*(sin(e2 + e3)*sin(e5) - cos(e2 + e3)*cos(e4)*cos(e5)))) - cos(e2 + e3)*sin(e4)*(I5xz*(cos(e2 + e3)*sin(e5) + sin(e2 + e3)*cos(e4)*cos(e5)) + I5yz*(cos(e2 + e3)*cos(e5) - sin(e2 + e3)*cos(e4)*sin(e5)) + I5zz*sin(e2 + e3)*sin(e4)) + sin(e2 + e3)*sin(e4)*(I5xz*(sin(e2 + e3)*sin(e5) - cos(e2 + e3)*cos(e4)*cos(e5)) + I5yz*(sin(e2 + e3)*cos(e5) + cos(e2 + e3)*cos(e4)*sin(e5)) - I5zz*cos(e2 + e3)*sin(e4)) + 2*m3*sin(e1)*(x3*cos(e2 + e3) - y3*sin(e2 + e3))*(sin(e1)*(a1 + y3*cos(e2 + e3) + x3*sin(e2 + e3) + a2*sin(e2)) + z3*cos(e2 + e3)^2*cos(e1) + z3*sin(e2 + e3)^2*cos(e1)) - 2*m3*cos(e1)*(x3*cos(e2 + e3) - y3*sin(e2 + e3))*(z3*cos(e2 + e3)^2*sin(e1) - cos(e1)*(a1 + y3*cos(e2 + e3) + x3*sin(e2 + e3) + a2*sin(e2)) + z3*sin(e2 + e3)^2*sin(e1))) + de4*((sin(e2 + e3)*cos(e5) + cos(e2 + e3)*cos(e4)*sin(e5))*(I6xz*(cos(e2 + e3)*cos(e4)*sin(e6) + cos(e2 + e3)*cos(e5)*cos(e6)*sin(e4)) + I6yz*(cos(e2 + e3)*cos(e4)*cos(e6) - cos(e2 + e3)*cos(e5)*sin(e4)*sin(e6)) - I6zz*cos(e2 + e3)*sin(e4)*sin(e5)) - (sin(e2 + e3)*cos(e5) + cos(e2 + e3)*cos(e4)*sin(e5))*(I5zy*cos(e2 + e3)*cos(e4) - I5xy*cos(e2 + e3)*cos(e5)*sin(e4) + I5yy*cos(e2 + e3)*sin(e4)*sin(e5)) - (sin(e2 + e3)*sin(e5) - cos(e2 + e3)*cos(e4)*cos(e5))*(I5zx*cos(e2 + e3)*cos(e4) - I5xx*cos(e2 + e3)*cos(e5)*sin(e4) + I5yx*cos(e2 + e3)*sin(e4)*sin(e5)) + (cos(e6)*(sin(e2 + e3)*sin(e5) - cos(e2 + e3)*cos(e4)*cos(e5)) + cos(e2 + e3)*sin(e4)*sin(e6))*(I6xx*(cos(e2 + e3)*cos(e4)*sin(e6) + cos(e2 + e3)*cos(e5)*cos(e6)*sin(e4)) + I6yx*(cos(e2 + e3)*cos(e4)*cos(e6) - cos(e2 + e3)*cos(e5)*sin(e4)*sin(e6)) - I6zx*cos(e2 + e3)*sin(e4)*sin(e5)) - (sin(e6)*(sin(e2 + e3)*sin(e5) - cos(e2 + e3)*cos(e4)*cos(e5)) - cos(e2 + e3)*cos(e6)*sin(e4))*(I6xy*(cos(e2 + e3)*cos(e4)*sin(e6) + cos(e2 + e3)*cos(e5)*cos(e6)*sin(e4)) + I6yy*(cos(e2 + e3)*cos(e4)*cos(e6) - cos(e2 + e3)*cos(e5)*sin(e4)*sin(e6)) - I6zy*cos(e2 + e3)*sin(e4)*sin(e5)) + (cos(e2 + e3)*cos(e4)*sin(e6) + cos(e2 + e3)*cos(e5)*cos(e6)*sin(e4))*(I6zx*(sin(e2 + e3)*cos(e5) + cos(e2 + e3)*cos(e4)*sin(e5)) + I6xx*(cos(e6)*(sin(e2 + e3)*sin(e5) - cos(e2 + e3)*cos(e4)*cos(e5)) + cos(e2 + e3)*sin(e4)*sin(e6)) - I6yx*(sin(e6)*(sin(e2 + e3)*sin(e5) - cos(e2 + e3)*cos(e4)*cos(e5)) - cos(e2 + e3)*cos(e6)*sin(e4))) + (cos(e2 + e3)*cos(e4)*cos(e6) - cos(e2 + e3)*cos(e5)*sin(e4)*sin(e6))*(I6zy*(sin(e2 + e3)*cos(e5) + cos(e2 + e3)*cos(e4)*sin(e5)) + I6xy*(cos(e6)*(sin(e2 + e3)*sin(e5) - cos(e2 + e3)*cos(e4)*cos(e5)) + cos(e2 + e3)*sin(e4)*sin(e6)) - I6yy*(sin(e6)*(sin(e2 + e3)*sin(e5) - cos(e2 + e3)*cos(e4)*cos(e5)) - cos(e2 + e3)*cos(e6)*sin(e4))) + sin(e2 + e3)*(I4xz*cos(e2 + e3)*sin(e4) + I4yz*cos(e2 + e3)*cos(e4)) - 2*m6*((sin(e6)*(sin(e5)*(cos(e2)*sin(e3) + cos(e3)*sin(e2)) + cos(e4)*cos(e5)*(sin(e2)*sin(e3) - cos(e2)*cos(e3))) + cos(e6)*sin(e4)*(sin(e2)*sin(e3) - cos(e2)*cos(e3)))*(x6*(sin(e2 + e3)*cos(e5) + cos(e2 + e3)*cos(e4)*sin(e5)) - z6*(cos(e6)*(sin(e2 + e3)*sin(e5) - cos(e2 + e3)*cos(e4)*cos(e5)) + cos(e2 + e3)*sin(e4)*sin(e6)) + cos(e4)*cos(e6)*(a1 + d4*cos(e2 + e3) + a3*sin(e2 + e3) + a2*sin(e2)) - cos(e5)*sin(e4)*sin(e6)*(a1 + d4*cos(e2 + e3) + a3*sin(e2 + e3) + a2*sin(e2))) + (cos(e6)*(sin(e5)*(cos(e2)*sin(e3) + cos(e3)*sin(e2)) + cos(e4)*cos(e5)*(sin(e2)*sin(e3) - cos(e2)*cos(e3))) - sin(e4)*sin(e6)*(sin(e2)*sin(e3) - cos(e2)*cos(e3)))*(y6*(sin(e2 + e3)*cos(e5) + cos(e2 + e3)*cos(e4)*sin(e5)) + z6*(sin(e6)*(sin(e2 + e3)*sin(e5) - cos(e2 + e3)*cos(e4)*cos(e5)) - cos(e2 + e3)*cos(e6)*sin(e4)) - cos(e4)*sin(e6)*(a1 + d4*cos(e2 + e3) + a3*sin(e2 + e3) + a2*sin(e2)) - cos(e5)*cos(e6)*sin(e4)*(a1 + d4*cos(e2 + e3) + a3*sin(e2 + e3) + a2*sin(e2))) - (cos(e5)*(cos(e2)*sin(e3) + cos(e3)*sin(e2)) - cos(e4)*sin(e5)*(sin(e2)*sin(e3) - cos(e2)*cos(e3)))*(x6*(sin(e6)*(sin(e2 + e3)*sin(e5) - cos(e2 + e3)*cos(e4)*cos(e5)) - cos(e2 + e3)*cos(e6)*sin(e4)) + y6*(cos(e6)*(sin(e2 + e3)*sin(e5) - cos(e2 + e3)*cos(e4)*cos(e5)) + cos(e2 + e3)*sin(e4)*sin(e6)) - sin(e4)*sin(e5)*(a1 + d4*cos(e2 + e3) + a3*sin(e2 + e3) + a2*sin(e2))))*((sin(e6)*(sin(e5)*(cos(e2)*sin(e3) + cos(e3)*sin(e2)) + cos(e4)*cos(e5)*(sin(e2)*sin(e3) - cos(e2)*cos(e3))) + cos(e6)*sin(e4)*(sin(e2)*sin(e3) - cos(e2)*cos(e3)))*(z6*(cos(e2 + e3)*cos(e4)*sin(e6) + cos(e2 + e3)*cos(e5)*cos(e6)*sin(e4)) + cos(e6)*sin(e4)*(a1 + d4*cos(e2 + e3) + a3*sin(e2 + e3) + a2*sin(e2)) + x6*cos(e2 + e3)*sin(e4)*sin(e5) + cos(e4)*cos(e5)*sin(e6)*(a1 + d4*cos(e2 + e3) + a3*sin(e2 + e3) + a2*sin(e2))) + (cos(e6)*(sin(e5)*(cos(e2)*sin(e3) + cos(e3)*sin(e2)) + cos(e4)*cos(e5)*(sin(e2)*sin(e3) - cos(e2)*cos(e3))) - sin(e4)*sin(e6)*(sin(e2)*sin(e3) - cos(e2)*cos(e3)))*(z6*(cos(e2 + e3)*cos(e4)*cos(e6) - cos(e2 + e3)*cos(e5)*sin(e4)*sin(e6)) - sin(e4)*sin(e6)*(a1 + d4*cos(e2 + e3) + a3*sin(e2 + e3) + a2*sin(e2)) + y6*cos(e2 + e3)*sin(e4)*sin(e5) + cos(e4)*cos(e5)*cos(e6)*(a1 + d4*cos(e2 + e3) + a3*sin(e2 + e3) + a2*sin(e2))) - (cos(e5)*(cos(e2)*sin(e3) + cos(e3)*sin(e2)) - cos(e4)*sin(e5)*(sin(e2)*sin(e3) - cos(e2)*cos(e3)))*(x6*(cos(e2 + e3)*cos(e4)*cos(e6) - cos(e2 + e3)*cos(e5)*sin(e4)*sin(e6)) - y6*(cos(e2 + e3)*cos(e4)*sin(e6) + cos(e2 + e3)*cos(e5)*cos(e6)*sin(e4)) + cos(e4)*sin(e5)*(a1 + d4*cos(e2 + e3) + a3*sin(e2 + e3) + a2*sin(e2))) - (cos(e4)*cos(e6)*(sin(e2)*sin(e3) - cos(e2)*cos(e3)) - cos(e5)*sin(e4)*sin(e6)*(sin(e2)*sin(e3) - cos(e2)*cos(e3)))*(x6*(sin(e2 + e3)*cos(e5) + cos(e2 + e3)*cos(e4)*sin(e5)) - z6*(cos(e6)*(sin(e2 + e3)*sin(e5) - cos(e2 + e3)*cos(e4)*cos(e5)) + cos(e2 + e3)*sin(e4)*sin(e6)) + cos(e4)*cos(e6)*(a1 + d4*cos(e2 + e3) + a3*sin(e2 + e3) + a2*sin(e2)) - cos(e5)*sin(e4)*sin(e6)*(a1 + d4*cos(e2 + e3) + a3*sin(e2 + e3) + a2*sin(e2))) + (cos(e4)*sin(e6)*(sin(e2)*sin(e3) - cos(e2)*cos(e3)) + cos(e5)*cos(e6)*sin(e4)*(sin(e2)*sin(e3) - cos(e2)*cos(e3)))*(y6*(sin(e2 + e3)*cos(e5) + cos(e2 + e3)*cos(e4)*sin(e5)) + z6*(sin(e6)*(sin(e2 + e3)*sin(e5) - cos(e2 + e3)*cos(e4)*cos(e5)) - cos(e2 + e3)*cos(e6)*sin(e4)) - cos(e4)*sin(e6)*(a1 + d4*cos(e2 + e3) + a3*sin(e2 + e3) + a2*sin(e2)) - cos(e5)*cos(e6)*sin(e4)*(a1 + d4*cos(e2 + e3) + a3*sin(e2 + e3) + a2*sin(e2))) + sin(e4)*sin(e5)*(sin(e2)*sin(e3) - cos(e2)*cos(e3))*(x6*(sin(e6)*(sin(e2 + e3)*sin(e5) - cos(e2 + e3)*cos(e4)*cos(e5)) - cos(e2 + e3)*cos(e6)*sin(e4)) + y6*(cos(e6)*(sin(e2 + e3)*sin(e5) - cos(e2 + e3)*cos(e4)*cos(e5)) + cos(e2 + e3)*sin(e4)*sin(e6)) - sin(e4)*sin(e5)*(a1 + d4*cos(e2 + e3) + a3*sin(e2 + e3) + a2*sin(e2)))) - 2*m5*((cos(e4)*sin(e1) - sin(e4)*(cos(e1)*cos(e2)*sin(e3) + cos(e1)*cos(e3)*sin(e2)))*(cos(e4)*(a1 + d4*cos(e2 + e3) + a3*sin(e2 + e3) + a2*sin(e2)) + x5*(sin(e2 + e3)*cos(e5) + cos(e2 + e3)*cos(e4)*sin(e5)) - y5*(sin(e2 + e3)*sin(e5) - cos(e2 + e3)*cos(e4)*cos(e5))) + (sin(e5)*(cos(e1)*cos(e2)*cos(e3) - cos(e1)*sin(e2)*sin(e3)) + cos(e5)*(sin(e1)*sin(e4) + cos(e4)*(cos(e1)*cos(e2)*sin(e3) + cos(e1)*cos(e3)*sin(e2))))*(z5*(sin(e2 + e3)*cos(e5) + cos(e2 + e3)*cos(e4)*sin(e5)) + cos(e5)*sin(e4)*(a1 + d4*cos(e2 + e3) + a3*sin(e2 + e3) + a2*sin(e2)) + y5*cos(e2 + e3)*sin(e4)) - (cos(e5)*(cos(e1)*cos(e2)*cos(e3) - cos(e1)*sin(e2)*sin(e3)) - sin(e5)*(sin(e1)*sin(e4) + cos(e4)*(cos(e1)*cos(e2)*sin(e3) + cos(e1)*cos(e3)*sin(e2))))*(z5*(sin(e2 + e3)*sin(e5) - cos(e2 + e3)*cos(e4)*cos(e5)) + sin(e4)*sin(e5)*(a1 + d4*cos(e2 + e3) + a3*sin(e2 + e3) + a2*sin(e2)) + x5*cos(e2 + e3)*sin(e4)))*((cos(e5)*(cos(e1)*cos(e2)*cos(e3) - cos(e1)*sin(e2)*sin(e3)) - sin(e5)*(sin(e1)*sin(e4) + cos(e4)*(cos(e1)*cos(e2)*sin(e3) + cos(e1)*cos(e3)*sin(e2))))*(cos(e4)*sin(e5)*(a1 + d4*cos(e2 + e3) + a3*sin(e2 + e3) + a2*sin(e2)) + x5*cos(e2 + e3)*cos(e4) + z5*cos(e2 + e3)*cos(e5)*sin(e4)) - (sin(e5)*(cos(e1)*cos(e2)*cos(e3) - cos(e1)*sin(e2)*sin(e3)) + cos(e5)*(sin(e1)*sin(e4) + cos(e4)*(cos(e1)*cos(e2)*sin(e3) + cos(e1)*cos(e3)*sin(e2))))*(y5*cos(e2 + e3)*cos(e4) + cos(e4)*cos(e5)*(a1 + d4*cos(e2 + e3) + a3*sin(e2 + e3) + a2*sin(e2)) - z5*cos(e2 + e3)*sin(e4)*sin(e5)) + (sin(e1)*sin(e4) + cos(e4)*(cos(e1)*cos(e2)*sin(e3) + cos(e1)*cos(e3)*sin(e2)))*(cos(e4)*(a1 + d4*cos(e2 + e3) + a3*sin(e2 + e3) + a2*sin(e2)) + x5*(sin(e2 + e3)*cos(e5) + cos(e2 + e3)*cos(e4)*sin(e5)) - y5*(sin(e2 + e3)*sin(e5) - cos(e2 + e3)*cos(e4)*cos(e5))) + (cos(e4)*sin(e1) - sin(e4)*(cos(e1)*cos(e2)*sin(e3) + cos(e1)*cos(e3)*sin(e2)))*(sin(e4)*(a1 + d4*cos(e2 + e3) + a3*sin(e2 + e3) + a2*sin(e2)) + y5*cos(e2 + e3)*cos(e5)*sin(e4) + x5*cos(e2 + e3)*sin(e4)*sin(e5)) - cos(e5)*(cos(e4)*sin(e1) - sin(e4)*(cos(e1)*cos(e2)*sin(e3) + cos(e1)*cos(e3)*sin(e2)))*(z5*(sin(e2 + e3)*cos(e5) + cos(e2 + e3)*cos(e4)*sin(e5)) + cos(e5)*sin(e4)*(a1 + d4*cos(e2 + e3) + a3*sin(e2 + e3) + a2*sin(e2)) + y5*cos(e2 + e3)*sin(e4)) - sin(e5)*(cos(e4)*sin(e1) - sin(e4)*(cos(e1)*cos(e2)*sin(e3) + cos(e1)*cos(e3)*sin(e2)))*(z5*(sin(e2 + e3)*sin(e5) - cos(e2 + e3)*cos(e4)*cos(e5)) + sin(e4)*sin(e5)*(a1 + d4*cos(e2 + e3) + a3*sin(e2 + e3) + a2*sin(e2)) + x5*cos(e2 + e3)*sin(e4))) - cos(e2 + e3)*cos(e4)*(I4xx*cos(e2 + e3)*sin(e4) + I4yx*cos(e2 + e3)*cos(e4)) + 2*m5*((cos(e5)*(cos(e2)*cos(e3)*sin(e1) - sin(e1)*sin(e2)*sin(e3)) + sin(e5)*(cos(e1)*sin(e4) - cos(e4)*(cos(e2)*sin(e1)*sin(e3) + cos(e3)*sin(e1)*sin(e2))))*(z5*(sin(e2 + e3)*sin(e5) - cos(e2 + e3)*cos(e4)*cos(e5)) + sin(e4)*sin(e5)*(a1 + d4*cos(e2 + e3) + a3*sin(e2 + e3) + a2*sin(e2)) + x5*cos(e2 + e3)*sin(e4)) + (sin(e4)*(cos(e2)*sin(e1)*sin(e3) + cos(e3)*sin(e1)*sin(e2)) + cos(e1)*cos(e4))*(cos(e4)*(a1 + d4*cos(e2 + e3) + a3*sin(e2 + e3) + a2*sin(e2)) + x5*(sin(e2 + e3)*cos(e5) + cos(e2 + e3)*cos(e4)*sin(e5)) - y5*(sin(e2 + e3)*sin(e5) - cos(e2 + e3)*cos(e4)*cos(e5))) - (sin(e5)*(cos(e2)*cos(e3)*sin(e1) - sin(e1)*sin(e2)*sin(e3)) - cos(e5)*(cos(e1)*sin(e4) - cos(e4)*(cos(e2)*sin(e1)*sin(e3) + cos(e3)*sin(e1)*sin(e2))))*(z5*(sin(e2 + e3)*cos(e5) + cos(e2 + e3)*cos(e4)*sin(e5)) + cos(e5)*sin(e4)*(a1 + d4*cos(e2 + e3) + a3*sin(e2 + e3) + a2*sin(e2)) + y5*cos(e2 + e3)*sin(e4)))*((cos(e5)*(cos(e2)*cos(e3)*sin(e1) - sin(e1)*sin(e2)*sin(e3)) + sin(e5)*(cos(e1)*sin(e4) - cos(e4)*(cos(e2)*sin(e1)*sin(e3) + cos(e3)*sin(e1)*sin(e2))))*(cos(e4)*sin(e5)*(a1 + d4*cos(e2 + e3) + a3*sin(e2 + e3) + a2*sin(e2)) + x5*cos(e2 + e3)*cos(e4) + z5*cos(e2 + e3)*cos(e5)*sin(e4)) - (sin(e5)*(cos(e2)*cos(e3)*sin(e1) - sin(e1)*sin(e2)*sin(e3)) - cos(e5)*(cos(e1)*sin(e4) - cos(e4)*(cos(e2)*sin(e1)*sin(e3) + cos(e3)*sin(e1)*sin(e2))))*(y5*cos(e2 + e3)*cos(e4) + cos(e4)*cos(e5)*(a1 + d4*cos(e2 + e3) + a3*sin(e2 + e3) + a2*sin(e2)) - z5*cos(e2 + e3)*sin(e4)*sin(e5)) - (cos(e1)*sin(e4) - cos(e4)*(cos(e2)*sin(e1)*sin(e3) + cos(e3)*sin(e1)*sin(e2)))*(cos(e4)*(a1 + d4*cos(e2 + e3) + a3*sin(e2 + e3) + a2*sin(e2)) + x5*(sin(e2 + e3)*cos(e5) + cos(e2 + e3)*cos(e4)*sin(e5)) - y5*(sin(e2 + e3)*sin(e5) - cos(e2 + e3)*cos(e4)*cos(e5))) - (sin(e4)*(cos(e2)*sin(e1)*sin(e3) + cos(e3)*sin(e1)*sin(e2)) + cos(e1)*cos(e4))*(sin(e4)*(a1 + d4*cos(e2 + e3) + a3*sin(e2 + e3) + a2*sin(e2)) + y5*cos(e2 + e3)*cos(e5)*sin(e4) + x5*cos(e2 + e3)*sin(e4)*sin(e5)) + sin(e5)*(sin(e4)*(cos(e2)*sin(e1)*sin(e3) + cos(e3)*sin(e1)*sin(e2)) + cos(e1)*cos(e4))*(z5*(sin(e2 + e3)*sin(e5) - cos(e2 + e3)*cos(e4)*cos(e5)) + sin(e4)*sin(e5)*(a1 + d4*cos(e2 + e3) + a3*sin(e2 + e3) + a2*sin(e2)) + x5*cos(e2 + e3)*sin(e4)) + cos(e5)*(sin(e4)*(cos(e2)*sin(e1)*sin(e3) + cos(e3)*sin(e1)*sin(e2)) + cos(e1)*cos(e4))*(z5*(sin(e2 + e3)*cos(e5) + cos(e2 + e3)*cos(e4)*sin(e5)) + cos(e5)*sin(e4)*(a1 + d4*cos(e2 + e3) + a3*sin(e2 + e3) + a2*sin(e2)) + y5*cos(e2 + e3)*sin(e4))) + cos(e2 + e3)*sin(e4)*(I4xy*cos(e2 + e3)*sin(e4) + I4yy*cos(e2 + e3)*cos(e4)) - 2*m6*((sin(e6)*(sin(e5)*(cos(e2)*cos(e3)*sin(e1) - sin(e1)*sin(e2)*sin(e3)) - cos(e5)*(cos(e1)*sin(e4) - cos(e4)*(cos(e2)*sin(e1)*sin(e3) + cos(e3)*sin(e1)*sin(e2)))) + cos(e6)*(sin(e4)*(cos(e2)*sin(e1)*sin(e3) + cos(e3)*sin(e1)*sin(e2)) + cos(e1)*cos(e4)))*(x6*(sin(e2 + e3)*cos(e5) + cos(e2 + e3)*cos(e4)*sin(e5)) - z6*(cos(e6)*(sin(e2 + e3)*sin(e5) - cos(e2 + e3)*cos(e4)*cos(e5)) + cos(e2 + e3)*sin(e4)*sin(e6)) + cos(e4)*cos(e6)*(a1 + d4*cos(e2 + e3) + a3*sin(e2 + e3) + a2*sin(e2)) - cos(e5)*sin(e4)*sin(e6)*(a1 + d4*cos(e2 + e3) + a3*sin(e2 + e3) + a2*sin(e2))) + (cos(e6)*(sin(e5)*(cos(e2)*cos(e3)*sin(e1) - sin(e1)*sin(e2)*sin(e3)) - cos(e5)*(cos(e1)*sin(e4) - cos(e4)*(cos(e2)*sin(e1)*sin(e3) + cos(e3)*sin(e1)*sin(e2)))) - sin(e6)*(sin(e4)*(cos(e2)*sin(e1)*sin(e3) + cos(e3)*sin(e1)*sin(e2)) + cos(e1)*cos(e4)))*(y6*(sin(e2 + e3)*cos(e5) + cos(e2 + e3)*cos(e4)*sin(e5)) + z6*(sin(e6)*(sin(e2 + e3)*sin(e5) - cos(e2 + e3)*cos(e4)*cos(e5)) - cos(e2 + e3)*cos(e6)*sin(e4)) - cos(e4)*sin(e6)*(a1 + d4*cos(e2 + e3) + a3*sin(e2 + e3) + a2*sin(e2)) - cos(e5)*cos(e6)*sin(e4)*(a1 + d4*cos(e2 + e3) + a3*sin(e2 + e3) + a2*sin(e2))) - (cos(e5)*(cos(e2)*cos(e3)*sin(e1) - sin(e1)*sin(e2)*sin(e3)) + sin(e5)*(cos(e1)*sin(e4) - cos(e4)*(cos(e2)*sin(e1)*sin(e3) + cos(e3)*sin(e1)*sin(e2))))*(x6*(sin(e6)*(sin(e2 + e3)*sin(e5) - cos(e2 + e3)*cos(e4)*cos(e5)) - cos(e2 + e3)*cos(e6)*sin(e4)) + y6*(cos(e6)*(sin(e2 + e3)*sin(e5) - cos(e2 + e3)*cos(e4)*cos(e5)) + cos(e2 + e3)*sin(e4)*sin(e6)) - sin(e4)*sin(e5)*(a1 + d4*cos(e2 + e3) + a3*sin(e2 + e3) + a2*sin(e2))))*((cos(e6)*(cos(e1)*sin(e4) - cos(e4)*(cos(e2)*sin(e1)*sin(e3) + cos(e3)*sin(e1)*sin(e2))) + cos(e5)*sin(e6)*(sin(e4)*(cos(e2)*sin(e1)*sin(e3) + cos(e3)*sin(e1)*sin(e2)) + cos(e1)*cos(e4)))*(x6*(sin(e2 + e3)*cos(e5) + cos(e2 + e3)*cos(e4)*sin(e5)) - z6*(cos(e6)*(sin(e2 + e3)*sin(e5) - cos(e2 + e3)*cos(e4)*cos(e5)) + cos(e2 + e3)*sin(e4)*sin(e6)) + cos(e4)*cos(e6)*(a1 + d4*cos(e2 + e3) + a3*sin(e2 + e3) + a2*sin(e2)) - cos(e5)*sin(e4)*sin(e6)*(a1 + d4*cos(e2 + e3) + a3*sin(e2 + e3) + a2*sin(e2))) - (cos(e5)*(cos(e2)*cos(e3)*sin(e1) - sin(e1)*sin(e2)*sin(e3)) + sin(e5)*(cos(e1)*sin(e4) - cos(e4)*(cos(e2)*sin(e1)*sin(e3) + cos(e3)*sin(e1)*sin(e2))))*(x6*(cos(e2 + e3)*cos(e4)*cos(e6) - cos(e2 + e3)*cos(e5)*sin(e4)*sin(e6)) - y6*(cos(e2 + e3)*cos(e4)*sin(e6) + cos(e2 + e3)*cos(e5)*cos(e6)*sin(e4)) + cos(e4)*sin(e5)*(a1 + d4*cos(e2 + e3) + a3*sin(e2 + e3) + a2*sin(e2))) + (sin(e6)*(sin(e5)*(cos(e2)*cos(e3)*sin(e1) - sin(e1)*sin(e2)*sin(e3)) - cos(e5)*(cos(e1)*sin(e4) - cos(e4)*(cos(e2)*sin(e1)*sin(e3) + cos(e3)*sin(e1)*sin(e2)))) + cos(e6)*(sin(e4)*(cos(e2)*sin(e1)*sin(e3) + cos(e3)*sin(e1)*sin(e2)) + cos(e1)*cos(e4)))*(z6*(cos(e2 + e3)*cos(e4)*sin(e6) + cos(e2 + e3)*cos(e5)*cos(e6)*sin(e4)) + cos(e6)*sin(e4)*(a1 + d4*cos(e2 + e3) + a3*sin(e2 + e3) + a2*sin(e2)) + x6*cos(e2 + e3)*sin(e4)*sin(e5) + cos(e4)*cos(e5)*sin(e6)*(a1 + d4*cos(e2 + e3) + a3*sin(e2 + e3) + a2*sin(e2))) - (sin(e6)*(cos(e1)*sin(e4) - cos(e4)*(cos(e2)*sin(e1)*sin(e3) + cos(e3)*sin(e1)*sin(e2))) - cos(e5)*cos(e6)*(sin(e4)*(cos(e2)*sin(e1)*sin(e3) + cos(e3)*sin(e1)*sin(e2)) + cos(e1)*cos(e4)))*(y6*(sin(e2 + e3)*cos(e5) + cos(e2 + e3)*cos(e4)*sin(e5)) + z6*(sin(e6)*(sin(e2 + e3)*sin(e5) - cos(e2 + e3)*cos(e4)*cos(e5)) - cos(e2 + e3)*cos(e6)*sin(e4)) - cos(e4)*sin(e6)*(a1 + d4*cos(e2 + e3) + a3*sin(e2 + e3) + a2*sin(e2)) - cos(e5)*cos(e6)*sin(e4)*(a1 + d4*cos(e2 + e3) + a3*sin(e2 + e3) + a2*sin(e2))) + (cos(e6)*(sin(e5)*(cos(e2)*cos(e3)*sin(e1) - sin(e1)*sin(e2)*sin(e3)) - cos(e5)*(cos(e1)*sin(e4) - cos(e4)*(cos(e2)*sin(e1)*sin(e3) + cos(e3)*sin(e1)*sin(e2)))) - sin(e6)*(sin(e4)*(cos(e2)*sin(e1)*sin(e3) + cos(e3)*sin(e1)*sin(e2)) + cos(e1)*cos(e4)))*(z6*(cos(e2 + e3)*cos(e4)*cos(e6) - cos(e2 + e3)*cos(e5)*sin(e4)*sin(e6)) - sin(e4)*sin(e6)*(a1 + d4*cos(e2 + e3) + a3*sin(e2 + e3) + a2*sin(e2)) + y6*cos(e2 + e3)*sin(e4)*sin(e5) + cos(e4)*cos(e5)*cos(e6)*(a1 + d4*cos(e2 + e3) + a3*sin(e2 + e3) + a2*sin(e2))) + sin(e5)*(sin(e4)*(cos(e2)*sin(e1)*sin(e3) + cos(e3)*sin(e1)*sin(e2)) + cos(e1)*cos(e4))*(x6*(sin(e6)*(sin(e2 + e3)*sin(e5) - cos(e2 + e3)*cos(e4)*cos(e5)) - cos(e2 + e3)*cos(e6)*sin(e4)) + y6*(cos(e6)*(sin(e2 + e3)*sin(e5) - cos(e2 + e3)*cos(e4)*cos(e5)) + cos(e2 + e3)*sin(e4)*sin(e6)) - sin(e4)*sin(e5)*(a1 + d4*cos(e2 + e3) + a3*sin(e2 + e3) + a2*sin(e2)))) + cos(e2 + e3)*cos(e4)*(I4zy*sin(e2 + e3) + I4yy*cos(e2 + e3)*sin(e4) - I4xy*cos(e2 + e3)*cos(e4)) + 2*m4*((sin(e4)*(cos(e2)*sin(e1)*sin(e3) + cos(e3)*sin(e1)*sin(e2)) + cos(e1)*cos(e4))*(cos(e4)*(a1 + d4*cos(e2 + e3) + a3*sin(e2 + e3) + a2*sin(e2)) + x4*sin(e2 + e3) + z4*cos(e2 + e3)*cos(e4)) + (cos(e2)*cos(e3)*sin(e1) - sin(e1)*sin(e2)*sin(e3))*(y4*cos(e2 + e3)*cos(e4) + x4*cos(e2 + e3)*sin(e4)) + (cos(e1)*sin(e4) - cos(e4)*(cos(e2)*sin(e1)*sin(e3) + cos(e3)*sin(e1)*sin(e2)))*(sin(e4)*(a1 + d4*cos(e2 + e3) + a3*sin(e2 + e3) + a2*sin(e2)) - y4*sin(e2 + e3) + z4*cos(e2 + e3)*sin(e4)))*((cos(e2)*cos(e3)*sin(e1) - sin(e1)*sin(e2)*sin(e3))*(x4*cos(e2 + e3)*cos(e4) - y4*cos(e2 + e3)*sin(e4)) - (cos(e1)*sin(e4) - cos(e4)*(cos(e2)*sin(e1)*sin(e3) + cos(e3)*sin(e1)*sin(e2)))*(cos(e4)*(a1 + d4*cos(e2 + e3) + a3*sin(e2 + e3) + a2*sin(e2)) + x4*sin(e2 + e3) + z4*cos(e2 + e3)*cos(e4)) + (sin(e4)*(cos(e2)*sin(e1)*sin(e3) + cos(e3)*sin(e1)*sin(e2)) + cos(e1)*cos(e4))*(sin(e4)*(a1 + d4*cos(e2 + e3) + a3*sin(e2 + e3) + a2*sin(e2)) - y4*sin(e2 + e3) + z4*cos(e2 + e3)*sin(e4)) + (cos(e1)*sin(e4) - cos(e4)*(cos(e2)*sin(e1)*sin(e3) + cos(e3)*sin(e1)*sin(e2)))*(cos(e4)*(a1 + d4*cos(e2 + e3) + a3*sin(e2 + e3) + a2*sin(e2)) + z4*cos(e2 + e3)*cos(e4)) - (sin(e4)*(cos(e2)*sin(e1)*sin(e3) + cos(e3)*sin(e1)*sin(e2)) + cos(e1)*cos(e4))*(sin(e4)*(a1 + d4*cos(e2 + e3) + a3*sin(e2 + e3) + a2*sin(e2)) + z4*cos(e2 + e3)*sin(e4))) + cos(e2 + e3)*sin(e4)*(I4zx*sin(e2 + e3) + I4yx*cos(e2 + e3)*sin(e4) - I4xx*cos(e2 + e3)*cos(e4)) + 2*m4*((cos(e2)*sin(e3) + cos(e3)*sin(e2))*(y4*cos(e2 + e3)*cos(e4) + x4*cos(e2 + e3)*sin(e4)) + sin(e4)*(sin(e2)*sin(e3) - cos(e2)*cos(e3))*(cos(e4)*(a1 + d4*cos(e2 + e3) + a3*sin(e2 + e3) + a2*sin(e2)) + x4*sin(e2 + e3) + z4*cos(e2 + e3)*cos(e4)) - cos(e4)*(sin(e2)*sin(e3) - cos(e2)*cos(e3))*(sin(e4)*(a1 + d4*cos(e2 + e3) + a3*sin(e2 + e3) + a2*sin(e2)) - y4*sin(e2 + e3) + z4*cos(e2 + e3)*sin(e4)))*((cos(e2)*sin(e3) + cos(e3)*sin(e2))*(x4*cos(e2 + e3)*cos(e4) - y4*cos(e2 + e3)*sin(e4)) - cos(e4)*(sin(e2)*sin(e3) - cos(e2)*cos(e3))*(cos(e4)*(a1 + d4*cos(e2 + e3) + a3*sin(e2 + e3) + a2*sin(e2)) + z4*cos(e2 + e3)*cos(e4)) - sin(e4)*(sin(e2)*sin(e3) - cos(e2)*cos(e3))*(sin(e4)*(a1 + d4*cos(e2 + e3) + a3*sin(e2 + e3) + a2*sin(e2)) + z4*cos(e2 + e3)*sin(e4)) + cos(e4)*(sin(e2)*sin(e3) - cos(e2)*cos(e3))*(cos(e4)*(a1 + d4*cos(e2 + e3) + a3*sin(e2 + e3) + a2*sin(e2)) + x4*sin(e2 + e3) + z4*cos(e2 + e3)*cos(e4)) + sin(e4)*(sin(e2)*sin(e3) - cos(e2)*cos(e3))*(sin(e4)*(a1 + d4*cos(e2 + e3) + a3*sin(e2 + e3) + a2*sin(e2)) - y4*sin(e2 + e3) + z4*cos(e2 + e3)*sin(e4))) + 2*m6*((sin(e6)*(sin(e5)*(cos(e1)*cos(e2)*cos(e3) - cos(e1)*sin(e2)*sin(e3)) + cos(e5)*(sin(e1)*sin(e4) + cos(e4)*(cos(e1)*cos(e2)*sin(e3) + cos(e1)*cos(e3)*sin(e2)))) - cos(e6)*(cos(e4)*sin(e1) - sin(e4)*(cos(e1)*cos(e2)*sin(e3) + cos(e1)*cos(e3)*sin(e2))))*(x6*(sin(e2 + e3)*cos(e5) + cos(e2 + e3)*cos(e4)*sin(e5)) - z6*(cos(e6)*(sin(e2 + e3)*sin(e5) - cos(e2 + e3)*cos(e4)*cos(e5)) + cos(e2 + e3)*sin(e4)*sin(e6)) + cos(e4)*cos(e6)*(a1 + d4*cos(e2 + e3) + a3*sin(e2 + e3) + a2*sin(e2)) - cos(e5)*sin(e4)*sin(e6)*(a1 + d4*cos(e2 + e3) + a3*sin(e2 + e3) + a2*sin(e2))) + (cos(e6)*(sin(e5)*(cos(e1)*cos(e2)*cos(e3) - cos(e1)*sin(e2)*sin(e3)) + cos(e5)*(sin(e1)*sin(e4) + cos(e4)*(cos(e1)*cos(e2)*sin(e3) + cos(e1)*cos(e3)*sin(e2)))) + sin(e6)*(cos(e4)*sin(e1) - sin(e4)*(cos(e1)*cos(e2)*sin(e3) + cos(e1)*cos(e3)*sin(e2))))*(y6*(sin(e2 + e3)*cos(e5) + cos(e2 + e3)*cos(e4)*sin(e5)) + z6*(sin(e6)*(sin(e2 + e3)*sin(e5) - cos(e2 + e3)*cos(e4)*cos(e5)) - cos(e2 + e3)*cos(e6)*sin(e4)) - cos(e4)*sin(e6)*(a1 + d4*cos(e2 + e3) + a3*sin(e2 + e3) + a2*sin(e2)) - cos(e5)*cos(e6)*sin(e4)*(a1 + d4*cos(e2 + e3) + a3*sin(e2 + e3) + a2*sin(e2))) - (cos(e5)*(cos(e1)*cos(e2)*cos(e3) - cos(e1)*sin(e2)*sin(e3)) - sin(e5)*(sin(e1)*sin(e4) + cos(e4)*(cos(e1)*cos(e2)*sin(e3) + cos(e1)*cos(e3)*sin(e2))))*(x6*(sin(e6)*(sin(e2 + e3)*sin(e5) - cos(e2 + e3)*cos(e4)*cos(e5)) - cos(e2 + e3)*cos(e6)*sin(e4)) + y6*(cos(e6)*(sin(e2 + e3)*sin(e5) - cos(e2 + e3)*cos(e4)*cos(e5)) + cos(e2 + e3)*sin(e4)*sin(e6)) - sin(e4)*sin(e5)*(a1 + d4*cos(e2 + e3) + a3*sin(e2 + e3) + a2*sin(e2))))*((cos(e5)*(cos(e1)*cos(e2)*cos(e3) - cos(e1)*sin(e2)*sin(e3)) - sin(e5)*(sin(e1)*sin(e4) + cos(e4)*(cos(e1)*cos(e2)*sin(e3) + cos(e1)*cos(e3)*sin(e2))))*(x6*(cos(e2 + e3)*cos(e4)*cos(e6) - cos(e2 + e3)*cos(e5)*sin(e4)*sin(e6)) - y6*(cos(e2 + e3)*cos(e4)*sin(e6) + cos(e2 + e3)*cos(e5)*cos(e6)*sin(e4)) + cos(e4)*sin(e5)*(a1 + d4*cos(e2 + e3) + a3*sin(e2 + e3) + a2*sin(e2))) - (sin(e6)*(sin(e5)*(cos(e1)*cos(e2)*cos(e3) - cos(e1)*sin(e2)*sin(e3)) + cos(e5)*(sin(e1)*sin(e4) + cos(e4)*(cos(e1)*cos(e2)*sin(e3) + cos(e1)*cos(e3)*sin(e2)))) - cos(e6)*(cos(e4)*sin(e1) - sin(e4)*(cos(e1)*cos(e2)*sin(e3) + cos(e1)*cos(e3)*sin(e2))))*(z6*(cos(e2 + e3)*cos(e4)*sin(e6) + cos(e2 + e3)*cos(e5)*cos(e6)*sin(e4)) + cos(e6)*sin(e4)*(a1 + d4*cos(e2 + e3) + a3*sin(e2 + e3) + a2*sin(e2)) + x6*cos(e2 + e3)*sin(e4)*sin(e5) + cos(e4)*cos(e5)*sin(e6)*(a1 + d4*cos(e2 + e3) + a3*sin(e2 + e3) + a2*sin(e2))) - (cos(e6)*(sin(e5)*(cos(e1)*cos(e2)*cos(e3) - cos(e1)*sin(e2)*sin(e3)) + cos(e5)*(sin(e1)*sin(e4) + cos(e4)*(cos(e1)*cos(e2)*sin(e3) + cos(e1)*cos(e3)*sin(e2)))) + sin(e6)*(cos(e4)*sin(e1) - sin(e4)*(cos(e1)*cos(e2)*sin(e3) + cos(e1)*cos(e3)*sin(e2))))*(z6*(cos(e2 + e3)*cos(e4)*cos(e6) - cos(e2 + e3)*cos(e5)*sin(e4)*sin(e6)) - sin(e4)*sin(e6)*(a1 + d4*cos(e2 + e3) + a3*sin(e2 + e3) + a2*sin(e2)) + y6*cos(e2 + e3)*sin(e4)*sin(e5) + cos(e4)*cos(e5)*cos(e6)*(a1 + d4*cos(e2 + e3) + a3*sin(e2 + e3) + a2*sin(e2))) + (cos(e6)*(sin(e1)*sin(e4) + cos(e4)*(cos(e1)*cos(e2)*sin(e3) + cos(e1)*cos(e3)*sin(e2))) + cos(e5)*sin(e6)*(cos(e4)*sin(e1) - sin(e4)*(cos(e1)*cos(e2)*sin(e3) + cos(e1)*cos(e3)*sin(e2))))*(x6*(sin(e2 + e3)*cos(e5) + cos(e2 + e3)*cos(e4)*sin(e5)) - z6*(cos(e6)*(sin(e2 + e3)*sin(e5) - cos(e2 + e3)*cos(e4)*cos(e5)) + cos(e2 + e3)*sin(e4)*sin(e6)) + cos(e4)*cos(e6)*(a1 + d4*cos(e2 + e3) + a3*sin(e2 + e3) + a2*sin(e2)) - cos(e5)*sin(e4)*sin(e6)*(a1 + d4*cos(e2 + e3) + a3*sin(e2 + e3) + a2*sin(e2))) - (sin(e6)*(sin(e1)*sin(e4) + cos(e4)*(cos(e1)*cos(e2)*sin(e3) + cos(e1)*cos(e3)*sin(e2))) - cos(e5)*cos(e6)*(cos(e4)*sin(e1) - sin(e4)*(cos(e1)*cos(e2)*sin(e3) + cos(e1)*cos(e3)*sin(e2))))*(y6*(sin(e2 + e3)*cos(e5) + cos(e2 + e3)*cos(e4)*sin(e5)) + z6*(sin(e6)*(sin(e2 + e3)*sin(e5) - cos(e2 + e3)*cos(e4)*cos(e5)) - cos(e2 + e3)*cos(e6)*sin(e4)) - cos(e4)*sin(e6)*(a1 + d4*cos(e2 + e3) + a3*sin(e2 + e3) + a2*sin(e2)) - cos(e5)*cos(e6)*sin(e4)*(a1 + d4*cos(e2 + e3) + a3*sin(e2 + e3) + a2*sin(e2))) + sin(e5)*(cos(e4)*sin(e1) - sin(e4)*(cos(e1)*cos(e2)*sin(e3) + cos(e1)*cos(e3)*sin(e2)))*(x6*(sin(e6)*(sin(e2 + e3)*sin(e5) - cos(e2 + e3)*cos(e4)*cos(e5)) - cos(e2 + e3)*cos(e6)*sin(e4)) + y6*(cos(e6)*(sin(e2 + e3)*sin(e5) - cos(e2 + e3)*cos(e4)*cos(e5)) + cos(e2 + e3)*sin(e4)*sin(e6)) - sin(e4)*sin(e5)*(a1 + d4*cos(e2 + e3) + a3*sin(e2 + e3) + a2*sin(e2)))) + 2*m5*((cos(e5)*(cos(e2)*sin(e3) + cos(e3)*sin(e2)) - cos(e4)*sin(e5)*(sin(e2)*sin(e3) - cos(e2)*cos(e3)))*(z5*(sin(e2 + e3)*sin(e5) - cos(e2 + e3)*cos(e4)*cos(e5)) + sin(e4)*sin(e5)*(a1 + d4*cos(e2 + e3) + a3*sin(e2 + e3) + a2*sin(e2)) + x5*cos(e2 + e3)*sin(e4)) - (sin(e5)*(cos(e2)*sin(e3) + cos(e3)*sin(e2)) + cos(e4)*cos(e5)*(sin(e2)*sin(e3) - cos(e2)*cos(e3)))*(z5*(sin(e2 + e3)*cos(e5) + cos(e2 + e3)*cos(e4)*sin(e5)) + cos(e5)*sin(e4)*(a1 + d4*cos(e2 + e3) + a3*sin(e2 + e3) + a2*sin(e2)) + y5*cos(e2 + e3)*sin(e4)) + sin(e4)*(sin(e2)*sin(e3) - cos(e2)*cos(e3))*(cos(e4)*(a1 + d4*cos(e2 + e3) + a3*sin(e2 + e3) + a2*sin(e2)) + x5*(sin(e2 + e3)*cos(e5) + cos(e2 + e3)*cos(e4)*sin(e5)) - y5*(sin(e2 + e3)*sin(e5) - cos(e2 + e3)*cos(e4)*cos(e5))))*((cos(e5)*(cos(e2)*sin(e3) + cos(e3)*sin(e2)) - cos(e4)*sin(e5)*(sin(e2)*sin(e3) - cos(e2)*cos(e3)))*(cos(e4)*sin(e5)*(a1 + d4*cos(e2 + e3) + a3*sin(e2 + e3) + a2*sin(e2)) + x5*cos(e2 + e3)*cos(e4) + z5*cos(e2 + e3)*cos(e5)*sin(e4)) - (sin(e5)*(cos(e2)*sin(e3) + cos(e3)*sin(e2)) + cos(e4)*cos(e5)*(sin(e2)*sin(e3) - cos(e2)*cos(e3)))*(y5*cos(e2 + e3)*cos(e4) + cos(e4)*cos(e5)*(a1 + d4*cos(e2 + e3) + a3*sin(e2 + e3) + a2*sin(e2)) - z5*cos(e2 + e3)*sin(e4)*sin(e5)) + cos(e4)*(sin(e2)*sin(e3) - cos(e2)*cos(e3))*(cos(e4)*(a1 + d4*cos(e2 + e3) + a3*sin(e2 + e3) + a2*sin(e2)) + x5*(sin(e2 + e3)*cos(e5) + cos(e2 + e3)*cos(e4)*sin(e5)) - y5*(sin(e2 + e3)*sin(e5) - cos(e2 + e3)*cos(e4)*cos(e5))) - sin(e4)*(sin(e2)*sin(e3) - cos(e2)*cos(e3))*(sin(e4)*(a1 + d4*cos(e2 + e3) + a3*sin(e2 + e3) + a2*sin(e2)) + y5*cos(e2 + e3)*cos(e5)*sin(e4) + x5*cos(e2 + e3)*sin(e4)*sin(e5)) + cos(e5)*sin(e4)*(sin(e2)*sin(e3) - cos(e2)*cos(e3))*(z5*(sin(e2 + e3)*cos(e5) + cos(e2 + e3)*cos(e4)*sin(e5)) + cos(e5)*sin(e4)*(a1 + d4*cos(e2 + e3) + a3*sin(e2 + e3) + a2*sin(e2)) + y5*cos(e2 + e3)*sin(e4)) + sin(e4)*sin(e5)*(sin(e2)*sin(e3) - cos(e2)*cos(e3))*(z5*(sin(e2 + e3)*sin(e5) - cos(e2 + e3)*cos(e4)*cos(e5)) + sin(e4)*sin(e5)*(a1 + d4*cos(e2 + e3) + a3*sin(e2 + e3) + a2*sin(e2)) + x5*cos(e2 + e3)*sin(e4))) - 2*m4*((cos(e4)*sin(e1) - sin(e4)*(cos(e1)*cos(e2)*sin(e3) + cos(e1)*cos(e3)*sin(e2)))*(cos(e4)*(a1 + d4*cos(e2 + e3) + a3*sin(e2 + e3) + a2*sin(e2)) + x4*sin(e2 + e3) + z4*cos(e2 + e3)*cos(e4)) - (y4*cos(e2 + e3)*cos(e4) + x4*cos(e2 + e3)*sin(e4))*(cos(e1)*cos(e2)*cos(e3) - cos(e1)*sin(e2)*sin(e3)) + (sin(e1)*sin(e4) + cos(e4)*(cos(e1)*cos(e2)*sin(e3) + cos(e1)*cos(e3)*sin(e2)))*(sin(e4)*(a1 + d4*cos(e2 + e3) + a3*sin(e2 + e3) + a2*sin(e2)) - y4*sin(e2 + e3) + z4*cos(e2 + e3)*sin(e4)))*((sin(e1)*sin(e4) + cos(e4)*(cos(e1)*cos(e2)*sin(e3) + cos(e1)*cos(e3)*sin(e2)))*(cos(e4)*(a1 + d4*cos(e2 + e3) + a3*sin(e2 + e3) + a2*sin(e2)) + x4*sin(e2 + e3) + z4*cos(e2 + e3)*cos(e4)) + (x4*cos(e2 + e3)*cos(e4) - y4*cos(e2 + e3)*sin(e4))*(cos(e1)*cos(e2)*cos(e3) - cos(e1)*sin(e2)*sin(e3)) - (cos(e4)*sin(e1) - sin(e4)*(cos(e1)*cos(e2)*sin(e3) + cos(e1)*cos(e3)*sin(e2)))*(sin(e4)*(a1 + d4*cos(e2 + e3) + a3*sin(e2 + e3) + a2*sin(e2)) - y4*sin(e2 + e3) + z4*cos(e2 + e3)*sin(e4)) - (sin(e1)*sin(e4) + cos(e4)*(cos(e1)*cos(e2)*sin(e3) + cos(e1)*cos(e3)*sin(e2)))*(cos(e4)*(a1 + d4*cos(e2 + e3) + a3*sin(e2 + e3) + a2*sin(e2)) + z4*cos(e2 + e3)*cos(e4)) + (cos(e4)*sin(e1) - sin(e4)*(cos(e1)*cos(e2)*sin(e3) + cos(e1)*cos(e3)*sin(e2)))*(sin(e4)*(a1 + d4*cos(e2 + e3) + a3*sin(e2 + e3) + a2*sin(e2)) + z4*cos(e2 + e3)*sin(e4))) - cos(e2 + e3)*cos(e4)*(I5xz*(sin(e2 + e3)*sin(e5) - cos(e2 + e3)*cos(e4)*cos(e5)) + I5yz*(sin(e2 + e3)*cos(e5) + cos(e2 + e3)*cos(e4)*sin(e5)) - I5zz*cos(e2 + e3)*sin(e4)) + cos(e2 + e3)*sin(e4)*(I5zz*cos(e2 + e3)*cos(e4) - I5xz*cos(e2 + e3)*cos(e5)*sin(e4) + I5yz*cos(e2 + e3)*sin(e4)*sin(e5)) - cos(e2 + e3)*sin(e4)*sin(e5)*(I6zz*(sin(e2 + e3)*cos(e5) + cos(e2 + e3)*cos(e4)*sin(e5)) + I6xz*(cos(e6)*(sin(e2 + e3)*sin(e5) - cos(e2 + e3)*cos(e4)*cos(e5)) + cos(e2 + e3)*sin(e4)*sin(e6)) - I6yz*(sin(e6)*(sin(e2 + e3)*sin(e5) - cos(e2 + e3)*cos(e4)*cos(e5)) - cos(e2 + e3)*cos(e6)*sin(e4))) + cos(e2 + e3)*cos(e5)*sin(e4)*(I5xx*(sin(e2 + e3)*sin(e5) - cos(e2 + e3)*cos(e4)*cos(e5)) + I5yx*(sin(e2 + e3)*cos(e5) + cos(e2 + e3)*cos(e4)*sin(e5)) - I5zx*cos(e2 + e3)*sin(e4)) - cos(e2 + e3)*sin(e4)*sin(e5)*(I5xy*(sin(e2 + e3)*sin(e5) - cos(e2 + e3)*cos(e4)*cos(e5)) + I5yy*(sin(e2 + e3)*cos(e5) + cos(e2 + e3)*cos(e4)*sin(e5)) - I5zy*cos(e2 + e3)*sin(e4))),de4*((cos(e4)*(I5zz*cos(e2 + e3)*cos(e4) - I5xz*cos(e2 + e3)*cos(e5)*sin(e4) + I5yz*cos(e2 + e3)*sin(e4)*sin(e5)))/2 - ((cos(e6)*sin(e4) + cos(e4)*cos(e5)*sin(e6))*(I6zy*(sin(e2 + e3)*cos(e5) + cos(e2 + e3)*cos(e4)*sin(e5)) + I6xy*(cos(e6)*(sin(e2 + e3)*sin(e5) - cos(e2 + e3)*cos(e4)*cos(e5)) + cos(e2 + e3)*sin(e4)*sin(e6)) - I6yy*(sin(e6)*(sin(e2 + e3)*sin(e5) - cos(e2 + e3)*cos(e4)*cos(e5)) - cos(e2 + e3)*cos(e6)*sin(e4))))/2 - ((sin(e4)*sin(e6) - cos(e4)*cos(e5)*cos(e6))*(I6zx*(sin(e2 + e3)*cos(e5) + cos(e2 + e3)*cos(e4)*sin(e5)) + I6xx*(cos(e6)*(sin(e2 + e3)*sin(e5) - cos(e2 + e3)*cos(e4)*cos(e5)) + cos(e2 + e3)*sin(e4)*sin(e6)) - I6yx*(sin(e6)*(sin(e2 + e3)*sin(e5) - cos(e2 + e3)*cos(e4)*cos(e5)) - cos(e2 + e3)*cos(e6)*sin(e4))))/2 + (sin(e2 + e3)*(I4xz*cos(e4) - I4yz*sin(e4)))/2 + (sin(e4)*(I5xz*(sin(e2 + e3)*sin(e5) - cos(e2 + e3)*cos(e4)*cos(e5)) + I5yz*(sin(e2 + e3)*cos(e5) + cos(e2 + e3)*cos(e4)*sin(e5)) - I5zz*cos(e2 + e3)*sin(e4)))/2 - ((sin(e2 + e3)*cos(e5) + cos(e2 + e3)*cos(e4)*sin(e5))*(I6xz*(sin(e4)*sin(e6) - cos(e4)*cos(e5)*cos(e6)) + I6yz*(cos(e6)*sin(e4) + cos(e4)*cos(e5)*sin(e6)) + I6zz*cos(e4)*sin(e5)))/2 + ((sin(e2 + e3)*sin(e5) - cos(e2 + e3)*cos(e4)*cos(e5))*(I5zx*sin(e4) + I5xx*cos(e4)*cos(e5) - I5yx*cos(e4)*sin(e5)))/2 + ((sin(e2 + e3)*cos(e5) + cos(e2 + e3)*cos(e4)*sin(e5))*(I5zy*sin(e4) + I5xy*cos(e4)*cos(e5) - I5yy*cos(e4)*sin(e5)))/2 - ((cos(e6)*(sin(e2 + e3)*sin(e5) - cos(e2 + e3)*cos(e4)*cos(e5)) + cos(e2 + e3)*sin(e4)*sin(e6))*(I6xx*(sin(e4)*sin(e6) - cos(e4)*cos(e5)*cos(e6)) + I6yx*(cos(e6)*sin(e4) + cos(e4)*cos(e5)*sin(e6)) + I6zx*cos(e4)*sin(e5)))/2 + ((sin(e6)*(sin(e2 + e3)*sin(e5) - cos(e2 + e3)*cos(e4)*cos(e5)) - cos(e2 + e3)*cos(e6)*sin(e4))*(I6xy*(sin(e4)*sin(e6) - cos(e4)*cos(e5)*cos(e6)) + I6yy*(cos(e6)*sin(e4) + cos(e4)*cos(e5)*sin(e6)) + I6zy*cos(e4)*sin(e5)))/2 + (cos(e4)*(I4xy*cos(e2 + e3)*sin(e4) + I4yy*cos(e2 + e3)*cos(e4)))/2 + ((cos(e4)*sin(e6) + cos(e5)*cos(e6)*sin(e4))*(I6xx*(cos(e2 + e3)*cos(e4)*sin(e6) + cos(e2 + e3)*cos(e5)*cos(e6)*sin(e4)) + I6yx*(cos(e2 + e3)*cos(e4)*cos(e6) - cos(e2 + e3)*cos(e5)*sin(e4)*sin(e6)) - I6zx*cos(e2 + e3)*sin(e4)*sin(e5)))/2 + ((cos(e4)*cos(e6) - cos(e5)*sin(e4)*sin(e6))*(I6xy*(cos(e2 + e3)*cos(e4)*sin(e6) + cos(e2 + e3)*cos(e5)*cos(e6)*sin(e4)) + I6yy*(cos(e2 + e3)*cos(e4)*cos(e6) - cos(e2 + e3)*cos(e5)*sin(e4)*sin(e6)) - I6zy*cos(e2 + e3)*sin(e4)*sin(e5)))/2 + (sin(e4)*(I4xx*cos(e2 + e3)*sin(e4) + I4yx*cos(e2 + e3)*cos(e4)))/2 + (cos(e4)*(I4zx*sin(e2 + e3) + I4yx*cos(e2 + e3)*sin(e4) - I4xx*cos(e2 + e3)*cos(e4)))/2 - (sin(e4)*(I4zy*sin(e2 + e3) + I4yy*cos(e2 + e3)*sin(e4) - I4xy*cos(e2 + e3)*cos(e4)))/2 + ((cos(e2 + e3)*cos(e4)*sin(e6) + cos(e2 + e3)*cos(e5)*cos(e6)*sin(e4))*(I6xx*(cos(e4)*sin(e6) + cos(e5)*cos(e6)*sin(e4)) + I6yx*(cos(e4)*cos(e6) - cos(e5)*sin(e4)*sin(e6)) - I6zx*sin(e4)*sin(e5)))/2 + ((cos(e2 + e3)*cos(e4)*cos(e6) - cos(e2 + e3)*cos(e5)*sin(e4)*sin(e6))*(I6xy*(cos(e4)*sin(e6) + cos(e5)*cos(e6)*sin(e4)) + I6yy*(cos(e4)*cos(e6) - cos(e5)*sin(e4)*sin(e6)) - I6zy*sin(e4)*sin(e5)))/2 - (cos(e2 + e3)*cos(e4)*(I4xx*cos(e4) - I4yx*sin(e4)))/2 + (cos(e2 + e3)*cos(e4)*(I4yy*cos(e4) + I4xy*sin(e4)))/2 + m6*((sin(e6)*(sin(e5)*(cos(e2)*sin(e3) + cos(e3)*sin(e2)) + cos(e4)*cos(e5)*(sin(e2)*sin(e3) - cos(e2)*cos(e3))) + cos(e6)*sin(e4)*(sin(e2)*sin(e3) - cos(e2)*cos(e3)))*(x6*(sin(e2 + e3)*cos(e5) + cos(e2 + e3)*cos(e4)*sin(e5)) - z6*(cos(e6)*(sin(e2 + e3)*sin(e5) - cos(e2 + e3)*cos(e4)*cos(e5)) + cos(e2 + e3)*sin(e4)*sin(e6)) + cos(e4)*cos(e6)*(a1 + d4*cos(e2 + e3) + a3*sin(e2 + e3) + a2*sin(e2)) - cos(e5)*sin(e4)*sin(e6)*(a1 + d4*cos(e2 + e3) + a3*sin(e2 + e3) + a2*sin(e2))) + (cos(e6)*(sin(e5)*(cos(e2)*sin(e3) + cos(e3)*sin(e2)) + cos(e4)*cos(e5)*(sin(e2)*sin(e3) - cos(e2)*cos(e3))) - sin(e4)*sin(e6)*(sin(e2)*sin(e3) - cos(e2)*cos(e3)))*(y6*(sin(e2 + e3)*cos(e5) + cos(e2 + e3)*cos(e4)*sin(e5)) + z6*(sin(e6)*(sin(e2 + e3)*sin(e5) - cos(e2 + e3)*cos(e4)*cos(e5)) - cos(e2 + e3)*cos(e6)*sin(e4)) - cos(e4)*sin(e6)*(a1 + d4*cos(e2 + e3) + a3*sin(e2 + e3) + a2*sin(e2)) - cos(e5)*cos(e6)*sin(e4)*(a1 + d4*cos(e2 + e3) + a3*sin(e2 + e3) + a2*sin(e2))) - (cos(e5)*(cos(e2)*sin(e3) + cos(e3)*sin(e2)) - cos(e4)*sin(e5)*(sin(e2)*sin(e3) - cos(e2)*cos(e3)))*(x6*(sin(e6)*(sin(e2 + e3)*sin(e5) - cos(e2 + e3)*cos(e4)*cos(e5)) - cos(e2 + e3)*cos(e6)*sin(e4)) + y6*(cos(e6)*(sin(e2 + e3)*sin(e5) - cos(e2 + e3)*cos(e4)*cos(e5)) + cos(e2 + e3)*sin(e4)*sin(e6)) - sin(e4)*sin(e5)*(a1 + d4*cos(e2 + e3) + a3*sin(e2 + e3) + a2*sin(e2))))*((cos(e4)*sin(e6)*(sin(e2)*sin(e3) - cos(e2)*cos(e3)) + cos(e5)*cos(e6)*sin(e4)*(sin(e2)*sin(e3) - cos(e2)*cos(e3)))*(z6*(cos(e4)*cos(e6) - cos(e5)*sin(e4)*sin(e6)) - cos(e6)*(sin(e5)*(a3 + a2*cos(e3)) - cos(e4)*cos(e5)*(d4 - a2*sin(e3))) - sin(e4)*sin(e6)*(d4 - a2*sin(e3)) + y6*sin(e4)*sin(e5)) - (cos(e4)*cos(e6)*(sin(e2)*sin(e3) - cos(e2)*cos(e3)) - cos(e5)*sin(e4)*sin(e6)*(sin(e2)*sin(e3) - cos(e2)*cos(e3)))*(z6*(cos(e4)*sin(e6) + cos(e5)*cos(e6)*sin(e4)) - sin(e6)*(sin(e5)*(a3 + a2*cos(e3)) - cos(e4)*cos(e5)*(d4 - a2*sin(e3))) + cos(e6)*sin(e4)*(d4 - a2*sin(e3)) + x6*sin(e4)*sin(e5)) - (cos(e5)*(cos(e2)*sin(e3) + cos(e3)*sin(e2)) - cos(e4)*sin(e5)*(sin(e2)*sin(e3) - cos(e2)*cos(e3)))*(x6*(cos(e6)*sin(e4) + cos(e4)*cos(e5)*sin(e6)) - y6*(sin(e4)*sin(e6) - cos(e4)*cos(e5)*cos(e6)) + sin(e4)*sin(e5)*(d4 - a2*sin(e3))) + (sin(e6)*(sin(e5)*(cos(e2)*sin(e3) + cos(e3)*sin(e2)) + cos(e4)*cos(e5)*(sin(e2)*sin(e3) - cos(e2)*cos(e3))) + cos(e6)*sin(e4)*(sin(e2)*sin(e3) - cos(e2)*cos(e3)))*(z6*(sin(e4)*sin(e6) - cos(e4)*cos(e5)*cos(e6)) - cos(e4)*cos(e6)*(d4 - a2*sin(e3)) - x6*cos(e4)*sin(e5) + cos(e5)*sin(e4)*sin(e6)*(d4 - a2*sin(e3))) + (cos(e6)*(sin(e5)*(cos(e2)*sin(e3) + cos(e3)*sin(e2)) + cos(e4)*cos(e5)*(sin(e2)*sin(e3) - cos(e2)*cos(e3))) - sin(e4)*sin(e6)*(sin(e2)*sin(e3) - cos(e2)*cos(e3)))*(z6*(cos(e6)*sin(e4) + cos(e4)*cos(e5)*sin(e6)) + cos(e4)*sin(e6)*(d4 - a2*sin(e3)) - y6*cos(e4)*sin(e5) + cos(e5)*cos(e6)*sin(e4)*(d4 - a2*sin(e3))) + sin(e4)*sin(e5)*(sin(e2)*sin(e3) - cos(e2)*cos(e3))*(cos(e5)*(a3 + a2*cos(e3)) - y6*(cos(e4)*sin(e6) + cos(e5)*cos(e6)*sin(e4)) + x6*(cos(e4)*cos(e6) - cos(e5)*sin(e4)*sin(e6)) + cos(e4)*sin(e5)*(d4 - a2*sin(e3)))) + (cos(e4)*cos(e5)*(I5xx*(sin(e2 + e3)*sin(e5) - cos(e2 + e3)*cos(e4)*cos(e5)) + I5yx*(sin(e2 + e3)*cos(e5) + cos(e2 + e3)*cos(e4)*sin(e5)) - I5zx*cos(e2 + e3)*sin(e4)))/2 - m4*(cos(e4)*(sin(e2)*sin(e3) - cos(e2)*cos(e3))*(cos(e4)*(d4 - a2*sin(e3)) + z4*cos(e4)) - (cos(e2)*sin(e3) + cos(e3)*sin(e2))*(a3 + a2*cos(e3) + x4*cos(e4) - y4*sin(e4)) + sin(e4)*(sin(e2)*sin(e3) - cos(e2)*cos(e3))*(sin(e4)*(d4 - a2*sin(e3)) + z4*sin(e4)))*((cos(e2)*sin(e3) + cos(e3)*sin(e2))*(x4*cos(e2 + e3)*cos(e4) - y4*cos(e2 + e3)*sin(e4)) - cos(e4)*(sin(e2)*sin(e3) - cos(e2)*cos(e3))*(cos(e4)*(a1 + d4*cos(e2 + e3) + a3*sin(e2 + e3) + a2*sin(e2)) + z4*cos(e2 + e3)*cos(e4)) - sin(e4)*(sin(e2)*sin(e3) - cos(e2)*cos(e3))*(sin(e4)*(a1 + d4*cos(e2 + e3) + a3*sin(e2 + e3) + a2*sin(e2)) + z4*cos(e2 + e3)*sin(e4)) + cos(e4)*(sin(e2)*sin(e3) - cos(e2)*cos(e3))*(cos(e4)*(a1 + d4*cos(e2 + e3) + a3*sin(e2 + e3) + a2*sin(e2)) + x4*sin(e2 + e3) + z4*cos(e2 + e3)*cos(e4)) + sin(e4)*(sin(e2)*sin(e3) - cos(e2)*cos(e3))*(sin(e4)*(a1 + d4*cos(e2 + e3) + a3*sin(e2 + e3) + a2*sin(e2)) - y4*sin(e2 + e3) + z4*cos(e2 + e3)*sin(e4))) + (cos(e2 + e3)*sin(e4)*(I4yx*cos(e4) + I4xx*sin(e4)))/2 + (cos(e2 + e3)*sin(e4)*(I4xy*cos(e4) - I4yy*sin(e4)))/2 - (cos(e5)*sin(e4)*(I5zx*cos(e2 + e3)*cos(e4) - I5xx*cos(e2 + e3)*cos(e5)*sin(e4) + I5yx*cos(e2 + e3)*sin(e4)*sin(e5)))/2 - (cos(e4)*sin(e5)*(I5xy*(sin(e2 + e3)*sin(e5) - cos(e2 + e3)*cos(e4)*cos(e5)) + I5yy*(sin(e2 + e3)*cos(e5) + cos(e2 + e3)*cos(e4)*sin(e5)) - I5zy*cos(e2 + e3)*sin(e4)))/2 + (cos(e2 + e3)*cos(e4)*(I5zz*cos(e4) - I5xz*cos(e5)*sin(e4) + I5yz*sin(e4)*sin(e5)))/2 - (cos(e2 + e3)*sin(e4)*(I5zz*sin(e4) + I5xz*cos(e4)*cos(e5) - I5yz*cos(e4)*sin(e5)))/2 + (sin(e4)*sin(e5)*(I5zy*cos(e2 + e3)*cos(e4) - I5xy*cos(e2 + e3)*cos(e5)*sin(e4) + I5yy*cos(e2 + e3)*sin(e4)*sin(e5)))/2 - (sin(e4)*sin(e5)*(I6xz*(cos(e2 + e3)*cos(e4)*sin(e6) + cos(e2 + e3)*cos(e5)*cos(e6)*sin(e4)) + I6yz*(cos(e2 + e3)*cos(e4)*cos(e6) - cos(e2 + e3)*cos(e5)*sin(e4)*sin(e6)) - I6zz*cos(e2 + e3)*sin(e4)*sin(e5)))/2 + m6*((sin(e6)*(sin(e5)*(cos(e2)*cos(e3)*sin(e1) - sin(e1)*sin(e2)*sin(e3)) - cos(e5)*(cos(e1)*sin(e4) - cos(e4)*(cos(e2)*sin(e1)*sin(e3) + cos(e3)*sin(e1)*sin(e2)))) + cos(e6)*(sin(e4)*(cos(e2)*sin(e1)*sin(e3) + cos(e3)*sin(e1)*sin(e2)) + cos(e1)*cos(e4)))*(z6*(cos(e4)*sin(e6) + cos(e5)*cos(e6)*sin(e4)) - sin(e6)*(sin(e5)*(a3 + a2*cos(e3)) - cos(e4)*cos(e5)*(d4 - a2*sin(e3))) + cos(e6)*sin(e4)*(d4 - a2*sin(e3)) + x6*sin(e4)*sin(e5)) + (cos(e6)*(sin(e5)*(cos(e2)*cos(e3)*sin(e1) - sin(e1)*sin(e2)*sin(e3)) - cos(e5)*(cos(e1)*sin(e4) - cos(e4)*(cos(e2)*sin(e1)*sin(e3) + cos(e3)*sin(e1)*sin(e2)))) - sin(e6)*(sin(e4)*(cos(e2)*sin(e1)*sin(e3) + cos(e3)*sin(e1)*sin(e2)) + cos(e1)*cos(e4)))*(z6*(cos(e4)*cos(e6) - cos(e5)*sin(e4)*sin(e6)) - cos(e6)*(sin(e5)*(a3 + a2*cos(e3)) - cos(e4)*cos(e5)*(d4 - a2*sin(e3))) - sin(e4)*sin(e6)*(d4 - a2*sin(e3)) + y6*sin(e4)*sin(e5)) - (cos(e5)*(cos(e2)*cos(e3)*sin(e1) - sin(e1)*sin(e2)*sin(e3)) + sin(e5)*(cos(e1)*sin(e4) - cos(e4)*(cos(e2)*sin(e1)*sin(e3) + cos(e3)*sin(e1)*sin(e2))))*(cos(e5)*(a3 + a2*cos(e3)) - y6*(cos(e4)*sin(e6) + cos(e5)*cos(e6)*sin(e4)) + x6*(cos(e4)*cos(e6) - cos(e5)*sin(e4)*sin(e6)) + cos(e4)*sin(e5)*(d4 - a2*sin(e3))))*((cos(e6)*(cos(e1)*sin(e4) - cos(e4)*(cos(e2)*sin(e1)*sin(e3) + cos(e3)*sin(e1)*sin(e2))) + cos(e5)*sin(e6)*(sin(e4)*(cos(e2)*sin(e1)*sin(e3) + cos(e3)*sin(e1)*sin(e2)) + cos(e1)*cos(e4)))*(x6*(sin(e2 + e3)*cos(e5) + cos(e2 + e3)*cos(e4)*sin(e5)) - z6*(cos(e6)*(sin(e2 + e3)*sin(e5) - cos(e2 + e3)*cos(e4)*cos(e5)) + cos(e2 + e3)*sin(e4)*sin(e6)) + cos(e4)*cos(e6)*(a1 + d4*cos(e2 + e3) + a3*sin(e2 + e3) + a2*sin(e2)) - cos(e5)*sin(e4)*sin(e6)*(a1 + d4*cos(e2 + e3) + a3*sin(e2 + e3) + a2*sin(e2))) - (cos(e5)*(cos(e2)*cos(e3)*sin(e1) - sin(e1)*sin(e2)*sin(e3)) + sin(e5)*(cos(e1)*sin(e4) - cos(e4)*(cos(e2)*sin(e1)*sin(e3) + cos(e3)*sin(e1)*sin(e2))))*(x6*(cos(e2 + e3)*cos(e4)*cos(e6) - cos(e2 + e3)*cos(e5)*sin(e4)*sin(e6)) - y6*(cos(e2 + e3)*cos(e4)*sin(e6) + cos(e2 + e3)*cos(e5)*cos(e6)*sin(e4)) + cos(e4)*sin(e5)*(a1 + d4*cos(e2 + e3) + a3*sin(e2 + e3) + a2*sin(e2))) + (sin(e6)*(sin(e5)*(cos(e2)*cos(e3)*sin(e1) - sin(e1)*sin(e2)*sin(e3)) - cos(e5)*(cos(e1)*sin(e4) - cos(e4)*(cos(e2)*sin(e1)*sin(e3) + cos(e3)*sin(e1)*sin(e2)))) + cos(e6)*(sin(e4)*(cos(e2)*sin(e1)*sin(e3) + cos(e3)*sin(e1)*sin(e2)) + cos(e1)*cos(e4)))*(z6*(cos(e2 + e3)*cos(e4)*sin(e6) + cos(e2 + e3)*cos(e5)*cos(e6)*sin(e4)) + cos(e6)*sin(e4)*(a1 + d4*cos(e2 + e3) + a3*sin(e2 + e3) + a2*sin(e2)) + x6*cos(e2 + e3)*sin(e4)*sin(e5) + cos(e4)*cos(e5)*sin(e6)*(a1 + d4*cos(e2 + e3) + a3*sin(e2 + e3) + a2*sin(e2))) - (sin(e6)*(cos(e1)*sin(e4) - cos(e4)*(cos(e2)*sin(e1)*sin(e3) + cos(e3)*sin(e1)*sin(e2))) - cos(e5)*cos(e6)*(sin(e4)*(cos(e2)*sin(e1)*sin(e3) + cos(e3)*sin(e1)*sin(e2)) + cos(e1)*cos(e4)))*(y6*(sin(e2 + e3)*cos(e5) + cos(e2 + e3)*cos(e4)*sin(e5)) + z6*(sin(e6)*(sin(e2 + e3)*sin(e5) - cos(e2 + e3)*cos(e4)*cos(e5)) - cos(e2 + e3)*cos(e6)*sin(e4)) - cos(e4)*sin(e6)*(a1 + d4*cos(e2 + e3) + a3*sin(e2 + e3) + a2*sin(e2)) - cos(e5)*cos(e6)*sin(e4)*(a1 + d4*cos(e2 + e3) + a3*sin(e2 + e3) + a2*sin(e2))) + (cos(e6)*(sin(e5)*(cos(e2)*cos(e3)*sin(e1) - sin(e1)*sin(e2)*sin(e3)) - cos(e5)*(cos(e1)*sin(e4) - cos(e4)*(cos(e2)*sin(e1)*sin(e3) + cos(e3)*sin(e1)*sin(e2)))) - sin(e6)*(sin(e4)*(cos(e2)*sin(e1)*sin(e3) + cos(e3)*sin(e1)*sin(e2)) + cos(e1)*cos(e4)))*(z6*(cos(e2 + e3)*cos(e4)*cos(e6) - cos(e2 + e3)*cos(e5)*sin(e4)*sin(e6)) - sin(e4)*sin(e6)*(a1 + d4*cos(e2 + e3) + a3*sin(e2 + e3) + a2*sin(e2)) + y6*cos(e2 + e3)*sin(e4)*sin(e5) + cos(e4)*cos(e5)*cos(e6)*(a1 + d4*cos(e2 + e3) + a3*sin(e2 + e3) + a2*sin(e2))) + sin(e5)*(sin(e4)*(cos(e2)*sin(e1)*sin(e3) + cos(e3)*sin(e1)*sin(e2)) + cos(e1)*cos(e4))*(x6*(sin(e6)*(sin(e2 + e3)*sin(e5) - cos(e2 + e3)*cos(e4)*cos(e5)) - cos(e2 + e3)*cos(e6)*sin(e4)) + y6*(cos(e6)*(sin(e2 + e3)*sin(e5) - cos(e2 + e3)*cos(e4)*cos(e5)) + cos(e2 + e3)*sin(e4)*sin(e6)) - sin(e4)*sin(e5)*(a1 + d4*cos(e2 + e3) + a3*sin(e2 + e3) + a2*sin(e2)))) + m5*((cos(e5)*(cos(e2)*sin(e3) + cos(e3)*sin(e2)) - cos(e4)*sin(e5)*(sin(e2)*sin(e3) - cos(e2)*cos(e3)))*(cos(e5)*(a3 + a2*cos(e3)) + x5*cos(e4) + cos(e4)*sin(e5)*(d4 - a2*sin(e3)) + z5*cos(e5)*sin(e4)) + (sin(e5)*(cos(e2)*sin(e3) + cos(e3)*sin(e2)) + cos(e4)*cos(e5)*(sin(e2)*sin(e3) - cos(e2)*cos(e3)))*(sin(e5)*(a3 + a2*cos(e3)) - y5*cos(e4) - cos(e4)*cos(e5)*(d4 - a2*sin(e3)) + z5*sin(e4)*sin(e5)) - sin(e4)*(sin(e2)*sin(e3) - cos(e2)*cos(e3))*(sin(e4)*(d4 - a2*sin(e3)) + y5*cos(e5)*sin(e4) + x5*sin(e4)*sin(e5)))*((cos(e5)*(cos(e2)*sin(e3) + cos(e3)*sin(e2)) - cos(e4)*sin(e5)*(sin(e2)*sin(e3) - cos(e2)*cos(e3)))*(cos(e4)*sin(e5)*(a1 + d4*cos(e2 + e3) + a3*sin(e2 + e3) + a2*sin(e2)) + x5*cos(e2 + e3)*cos(e4) + z5*cos(e2 + e3)*cos(e5)*sin(e4)) - (sin(e5)*(cos(e2)*sin(e3) + cos(e3)*sin(e2)) + cos(e4)*cos(e5)*(sin(e2)*sin(e3) - cos(e2)*cos(e3)))*(y5*cos(e2 + e3)*cos(e4) + cos(e4)*cos(e5)*(a1 + d4*cos(e2 + e3) + a3*sin(e2 + e3) + a2*sin(e2)) - z5*cos(e2 + e3)*sin(e4)*sin(e5)) + cos(e4)*(sin(e2)*sin(e3) - cos(e2)*cos(e3))*(cos(e4)*(a1 + d4*cos(e2 + e3) + a3*sin(e2 + e3) + a2*sin(e2)) + x5*(sin(e2 + e3)*cos(e5) + cos(e2 + e3)*cos(e4)*sin(e5)) - y5*(sin(e2 + e3)*sin(e5) - cos(e2 + e3)*cos(e4)*cos(e5))) - sin(e4)*(sin(e2)*sin(e3) - cos(e2)*cos(e3))*(sin(e4)*(a1 + d4*cos(e2 + e3) + a3*sin(e2 + e3) + a2*sin(e2)) + y5*cos(e2 + e3)*cos(e5)*sin(e4) + x5*cos(e2 + e3)*sin(e4)*sin(e5)) + cos(e5)*sin(e4)*(sin(e2)*sin(e3) - cos(e2)*cos(e3))*(z5*(sin(e2 + e3)*cos(e5) + cos(e2 + e3)*cos(e4)*sin(e5)) + cos(e5)*sin(e4)*(a1 + d4*cos(e2 + e3) + a3*sin(e2 + e3) + a2*sin(e2)) + y5*cos(e2 + e3)*sin(e4)) + sin(e4)*sin(e5)*(sin(e2)*sin(e3) - cos(e2)*cos(e3))*(z5*(sin(e2 + e3)*sin(e5) - cos(e2 + e3)*cos(e4)*cos(e5)) + sin(e4)*sin(e5)*(a1 + d4*cos(e2 + e3) + a3*sin(e2 + e3) + a2*sin(e2)) + x5*cos(e2 + e3)*sin(e4))) + m4*((cos(e4)*sin(e1) - sin(e4)*(cos(e1)*cos(e2)*sin(e3) + cos(e1)*cos(e3)*sin(e2)))*(sin(e4)*(d4 - a2*sin(e3)) + z4*sin(e4)) - (cos(e4)*(d4 - a2*sin(e3)) + z4*cos(e4))*(sin(e1)*sin(e4) + cos(e4)*(cos(e1)*cos(e2)*sin(e3) + cos(e1)*cos(e3)*sin(e2))) + (cos(e1)*cos(e2)*cos(e3) - cos(e1)*sin(e2)*sin(e3))*(a3 + a2*cos(e3) + x4*cos(e4) - y4*sin(e4)))*((sin(e1)*sin(e4) + cos(e4)*(cos(e1)*cos(e2)*sin(e3) + cos(e1)*cos(e3)*sin(e2)))*(cos(e4)*(a1 + d4*cos(e2 + e3) + a3*sin(e2 + e3) + a2*sin(e2)) + x4*sin(e2 + e3) + z4*cos(e2 + e3)*cos(e4)) + (x4*cos(e2 + e3)*cos(e4) - y4*cos(e2 + e3)*sin(e4))*(cos(e1)*cos(e2)*cos(e3) - cos(e1)*sin(e2)*sin(e3)) - (cos(e4)*sin(e1) - sin(e4)*(cos(e1)*cos(e2)*sin(e3) + cos(e1)*cos(e3)*sin(e2)))*(sin(e4)*(a1 + d4*cos(e2 + e3) + a3*sin(e2 + e3) + a2*sin(e2)) - y4*sin(e2 + e3) + z4*cos(e2 + e3)*sin(e4)) - (sin(e1)*sin(e4) + cos(e4)*(cos(e1)*cos(e2)*sin(e3) + cos(e1)*cos(e3)*sin(e2)))*(cos(e4)*(a1 + d4*cos(e2 + e3) + a3*sin(e2 + e3) + a2*sin(e2)) + z4*cos(e2 + e3)*cos(e4)) + (cos(e4)*sin(e1) - sin(e4)*(cos(e1)*cos(e2)*sin(e3) + cos(e1)*cos(e3)*sin(e2)))*(sin(e4)*(a1 + d4*cos(e2 + e3) + a3*sin(e2 + e3) + a2*sin(e2)) + z4*cos(e2 + e3)*sin(e4))) + m5*((cos(e4)*sin(e1) - sin(e4)*(cos(e1)*cos(e2)*sin(e3) + cos(e1)*cos(e3)*sin(e2)))*(cos(e4)*(a1 + d4*cos(e2 + e3) + a3*sin(e2 + e3) + a2*sin(e2)) + x5*(sin(e2 + e3)*cos(e5) + cos(e2 + e3)*cos(e4)*sin(e5)) - y5*(sin(e2 + e3)*sin(e5) - cos(e2 + e3)*cos(e4)*cos(e5))) + (sin(e5)*(cos(e1)*cos(e2)*cos(e3) - cos(e1)*sin(e2)*sin(e3)) + cos(e5)*(sin(e1)*sin(e4) + cos(e4)*(cos(e1)*cos(e2)*sin(e3) + cos(e1)*cos(e3)*sin(e2))))*(z5*(sin(e2 + e3)*cos(e5) + cos(e2 + e3)*cos(e4)*sin(e5)) + cos(e5)*sin(e4)*(a1 + d4*cos(e2 + e3) + a3*sin(e2 + e3) + a2*sin(e2)) + y5*cos(e2 + e3)*sin(e4)) - (cos(e5)*(cos(e1)*cos(e2)*cos(e3) - cos(e1)*sin(e2)*sin(e3)) - sin(e5)*(sin(e1)*sin(e4) + cos(e4)*(cos(e1)*cos(e2)*sin(e3) + cos(e1)*cos(e3)*sin(e2))))*(z5*(sin(e2 + e3)*sin(e5) - cos(e2 + e3)*cos(e4)*cos(e5)) + sin(e4)*sin(e5)*(a1 + d4*cos(e2 + e3) + a3*sin(e2 + e3) + a2*sin(e2)) + x5*cos(e2 + e3)*sin(e4)))*((cos(e5)*(cos(e1)*cos(e2)*cos(e3) - cos(e1)*sin(e2)*sin(e3)) - sin(e5)*(sin(e1)*sin(e4) + cos(e4)*(cos(e1)*cos(e2)*sin(e3) + cos(e1)*cos(e3)*sin(e2))))*(x5*sin(e4) - z5*cos(e4)*cos(e5) + sin(e4)*sin(e5)*(d4 - a2*sin(e3))) - (sin(e5)*(cos(e1)*cos(e2)*cos(e3) - cos(e1)*sin(e2)*sin(e3)) + cos(e5)*(sin(e1)*sin(e4) + cos(e4)*(cos(e1)*cos(e2)*sin(e3) + cos(e1)*cos(e3)*sin(e2))))*(y5*sin(e4) + cos(e5)*sin(e4)*(d4 - a2*sin(e3)) + z5*cos(e4)*sin(e5)) - (cos(e4)*sin(e1) - sin(e4)*(cos(e1)*cos(e2)*sin(e3) + cos(e1)*cos(e3)*sin(e2)))*(cos(e4)*(d4 - a2*sin(e3)) + y5*cos(e4)*cos(e5) + x5*cos(e4)*sin(e5)) + (sin(e1)*sin(e4) + cos(e4)*(cos(e1)*cos(e2)*sin(e3) + cos(e1)*cos(e3)*sin(e2)))*(sin(e4)*(d4 - a2*sin(e3)) + y5*cos(e5)*sin(e4) + x5*sin(e4)*sin(e5)) + sin(e5)*(cos(e4)*sin(e1) - sin(e4)*(cos(e1)*cos(e2)*sin(e3) + cos(e1)*cos(e3)*sin(e2)))*(cos(e5)*(a3 + a2*cos(e3)) + x5*cos(e4) + cos(e4)*sin(e5)*(d4 - a2*sin(e3)) + z5*cos(e5)*sin(e4)) - cos(e5)*(cos(e4)*sin(e1) - sin(e4)*(cos(e1)*cos(e2)*sin(e3) + cos(e1)*cos(e3)*sin(e2)))*(sin(e5)*(a3 + a2*cos(e3)) - y5*cos(e4) - cos(e4)*cos(e5)*(d4 - a2*sin(e3)) + z5*sin(e4)*sin(e5))) + m6*((sin(e6)*(sin(e5)*(cos(e2)*cos(e3)*sin(e1) - sin(e1)*sin(e2)*sin(e3)) - cos(e5)*(cos(e1)*sin(e4) - cos(e4)*(cos(e2)*sin(e1)*sin(e3) + cos(e3)*sin(e1)*sin(e2)))) + cos(e6)*(sin(e4)*(cos(e2)*sin(e1)*sin(e3) + cos(e3)*sin(e1)*sin(e2)) + cos(e1)*cos(e4)))*(x6*(sin(e2 + e3)*cos(e5) + cos(e2 + e3)*cos(e4)*sin(e5)) - z6*(cos(e6)*(sin(e2 + e3)*sin(e5) - cos(e2 + e3)*cos(e4)*cos(e5)) + cos(e2 + e3)*sin(e4)*sin(e6)) + cos(e4)*cos(e6)*(a1 + d4*cos(e2 + e3) + a3*sin(e2 + e3) + a2*sin(e2)) - cos(e5)*sin(e4)*sin(e6)*(a1 + d4*cos(e2 + e3) + a3*sin(e2 + e3) + a2*sin(e2))) + (cos(e6)*(sin(e5)*(cos(e2)*cos(e3)*sin(e1) - sin(e1)*sin(e2)*sin(e3)) - cos(e5)*(cos(e1)*sin(e4) - cos(e4)*(cos(e2)*sin(e1)*sin(e3) + cos(e3)*sin(e1)*sin(e2)))) - sin(e6)*(sin(e4)*(cos(e2)*sin(e1)*sin(e3) + cos(e3)*sin(e1)*sin(e2)) + cos(e1)*cos(e4)))*(y6*(sin(e2 + e3)*cos(e5) + cos(e2 + e3)*cos(e4)*sin(e5)) + z6*(sin(e6)*(sin(e2 + e3)*sin(e5) - cos(e2 + e3)*cos(e4)*cos(e5)) - cos(e2 + e3)*cos(e6)*sin(e4)) - cos(e4)*sin(e6)*(a1 + d4*cos(e2 + e3) + a3*sin(e2 + e3) + a2*sin(e2)) - cos(e5)*cos(e6)*sin(e4)*(a1 + d4*cos(e2 + e3) + a3*sin(e2 + e3) + a2*sin(e2))) - (cos(e5)*(cos(e2)*cos(e3)*sin(e1) - sin(e1)*sin(e2)*sin(e3)) + sin(e5)*(cos(e1)*sin(e4) - cos(e4)*(cos(e2)*sin(e1)*sin(e3) + cos(e3)*sin(e1)*sin(e2))))*(x6*(sin(e6)*(sin(e2 + e3)*sin(e5) - cos(e2 + e3)*cos(e4)*cos(e5)) - cos(e2 + e3)*cos(e6)*sin(e4)) + y6*(cos(e6)*(sin(e2 + e3)*sin(e5) - cos(e2 + e3)*cos(e4)*cos(e5)) + cos(e2 + e3)*sin(e4)*sin(e6)) - sin(e4)*sin(e5)*(a1 + d4*cos(e2 + e3) + a3*sin(e2 + e3) + a2*sin(e2))))*((sin(e6)*(sin(e5)*(cos(e2)*cos(e3)*sin(e1) - sin(e1)*sin(e2)*sin(e3)) - cos(e5)*(cos(e1)*sin(e4) - cos(e4)*(cos(e2)*sin(e1)*sin(e3) + cos(e3)*sin(e1)*sin(e2)))) + cos(e6)*(sin(e4)*(cos(e2)*sin(e1)*sin(e3) + cos(e3)*sin(e1)*sin(e2)) + cos(e1)*cos(e4)))*(z6*(sin(e4)*sin(e6) - cos(e4)*cos(e5)*cos(e6)) - cos(e4)*cos(e6)*(d4 - a2*sin(e3)) - x6*cos(e4)*sin(e5) + cos(e5)*sin(e4)*sin(e6)*(d4 - a2*sin(e3))) + (cos(e6)*(sin(e5)*(cos(e2)*cos(e3)*sin(e1) - sin(e1)*sin(e2)*sin(e3)) - cos(e5)*(cos(e1)*sin(e4) - cos(e4)*(cos(e2)*sin(e1)*sin(e3) + cos(e3)*sin(e1)*sin(e2)))) - sin(e6)*(sin(e4)*(cos(e2)*sin(e1)*sin(e3) + cos(e3)*sin(e1)*sin(e2)) + cos(e1)*cos(e4)))*(z6*(cos(e6)*sin(e4) + cos(e4)*cos(e5)*sin(e6)) + cos(e4)*sin(e6)*(d4 - a2*sin(e3)) - y6*cos(e4)*sin(e5) + cos(e5)*cos(e6)*sin(e4)*(d4 - a2*sin(e3))) - (cos(e5)*(cos(e2)*cos(e3)*sin(e1) - sin(e1)*sin(e2)*sin(e3)) + sin(e5)*(cos(e1)*sin(e4) - cos(e4)*(cos(e2)*sin(e1)*sin(e3) + cos(e3)*sin(e1)*sin(e2))))*(x6*(cos(e6)*sin(e4) + cos(e4)*cos(e5)*sin(e6)) - y6*(sin(e4)*sin(e6) - cos(e4)*cos(e5)*cos(e6)) + sin(e4)*sin(e5)*(d4 - a2*sin(e3))) + (cos(e6)*(cos(e1)*sin(e4) - cos(e4)*(cos(e2)*sin(e1)*sin(e3) + cos(e3)*sin(e1)*sin(e2))) + cos(e5)*sin(e6)*(sin(e4)*(cos(e2)*sin(e1)*sin(e3) + cos(e3)*sin(e1)*sin(e2)) + cos(e1)*cos(e4)))*(z6*(cos(e4)*sin(e6) + cos(e5)*cos(e6)*sin(e4)) - sin(e6)*(sin(e5)*(a3 + a2*cos(e3)) - cos(e4)*cos(e5)*(d4 - a2*sin(e3))) + cos(e6)*sin(e4)*(d4 - a2*sin(e3)) + x6*sin(e4)*sin(e5)) - (sin(e6)*(cos(e1)*sin(e4) - cos(e4)*(cos(e2)*sin(e1)*sin(e3) + cos(e3)*sin(e1)*sin(e2))) - cos(e5)*cos(e6)*(sin(e4)*(cos(e2)*sin(e1)*sin(e3) + cos(e3)*sin(e1)*sin(e2)) + cos(e1)*cos(e4)))*(z6*(cos(e4)*cos(e6) - cos(e5)*sin(e4)*sin(e6)) - cos(e6)*(sin(e5)*(a3 + a2*cos(e3)) - cos(e4)*cos(e5)*(d4 - a2*sin(e3))) - sin(e4)*sin(e6)*(d4 - a2*sin(e3)) + y6*sin(e4)*sin(e5)) + sin(e5)*(sin(e4)*(cos(e2)*sin(e1)*sin(e3) + cos(e3)*sin(e1)*sin(e2)) + cos(e1)*cos(e4))*(cos(e5)*(a3 + a2*cos(e3)) - y6*(cos(e4)*sin(e6) + cos(e5)*cos(e6)*sin(e4)) + x6*(cos(e4)*cos(e6) - cos(e5)*sin(e4)*sin(e6)) + cos(e4)*sin(e5)*(d4 - a2*sin(e3)))) - m5*((cos(e5)*(cos(e2)*cos(e3)*sin(e1) - sin(e1)*sin(e2)*sin(e3)) + sin(e5)*(cos(e1)*sin(e4) - cos(e4)*(cos(e2)*sin(e1)*sin(e3) + cos(e3)*sin(e1)*sin(e2))))*(z5*(sin(e2 + e3)*sin(e5) - cos(e2 + e3)*cos(e4)*cos(e5)) + sin(e4)*sin(e5)*(a1 + d4*cos(e2 + e3) + a3*sin(e2 + e3) + a2*sin(e2)) + x5*cos(e2 + e3)*sin(e4)) + (sin(e4)*(cos(e2)*sin(e1)*sin(e3) + cos(e3)*sin(e1)*sin(e2)) + cos(e1)*cos(e4))*(cos(e4)*(a1 + d4*cos(e2 + e3) + a3*sin(e2 + e3) + a2*sin(e2)) + x5*(sin(e2 + e3)*cos(e5) + cos(e2 + e3)*cos(e4)*sin(e5)) - y5*(sin(e2 + e3)*sin(e5) - cos(e2 + e3)*cos(e4)*cos(e5))) - (sin(e5)*(cos(e2)*cos(e3)*sin(e1) - sin(e1)*sin(e2)*sin(e3)) - cos(e5)*(cos(e1)*sin(e4) - cos(e4)*(cos(e2)*sin(e1)*sin(e3) + cos(e3)*sin(e1)*sin(e2))))*(z5*(sin(e2 